simulink model "ScaraRobotApresentacao2023"  (R2024a)
(part 6 of 10)

et14 = -t2.*t4.*t8.*t9.*t63-t3.*t4.*t7.*t9.*t63-t2.*t4.*t8.*t9.*t68.*2.0-t3.*t4.*t7.*t9.*t68.*2.0-t2.*t4.*t8.*t9.*t69.*2.0-t3.*t4.*t7.*t9.*t69.*2.0+t2.*t4.*t8.*t9.*t70+t3.*t4.*t7.*t9.*t70+t2.*t4.*t8.*t9.*t71+t3.*t4.*t7.*t9.*t71-t2.*t4.*t8.*t9.*t72.*2.0-t3.*t4.*t7.*t9.*t72.*2.0-t2.*t4.*t8.*t9.*t73.*2.0-t3.*t4.*t7.*t9.*t73.*2.0+t2.*t4.*t8.*t9.*t74+t3.*t4.*t7.*t9.*t74+t2.*t4.*t8.*t9.*t75+t3.*t4.*t7.*t9.*t75+t2.*t4.*t8.*t9.*t95+t3.*t4.*t7.*t9.*t95+t2.*t4.*t8.*t9.*t97+t3.*t4.*t7.*t9.*t97+t2.*t4.*t8.*t9.*t101+t3.*t4.*t7.*t9.*t101+t2.*t4.*t8.*t9.*t103+t3.*t4.*t7.*t9.*t103-t3.*t4.*t7.*t9.*t126.*4.0+t3.*t4.*t7.*t9.*t130.*4.0+t3.*t4.*t7.*t9.*t134.*4.0;
et15 = t3.*t4.*t7.*t9.*t136.*4.0-t2.*t4.*t8.*t9.*t142.*2.0-t3.*t4.*t7.*t9.*t142.*2.0-t2.*t4.*t8.*t9.*t143.*2.0-t3.*t4.*t7.*t9.*t143.*2.0-t2.*t4.*t8.*t9.*t144.*2.0-t3.*t4.*t7.*t9.*t144.*2.0-t2.*t4.*t8.*t9.*t145.*2.0-t3.*t4.*t7.*t9.*t145.*2.0-t3.*t4.*t7.*t9.*t148.*4.0-t3.*t4.*t7.*t9.*t150.*4.0-t2.*t4.*t8.*t9.*t154.*2.0-t3.*t4.*t7.*t9.*t154.*2.0-t2.*t4.*t8.*t9.*t155.*2.0-t3.*t4.*t7.*t9.*t155.*2.0-t2.*t4.*t8.*t9.*t156.*2.0-t3.*t4.*t7.*t9.*t156.*2.0-t2.*t4.*t8.*t9.*t157.*2.0-t3.*t4.*t7.*t9.*t157.*2.0+t2.*t4.*t8.*t9.*t160+t3.*t4.*t7.*t9.*t160+t2.*t4.*t8.*t9.*t161+t3.*t4.*t7.*t9.*t161+t2.*t4.*t8.*t9.*t164+t3.*t4.*t7.*t9.*t164+t2.*t4.*t8.*t9.*t165+t3.*t4.*t7.*t9.*t165;
et16 = t2.*t4.*t8.*t9.*t183+t3.*t4.*t7.*t9.*t183+t2.*t4.*t8.*t9.*t184+t3.*t4.*t7.*t9.*t184+t2.*t4.*t8.*t9.*t187+t3.*t4.*t7.*t9.*t187+t2.*t4.*t8.*t9.*t188+t3.*t4.*t7.*t9.*t188+t3.*t4.*t7.*t9.*t239.*4.0-t3.*t4.*t7.*t9.*t243.*4.0+t3.*t4.*t7.*t9.*t246.*2.0-t2.*t4.*t8.*t9.*t250-t3.*t4.*t7.*t9.*t250-t2.*t4.*t8.*t9.*t251-t3.*t4.*t7.*t9.*t251+t3.*t4.*t7.*t9.*t254.*2.0-t2.*t4.*t8.*t9.*t258-t3.*t4.*t7.*t9.*t258-t2.*t4.*t8.*t9.*t259-t3.*t4.*t7.*t9.*t259-t3.*t4.*t7.*t9.*t265.*2.0+t3.*t4.*t7.*t9.*t267.*2.0-t2.*t4.*t8.*t9.*t276-t3.*t4.*t7.*t9.*t276-t2.*t4.*t8.*t9.*t277-t3.*t4.*t7.*t9.*t277-t3.*t4.*t7.*t9.*t278.*2.0;
et17 = t3.*t4.*t7.*t9.*t280.*2.0-t2.*t4.*t8.*t9.*t289-t3.*t4.*t7.*t9.*t289-t2.*t4.*t8.*t9.*t290-t3.*t4.*t7.*t9.*t290+t2.*t4.*t8.*t9.*t336+t3.*t4.*t7.*t9.*t336+t2.*t4.*t8.*t9.*t337+t3.*t4.*t7.*t9.*t337+t2.*t4.*t8.*t9.*t345+t3.*t4.*t7.*t9.*t345+t2.*t4.*t8.*t9.*t346+t3.*t4.*t7.*t9.*t346+t2.*t4.*t8.*t9.*t350+t3.*t4.*t7.*t9.*t350+t2.*t4.*t8.*t9.*t352+t3.*t4.*t7.*t9.*t352+t2.*t4.*t8.*t9.*t355+t3.*t4.*t7.*t9.*t355+t2.*t4.*t8.*t9.*t356+t3.*t4.*t7.*t9.*t356+t3.*t4.*t7.*t9.*t502.*2.0+t3.*t4.*t7.*t9.*t508.*2.0+t3.*t4.*t7.*t9.*t520.*2.0+t3.*t4.*t7.*t9.*t533.*2.0+t2.*t4.*t8.*t9.*t766+t3.*t4.*t7.*t9.*t766+t2.*t4.*t8.*t9.*t767+t3.*t4.*t7.*t9.*t767+t2.*t4.*t8.*t9.*t770+t3.*t4.*t7.*t9.*t770;
et18 = t2.*t4.*t8.*t9.*t771+t3.*t4.*t7.*t9.*t771+t2.*t4.*t8.*t9.*t784+t3.*t4.*t7.*t9.*t784+t2.*t4.*t8.*t9.*t786+t3.*t4.*t7.*t9.*t786+t2.*t4.*t8.*t9.*t787+t3.*t4.*t7.*t9.*t787+t2.*t4.*t8.*t9.*t790+t3.*t4.*t7.*t9.*t790+t2.*t4.*t8.*t9.*t1100+t3.*t4.*t7.*t9.*t1100+t2.*t4.*t8.*t9.*t1101+t3.*t4.*t7.*t9.*t1101+t2.*t4.*t8.*t9.*t1489+t3.*t4.*t7.*t9.*t1489+t2.*t4.*t8.*t9.*t1491+t3.*t4.*t7.*t9.*t1491+t2.*t4.*t8.*t9.*t1492+t3.*t4.*t7.*t9.*t1492+t2.*t4.*t8.*t9.*t1495+t3.*t4.*t7.*t9.*t1495-Lxcm2.^2.*dQ1.*dQ2.*m2.*t37+Lzcm2.^2.*dQ1.*dQ2.*m2.*t37+t2.*t3.*t5.*t9.*t10.*t44.*2.0+t2.*t3.*t5.*t9.*t10.*t45.*2.0+t2.*t3.*t5.*t9.*t10.*t48.*2.0+t2.*t3.*t5.*t9.*t10.*t49.*2.0-t5.*t7.*t8.*t9.*t10.*t44.*2.0+t2.*t3.*t5.*t9.*t10.*t55.*2.0;
et19 = t5.*t7.*t8.*t9.*t10.*t45.*-2.0+t2.*t3.*t5.*t9.*t10.*t56.*2.0-t2.*t5.*t6.*t8.*t11.*t54.*2.0-t3.*t5.*t6.*t7.*t11.*t54.*2.0-t5.*t7.*t8.*t9.*t10.*t48.*2.0-t5.*t7.*t8.*t9.*t10.*t49.*2.0+t2.*t3.*t5.*t9.*t10.*t62.*2.0+t2.*t3.*t5.*t9.*t10.*t63.*2.0-t2.*t5.*t6.*t8.*t11.*t61.*2.0-t3.*t5.*t6.*t7.*t11.*t61.*2.0-t5.*t7.*t8.*t9.*t10.*t55.*2.0-t5.*t7.*t8.*t9.*t10.*t56.*2.0-t2.*t3.*t5.*t9.*t10.*t70.*2.0-t2.*t3.*t5.*t9.*t10.*t71.*2.0-t5.*t7.*t8.*t9.*t10.*t62.*2.0-t5.*t7.*t8.*t9.*t10.*t63.*2.0-t2.*t3.*t5.*t9.*t10.*t74.*2.0-t2.*t3.*t5.*t9.*t10.*t75.*2.0+t5.*t7.*t8.*t9.*t10.*t70.*2.0+t5.*t7.*t8.*t9.*t10.*t71.*2.0-t2.*t4.*t8.*t9.*t36.*t52.*4.0-t3.*t4.*t7.*t9.*t36.*t52.*4.0;
et20 = t2.*t4.*t8.*t9.*t36.*t53.*-4.0-t3.*t4.*t7.*t9.*t36.*t53.*4.0+t5.*t7.*t8.*t9.*t10.*t74.*2.0+t5.*t7.*t8.*t9.*t10.*t75.*2.0-t2.*t4.*t8.*t9.*t36.*t59.*4.0-t3.*t4.*t7.*t9.*t36.*t59.*4.0-t2.*t4.*t8.*t9.*t36.*t60.*4.0-t3.*t4.*t7.*t9.*t36.*t60.*4.0-t2.*t5.*t6.*t8.*t11.*t94.*4.0-t3.*t5.*t6.*t7.*t11.*t94.*4.0-t2.*t4.*t8.*t9.*t35.*t70.*2.0-t2.*t5.*t6.*t8.*t11.*t96.*4.0-t3.*t4.*t7.*t9.*t35.*t70.*2.0-t3.*t5.*t6.*t7.*t11.*t96.*4.0-t2.*t4.*t8.*t9.*t35.*t71.*2.0-t3.*t4.*t7.*t9.*t35.*t71.*2.0-t2.*t4.*t8.*t9.*t35.*t74.*2.0-t2.*t5.*t6.*t8.*t11.*t100.*4.0-t3.*t4.*t7.*t9.*t35.*t74.*2.0-t3.*t5.*t6.*t7.*t11.*t100.*4.0-t2.*t4.*t8.*t9.*t35.*t75.*2.0-t3.*t4.*t7.*t9.*t35.*t75.*2.0;
et21 = t2.*t5.*t6.*t8.*t11.*t102.*-4.0-t3.*t5.*t6.*t7.*t11.*t102.*4.0-t2.*t4.*t8.*t9.*t36.*t95.*2.0-t3.*t4.*t7.*t9.*t36.*t95.*2.0-t2.*t4.*t8.*t9.*t36.*t97.*2.0-t3.*t4.*t7.*t9.*t36.*t97.*2.0-t2.*t4.*t8.*t9.*t36.*t101.*2.0-t3.*t4.*t7.*t9.*t36.*t101.*2.0-t2.*t4.*t8.*t9.*t36.*t103.*2.0-t3.*t4.*t7.*t9.*t36.*t103.*2.0+t3.*t5.*t6.*t7.*t11.*t130.*4.0-t2.*t5.*t6.*t8.*t11.*t132.*2.0-t3.*t5.*t6.*t7.*t11.*t132.*2.0-t3.*t5.*t6.*t7.*t11.*t138.*4.0+t2.*t5.*t6.*t8.*t11.*t140.*2.0+t3.*t5.*t6.*t7.*t11.*t140.*2.0-t3.*t4.*t7.*t9.*t35.*t128.*4.0-t3.*t4.*t7.*t9.*t36.*t130.*4.0-t3.*t4.*t7.*t9.*t35.*t138.*4.0+t3.*t4.*t7.*t9.*t36.*t138.*4.0+t3.*t4.*t7.*t9.*t35.*t148.*4.0+t3.*t4.*t7.*t9.*t35.*t150.*4.0+t5.*t7.*t8.*t9.*t10.*t222.*4.0;
et22 = t5.*t7.*t8.*t9.*t10.*t225.*4.0-t3.*t4.*t7.*t9.*t36.*t239.*8.0-t3.*t5.*t6.*t7.*t11.*t267.*4.0+t3.*t4.*t7.*t9.*t36.*t243.*8.0+t2.*t5.*t6.*t8.*t11.*t271.*2.0+t3.*t5.*t6.*t7.*t11.*t271.*2.0+t2.*t5.*t6.*t8.*t11.*t272.*2.0+t3.*t5.*t6.*t7.*t11.*t272.*2.0-t3.*t5.*t6.*t7.*t11.*t280.*4.0+t2.*t5.*t6.*t8.*t11.*t284.*2.0+t3.*t5.*t6.*t7.*t11.*t284.*2.0+t2.*t5.*t6.*t8.*t11.*t285.*2.0+t3.*t5.*t6.*t7.*t11.*t285.*2.0-t3.*t4.*t7.*t9.*t36.*t267.*4.0-t3.*t4.*t7.*t9.*t36.*t280.*4.0+t5.*t7.*t8.*t9.*t10.*t485.*4.0+t5.*t7.*t8.*t9.*t10.*t486.*4.0-t5.*t7.*t8.*t9.*t10.*t501.*4.0-t5.*t7.*t8.*t9.*t10.*t507.*4.0-t3.*t5.*t6.*t7.*t11.*t515.*8.0-t3.*t5.*t6.*t7.*t11.*t528.*8.0-t3.*t5.*t6.*t7.*t11.*t978.*4.0-t3.*t5.*t6.*t7.*t11.*t984.*4.0;
et23 = Lx2.*Lx3.*dQ1.*dQ2.*m4.*t8.*2.0+Lx2.*Lx3.*dQ1.*dQ2.*m5.*t8.*2.0+Lx2.*Lx3.*dQ1.*dQ2.*m6.*t8.*2.0+Lx2.*Lxcm3.*dQ1.*dQ2.*m3.*t8.*2.0-Lx3.*Lxcm4.*dQ1.*dQ4.*m4.*t9.*2.0-Lx3.*Lxcm5.*dQ1.*dQ2.*m5.*t10.*2.0-Lx3.*Lxcm5.*dQ1.*dQ3.*m5.*t10.*2.0-Lx3.*Lycm4.*dQ1.*dQ4.*m4.*t4.*2.0-Lx3.*Lycm5.*dQ1.*dQ4.*m5.*t4.*2.0-Lxcm4.*Lycm4.*dQ1.*dQ4.*m4.*t32.*2.0-Lxcm4.*Lycm4.*dQ1.*dQ4.*m4.*t33.*2.0+Lxcm6.*Lycm6.*dQ1.*dQ6.*m6.*t32.*4.0+Lxcm6.*Lycm6.*dQ1.*dQ6.*m6.*t33.*4.0+Lxcm6.*Lycm6.*dQ1.*dQ6.*m6.*t35.*2.0+Lxcm6.*Lycm6.*dQ1.*dQ6.*m6.*t36.*4.0-Lx2.*Lz4.*dQ1.*dQ2.*m5.*t3.*2.0-Lx2.*Lz4.*dQ1.*dQ2.*m6.*t3.*2.0+Lx3.*Lz5.*dQ1.*dQ2.*m6.*t5.*2.0+Lx3.*Lz5.*dQ1.*dQ3.*m6.*t5.*2.0-Lx3.*Lz4.*dQ1.*dQ2.*m5.*t32.*4.0-Lx3.*Lz4.*dQ1.*dQ2.*m5.*t33.*4.0-Lx3.*Lz4.*dQ1.*dQ2.*m6.*t32.*4.0-Lx3.*Lz4.*dQ1.*dQ3.*m5.*t32.*4.0;
et24 = Lx3.*Lz4.*dQ1.*dQ2.*m6.*t33.*-4.0-Lx3.*Lz4.*dQ1.*dQ3.*m5.*t33.*4.0-Lx3.*Lz4.*dQ1.*dQ3.*m6.*t32.*4.0-Lx3.*Lz4.*dQ1.*dQ3.*m6.*t33.*4.0-Lx2.*Lzcm3.*dQ1.*dQ2.*m3.*t3.*2.0-Lx2.*Lzcm4.*dQ1.*dQ2.*m4.*t3.*2.0+Lx3.*Lzcm5.*dQ1.*dQ2.*m5.*t5.*2.0+Lx3.*Lzcm5.*dQ1.*dQ3.*m5.*t5.*2.0+Lx3.*Lzcm6.*dQ1.*dQ2.*m6.*t5.*2.0+Lx3.*Lzcm6.*dQ1.*dQ3.*m6.*t5.*2.0-Lxcm6.*Lz5.*dQ1.*dQ5.*m6.*t6.*2.0-Lx3.*Lzcm4.*dQ1.*dQ2.*m4.*t32.*4.0-Lx3.*Lzcm4.*dQ1.*dQ2.*m4.*t33.*4.0-Lx3.*Lzcm4.*dQ1.*dQ3.*m4.*t32.*4.0-Lx3.*Lzcm4.*dQ1.*dQ3.*m4.*t33.*4.0+Lxcm4.*Lzcm4.*dQ1.*dQ2.*m4.*t4.*2.0+Lxcm4.*Lzcm4.*dQ1.*dQ3.*m4.*t4.*2.0-Lxcm5.*Lzcm5.*dQ1.*dQ2.*m5.*t4.*2.0-Lxcm5.*Lzcm5.*dQ1.*dQ3.*m5.*t4.*2.0-Lxcm6.*Lzcm6.*dQ1.*dQ5.*m6.*t6.*2.0+Lxcm2.*Lzcm2.*dQ1.*dQ2.*m2.*t32.*4.0-Lxcm3.*Lzcm3.*dQ1.*dQ2.*m3.*t32.*4.0-Lxcm3.*Lzcm3.*dQ1.*dQ2.*m3.*t33.*4.0;
et25 = Lxcm3.*Lzcm3.*dQ1.*dQ3.*m3.*t32.*-4.0-Lxcm3.*Lzcm3.*dQ1.*dQ3.*m3.*t33.*4.0+Lxcm5.*Lzcm5.*dQ1.*dQ5.*m5.*t32.*2.0+Lxcm5.*Lzcm5.*dQ1.*dQ5.*m5.*t33.*2.0+Lxcm5.*Lzcm5.*dQ1.*dQ5.*m5.*t35.*4.0-Lycm5.*Lz4.*dQ1.*dQ2.*m5.*t9.*2.0-Lycm5.*Lz4.*dQ1.*dQ3.*m5.*t9.*2.0+Lycm6.*Lz5.*dQ1.*dQ5.*m6.*t11.*2.0-Lycm4.*Lzcm4.*dQ1.*dQ2.*m4.*t9.*2.0-Lycm4.*Lzcm4.*dQ1.*dQ3.*m4.*t9.*2.0+Lycm6.*Lzcm6.*dQ1.*dQ5.*m6.*t11.*2.0+Lz5.*Lzcm6.*dQ1.*dQ5.*m6.*t40.*2.0+Ixx5.*dQ1.*dQ5.*t2.*t4.*t7.*2.0+Ixx5.*dQ1.*dQ5.*t3.*t4.*t8.*2.0+Ixx5.*dQ2.*dQ5.*t2.*t3.*t9+Ixx5.*dQ1.*dQ2.*t4.*t5.*t10.*2.0+Ixx5.*dQ3.*dQ5.*t2.*t3.*t9+Ixx6.*dQ2.*dQ5.*t2.*t3.*t9+Ixx5.*dQ1.*dQ3.*t4.*t5.*t10.*2.0-Ixx5.*dQ4.*dQ5.*t2.*t4.*t8-Ixx5.*dQ4.*dQ5.*t3.*t4.*t7+Ixx6.*dQ3.*dQ5.*t2.*t3.*t9-Ixx6.*dQ2.*dQ6.*t2.*t5.*t8-Ixx6.*dQ2.*dQ6.*t3.*t5.*t7;
et26 = Ixx6.*dQ4.*dQ5.*t2.*t4.*t8+Ixx6.*dQ4.*dQ5.*t3.*t4.*t7-Ixx6.*dQ3.*dQ6.*t2.*t5.*t8-Ixx6.*dQ3.*dQ6.*t3.*t5.*t7+Ixx6.*dQ5.*dQ6.*t2.*t3.*t10-Ixx5.*dQ2.*dQ5.*t7.*t8.*t9-Ixx5.*dQ3.*dQ5.*t7.*t8.*t9-Ixx6.*dQ2.*dQ5.*t7.*t8.*t9-Ixx6.*dQ3.*dQ5.*t7.*t8.*t9-Ixx6.*dQ5.*dQ6.*t7.*t8.*t10+Ixx3.*dQ1.*dQ2.*t2.*t7.*t33.*4.0+Ixx3.*dQ1.*dQ2.*t3.*t8.*t32.*4.0+Ixx3.*dQ1.*dQ3.*t2.*t7.*t33.*4.0+Ixx3.*dQ1.*dQ3.*t3.*t8.*t32.*4.0-Ixx4.*dQ1.*dQ2.*t2.*t7.*t34.*2.0-Ixx5.*dQ1.*dQ2.*t2.*t7.*t33.*4.0-Ixx4.*dQ1.*dQ3.*t2.*t7.*t34.*2.0-Ixx5.*dQ1.*dQ2.*t3.*t8.*t32.*4.0-Ixx5.*dQ1.*dQ3.*t2.*t7.*t33.*4.0+Ixx6.*dQ1.*dQ2.*t2.*t7.*t33.*4.0-Ixx4.*dQ1.*dQ2.*t3.*t8.*t34.*2.0-Ixx5.*dQ1.*dQ2.*t2.*t7.*t35.*2.0-Ixx5.*dQ1.*dQ3.*t3.*t8.*t32.*4.0;
et27 = Ixx6.*dQ1.*dQ2.*t2.*t7.*t34.*2.0+Ixx6.*dQ1.*dQ2.*t3.*t8.*t32.*4.0+Ixx6.*dQ1.*dQ3.*t2.*t7.*t33.*4.0-Ixx4.*dQ1.*dQ3.*t3.*t8.*t34.*2.0-Ixx5.*dQ1.*dQ3.*t2.*t7.*t35.*2.0+Ixx6.*dQ1.*dQ3.*t2.*t7.*t34.*2.0+Ixx6.*dQ1.*dQ3.*t3.*t8.*t32.*4.0-Ixx4.*dQ1.*dQ4.*t4.*t9.*t32.*2.0-Ixx4.*dQ2.*dQ4.*t2.*t8.*t34.*2.0-Ixx4.*dQ2.*dQ4.*t3.*t7.*t34.*2.0-Ixx5.*dQ1.*dQ2.*t3.*t8.*t35.*2.0+Ixx6.*dQ1.*dQ2.*t2.*t7.*t36.*4.0+Ixx6.*dQ1.*dQ2.*t3.*t8.*t34.*2.0-Ixx4.*dQ1.*dQ4.*t4.*t9.*t33.*2.0-Ixx4.*dQ3.*dQ4.*t2.*t8.*t34.*2.0-Ixx4.*dQ3.*dQ4.*t3.*t7.*t34.*2.0-Ixx5.*dQ1.*dQ3.*t3.*t8.*t35.*2.0+Ixx6.*dQ1.*dQ3.*t2.*t7.*t36.*4.0+Ixx6.*dQ1.*dQ3.*t3.*t8.*t34.*2.0+Ixx5.*dQ2.*dQ4.*t2.*t8.*t35.*2.0+Ixx5.*dQ2.*dQ4.*t3.*t7.*t35.*2.0+Ixx6.*dQ1.*dQ2.*t3.*t8.*t36.*4.0+Ixx6.*dQ1.*dQ4.*t4.*t9.*t32.*2.0;
et28 = Ixx6.*dQ2.*dQ4.*t2.*t8.*t34.*2.0+Ixx6.*dQ2.*dQ4.*t3.*t7.*t34.*2.0+Ixx5.*dQ3.*dQ4.*t2.*t8.*t35.*2.0+Ixx5.*dQ3.*dQ4.*t3.*t7.*t35.*2.0+Ixx6.*dQ1.*dQ3.*t3.*t8.*t36.*4.0+Ixx6.*dQ1.*dQ4.*t4.*t9.*t33.*2.0+Ixx6.*dQ3.*dQ4.*t2.*t8.*t34.*2.0+Ixx6.*dQ3.*dQ4.*t3.*t7.*t34.*2.0-Ixx5.*dQ1.*dQ5.*t5.*t10.*t32.*2.0-Ixx5.*dQ1.*dQ5.*t5.*t10.*t33.*2.0+Ixx6.*dQ1.*dQ6.*t6.*t11.*t32.*4.0+Ixx6.*dQ1.*dQ5.*t5.*t10.*t36.*2.0+Ixx6.*dQ1.*dQ6.*t6.*t11.*t33.*4.0+Ixx6.*dQ1.*dQ6.*t6.*t11.*t35.*2.0-Ixy5.*dQ2.*dQ3.*t2.*t3.*t5+Ixy6.*dQ2.*dQ3.*t2.*t3.*t5+Ixy5.*dQ2.*dQ3.*t5.*t7.*t8-Ixy6.*dQ2.*dQ3.*t5.*t7.*t8+Ixy6.*dQ5.*dQ6.*t2.*t8.*t9+Ixy6.*dQ5.*dQ6.*t3.*t7.*t9+Ixy4.*dQ2.*dQ3.*t2.*t3.*t34.*2.0+Ixy6.*dQ4.*dQ6.*t2.*t3.*t35+Ixy6.*dQ4.*dQ6.*t2.*t3.*t36.*2.0-Ixy4.*dQ2.*dQ3.*t7.*t8.*t34.*2.0;
et29 = Ixy5.*dQ1.*dQ2.*t9.*t10.*t32.*-2.0-Ixy5.*dQ1.*dQ2.*t9.*t10.*t33.*2.0-Ixy5.*dQ1.*dQ3.*t9.*t10.*t32.*2.0+Ixy6.*dQ1.*dQ2.*t9.*t10.*t32.*2.0-Ixy5.*dQ1.*dQ3.*t9.*t10.*t33.*2.0+Ixy6.*dQ1.*dQ2.*t9.*t10.*t33.*2.0+Ixy6.*dQ1.*dQ3.*t9.*t10.*t32.*2.0+Ixy6.*dQ1.*dQ3.*t9.*t10.*t33.*2.0+Ixy6.*dQ1.*dQ2.*t9.*t10.*t36.*2.0+Ixy6.*dQ1.*dQ3.*t9.*t10.*t36.*2.0-Ixy6.*dQ4.*dQ6.*t7.*t8.*t35-Ixy6.*dQ4.*dQ6.*t7.*t8.*t36.*2.0+Ixy5.*dQ1.*dQ4.*t5.*t32.*t33.*2.0+Ixy5.*dQ1.*dQ4.*t5.*t32.*t34.*2.0-Ixy6.*dQ1.*dQ4.*t5.*t32.*t33.*2.0+Ixy5.*dQ1.*dQ4.*t5.*t33.*t34.*2.0-Ixy6.*dQ1.*dQ4.*t5.*t32.*t34.*2.0-Ixy6.*dQ1.*dQ4.*t5.*t33.*t34.*2.0-Ixy6.*dQ1.*dQ4.*t5.*t32.*t36.*2.0-Ixy6.*dQ1.*dQ4.*t5.*t33.*t36.*2.0-Ixy4.*dQ1.*dQ4.*t32.*t33.*t34.*4.0+Ixy6.*dQ1.*dQ6.*t32.*t33.*t34.*2.0+Ixy6.*dQ1.*dQ6.*t32.*t33.*t35.*2.0;
et30 = Ixy6.*dQ1.*dQ6.*t32.*t33.*t36.*8.0-Ixy6.*dQ1.*dQ6.*t32.*t34.*t35+Ixy6.*dQ1.*dQ6.*t32.*t34.*t36.*2.0-Ixy6.*dQ1.*dQ6.*t33.*t34.*t35+Ixy6.*dQ1.*dQ6.*t32.*t35.*t36.*2.0+Ixy6.*dQ1.*dQ6.*t33.*t34.*t36.*2.0+Ixy6.*dQ1.*dQ6.*t33.*t35.*t36.*2.0-Ixz6.*dQ4.*dQ5.*t2.*t3.*t6+Ixz4.*dQ1.*dQ4.*t2.*t7.*t9+Ixz4.*dQ2.*dQ3.*t2.*t8.*t9+Ixz4.*dQ2.*dQ3.*t3.*t7.*t9-Ixz5.*dQ1.*dQ4.*t2.*t7.*t9+Ixz4.*dQ1.*dQ4.*t3.*t8.*t9-Ixz5.*dQ2.*dQ3.*t2.*t8.*t9-Ixz5.*dQ2.*dQ3.*t3.*t7.*t9-Ixz5.*dQ1.*dQ4.*t3.*t8.*t9-Ixz6.*dQ1.*dQ2.*t5.*t9.*t11-Ixz6.*dQ1.*dQ3.*t5.*t9.*t11+Ixz6.*dQ4.*dQ5.*t6.*t7.*t8-Ixz6.*dQ1.*dQ6.*t5.*t10.*t11+Ixz6.*dQ1.*dQ2.*t4.*t6.*t32.*2.0+Ixz6.*dQ1.*dQ2.*t4.*t6.*t33.*2.0+Ixz6.*dQ1.*dQ3.*t4.*t6.*t32.*2.0+Ixz6.*dQ1.*dQ3.*t4.*t6.*t33.*2.0;
et31 = Ixz5.*dQ4.*dQ5.*t2.*t3.*t35.*2.0+Ixz6.*dQ1.*dQ2.*t4.*t6.*t35.*2.0+Ixz6.*dQ1.*dQ3.*t4.*t6.*t35.*2.0-Ixz5.*dQ4.*dQ5.*t7.*t8.*t35.*2.0-Ixz6.*dQ1.*dQ4.*t10.*t11.*t32-Ixz6.*dQ1.*dQ4.*t10.*t11.*t33+Ixz4.*dQ1.*dQ2.*t4.*t32.*t33.*4.0+Ixz4.*dQ1.*dQ3.*t4.*t32.*t33.*4.0-Ixz5.*dQ1.*dQ2.*t4.*t32.*t33.*4.0-Ixz5.*dQ1.*dQ3.*t4.*t32.*t33.*4.0-Ixz5.*dQ1.*dQ2.*t4.*t32.*t35.*4.0-Ixz5.*dQ1.*dQ2.*t4.*t33.*t35.*4.0-Ixz5.*dQ1.*dQ3.*t4.*t32.*t35.*4.0-Ixz5.*dQ1.*dQ3.*t4.*t33.*t35.*4.0-Ixz6.*dQ1.*dQ5.*t6.*t32.*t33.*2.0+Ixz6.*dQ1.*dQ5.*t6.*t32.*t34-Ixz6.*dQ1.*dQ5.*t6.*t32.*t35.*2.0+Ixz6.*dQ1.*dQ5.*t6.*t33.*t34-Ixz6.*dQ1.*dQ5.*t6.*t33.*t35.*2.0-Ixz5.*dQ1.*dQ5.*t32.*t33.*t34.*2.0+Ixz5.*dQ1.*dQ5.*t32.*t33.*t35.*4.0-Ixz5.*dQ1.*dQ5.*t32.*t34.*t35.*2.0-Ixz5.*dQ1.*dQ5.*t33.*t34.*t35.*2.0;
et32 = -Iyx5.*dQ2.*dQ3.*t2.*t3.*t5+Iyx6.*dQ2.*dQ3.*t2.*t3.*t5+Iyx5.*dQ2.*dQ3.*t5.*t7.*t8-Iyx6.*dQ2.*dQ3.*t5.*t7.*t8+Iyx6.*dQ5.*dQ6.*t2.*t8.*t9+Iyx6.*dQ5.*dQ6.*t3.*t7.*t9+Iyx4.*dQ2.*dQ3.*t2.*t3.*t34.*2.0+Iyx6.*dQ4.*dQ6.*t2.*t3.*t35+Iyx6.*dQ4.*dQ6.*t2.*t3.*t36.*2.0-Iyx4.*dQ2.*dQ3.*t7.*t8.*t34.*2.0-Iyx5.*dQ1.*dQ2.*t9.*t10.*t32.*2.0-Iyx5.*dQ1.*dQ2.*t9.*t10.*t33.*2.0-Iyx5.*dQ1.*dQ3.*t9.*t10.*t32.*2.0+Iyx6.*dQ1.*dQ2.*t9.*t10.*t32.*2.0-Iyx5.*dQ1.*dQ3.*t9.*t10.*t33.*2.0+Iyx6.*dQ1.*dQ2.*t9.*t10.*t33.*2.0+Iyx6.*dQ1.*dQ3.*t9.*t10.*t32.*2.0+Iyx6.*dQ1.*dQ3.*t9.*t10.*t33.*2.0+Iyx6.*dQ1.*dQ2.*t9.*t10.*t36.*2.0+Iyx6.*dQ1.*dQ3.*t9.*t10.*t36.*2.0-Iyx6.*dQ4.*dQ6.*t7.*t8.*t35-Iyx6.*dQ4.*dQ6.*t7.*t8.*t36.*2.0+Iyx5.*dQ1.*dQ4.*t5.*t32.*t33.*2.0+Iyx5.*dQ1.*dQ4.*t5.*t32.*t34.*2.0;
et33 = Iyx6.*dQ1.*dQ4.*t5.*t32.*t33.*-2.0+Iyx5.*dQ1.*dQ4.*t5.*t33.*t34.*2.0-Iyx6.*dQ1.*dQ4.*t5.*t32.*t34.*2.0-Iyx6.*dQ1.*dQ4.*t5.*t33.*t34.*2.0-Iyx6.*dQ1.*dQ4.*t5.*t32.*t36.*2.0-Iyx6.*dQ1.*dQ4.*t5.*t33.*t36.*2.0-Iyx4.*dQ1.*dQ4.*t32.*t33.*t34.*4.0+Iyx6.*dQ1.*dQ6.*t32.*t33.*t34.*2.0+Iyx6.*dQ1.*dQ6.*t32.*t33.*t35.*2.0+Iyx6.*dQ1.*dQ6.*t32.*t33.*t36.*8.0-Iyx6.*dQ1.*dQ6.*t32.*t34.*t35+Iyx6.*dQ1.*dQ6.*t32.*t34.*t36.*2.0-Iyx6.*dQ1.*dQ6.*t33.*t34.*t35+Iyx6.*dQ1.*dQ6.*t32.*t35.*t36.*2.0+Iyx6.*dQ1.*dQ6.*t33.*t34.*t36.*2.0+Iyx6.*dQ1.*dQ6.*t33.*t35.*t36.*2.0+Iyy6.*dQ1.*dQ5.*t2.*t4.*t7.*2.0+Iyy5.*dQ2.*dQ5.*t2.*t3.*t9+Iyy5.*dQ3.*dQ5.*t2.*t3.*t9+Iyy6.*dQ1.*dQ5.*t3.*t4.*t8.*2.0+Iyy6.*dQ2.*dQ5.*t2.*t3.*t9+Iyy5.*dQ4.*dQ5.*t2.*t4.*t8+Iyy5.*dQ4.*dQ5.*t3.*t4.*t7+Iyy6.*dQ1.*dQ2.*t4.*t5.*t10.*2.0;
et34 = Iyy6.*dQ3.*dQ5.*t2.*t3.*t9+Iyy6.*dQ1.*dQ3.*t4.*t5.*t10.*2.0+Iyy6.*dQ2.*dQ6.*t2.*t5.*t8+Iyy6.*dQ2.*dQ6.*t3.*t5.*t7-Iyy6.*dQ4.*dQ5.*t2.*t4.*t8-Iyy6.*dQ4.*dQ5.*t3.*t4.*t7+Iyy6.*dQ3.*dQ6.*t2.*t5.*t8+Iyy6.*dQ3.*dQ6.*t3.*t5.*t7-Iyy6.*dQ5.*dQ6.*t2.*t3.*t10-Iyy5.*dQ2.*dQ5.*t7.*t8.*t9-Iyy5.*dQ3.*dQ5.*t7.*t8.*t9-Iyy6.*dQ2.*dQ5.*t7.*t8.*t9-Iyy6.*dQ3.*dQ5.*t7.*t8.*t9+Iyy6.*dQ5.*dQ6.*t7.*t8.*t10+Iyy4.*dQ1.*dQ2.*t2.*t7.*t33.*4.0+Iyy4.*dQ1.*dQ2.*t2.*t7.*t34.*2.0+Iyy4.*dQ1.*dQ2.*t3.*t8.*t32.*4.0+Iyy4.*dQ1.*dQ3.*t2.*t7.*t33.*4.0+Iyy5.*dQ1.*dQ2.*t2.*t7.*t33.*4.0+Iyy4.*dQ1.*dQ3.*t2.*t7.*t34.*2.0+Iyy4.*dQ1.*dQ3.*t3.*t8.*t32.*4.0+Iyy5.*dQ1.*dQ2.*t2.*t7.*t34.*2.0+Iyy5.*dQ1.*dQ2.*t3.*t8.*t32.*4.0+Iyy5.*dQ1.*dQ3.*t2.*t7.*t33.*4.0;
et35 = Iyy6.*dQ1.*dQ2.*t2.*t7.*t33.*-4.0+Iyy4.*dQ1.*dQ2.*t3.*t8.*t34.*2.0+Iyy5.*dQ1.*dQ3.*t2.*t7.*t34.*2.0+Iyy5.*dQ1.*dQ3.*t3.*t8.*t32.*4.0-Iyy6.*dQ1.*dQ2.*t3.*t8.*t32.*4.0-Iyy6.*dQ1.*dQ3.*t2.*t7.*t33.*4.0+Iyy4.*dQ1.*dQ3.*t3.*t8.*t34.*2.0+Iyy5.*dQ1.*dQ2.*t3.*t8.*t34.*2.0-Iyy6.*dQ1.*dQ2.*t2.*t7.*t35.*2.0-Iyy6.*dQ1.*dQ3.*t3.*t8.*t32.*4.0+Iyy4.*dQ1.*dQ4.*t4.*t9.*t32.*2.0+Iyy4.*dQ2.*dQ4.*t2.*t8.*t34.*2.0+Iyy4.*dQ2.*dQ4.*t3.*t7.*t34.*2.0+Iyy5.*dQ1.*dQ3.*t3.*t8.*t34.*2.0-Iyy6.*dQ1.*dQ2.*t2.*t7.*t36.*4.0-Iyy6.*dQ1.*dQ3.*t2.*t7.*t35.*2.0+Iyy4.*dQ1.*dQ4.*t4.*t9.*t33.*2.0+Iyy4.*dQ3.*dQ4.*t2.*t8.*t34.*2.0+Iyy4.*dQ3.*dQ4.*t3.*t7.*t34.*2.0+Iyy5.*dQ1.*dQ4.*t4.*t9.*t32.*2.0+Iyy5.*dQ2.*dQ4.*t2.*t8.*t34.*2.0+Iyy5.*dQ2.*dQ4.*t3.*t7.*t34.*2.0-Iyy6.*dQ1.*dQ2.*t3.*t8.*t35.*2.0;
et36 = Iyy6.*dQ1.*dQ3.*t2.*t7.*t36.*-4.0+Iyy5.*dQ1.*dQ4.*t4.*t9.*t33.*2.0+Iyy5.*dQ3.*dQ4.*t2.*t8.*t34.*2.0+Iyy5.*dQ3.*dQ4.*t3.*t7.*t34.*2.0-Iyy6.*dQ1.*dQ2.*t3.*t8.*t36.*4.0-Iyy6.*dQ1.*dQ3.*t3.*t8.*t35.*2.0-Iyy6.*dQ1.*dQ3.*t3.*t8.*t36.*4.0+Iyy6.*dQ2.*dQ4.*t2.*t8.*t35.*2.0+Iyy6.*dQ2.*dQ4.*t3.*t7.*t35.*2.0+Iyy6.*dQ3.*dQ4.*t2.*t8.*t35.*2.0+Iyy6.*dQ3.*dQ4.*t3.*t7.*t35.*2.0-Iyy6.*dQ1.*dQ5.*t5.*t10.*t32.*2.0-Iyy6.*dQ1.*dQ5.*t5.*t10.*t33.*2.0-Iyy6.*dQ1.*dQ6.*t6.*t11.*t32.*4.0-Iyy6.*dQ1.*dQ5.*t5.*t10.*t36.*2.0-Iyy6.*dQ1.*dQ6.*t6.*t11.*t33.*4.0-Iyy6.*dQ1.*dQ6.*t6.*t11.*t35.*2.0+Iyz4.*dQ1.*dQ4.*t2.*t4.*t7+Iyz4.*dQ2.*dQ3.*t2.*t4.*t8+Iyz4.*dQ2.*dQ3.*t3.*t4.*t7+Iyz4.*dQ1.*dQ4.*t3.*t4.*t8-Iyz5.*dQ2.*dQ3.*t2.*t3.*t10-Iyz6.*dQ1.*dQ2.*t5.*t6.*t9;
et37 = -Iyz6.*dQ1.*dQ3.*t5.*t6.*t9+Iyz6.*dQ4.*dQ5.*t2.*t3.*t11-Iyz6.*dQ1.*dQ6.*t5.*t6.*t10+Iyz5.*dQ2.*dQ3.*t7.*t8.*t10-Iyz6.*dQ4.*dQ5.*t7.*t8.*t11+Iyz5.*dQ1.*dQ2.*t5.*t9.*t32.*2.0+Iyz5.*dQ1.*dQ2.*t5.*t9.*t33.*2.0+Iyz5.*dQ1.*dQ3.*t5.*t9.*t32.*2.0+Iyz5.*dQ1.*dQ3.*t5.*t9.*t33.*2.0-Iyz6.*dQ1.*dQ2.*t4.*t11.*t32.*2.0-Iyz6.*dQ1.*dQ2.*t4.*t11.*t33.*2.0-Iyz6.*dQ1.*dQ3.*t4.*t11.*t32.*2.0-Iyz6.*dQ1.*dQ3.*t4.*t11.*t33.*2.0-Iyz6.*dQ1.*dQ2.*t4.*t11.*t35.*2.0-Iyz6.*dQ1.*dQ4.*t6.*t10.*t32-Iyz6.*dQ1.*dQ3.*t4.*t11.*t35.*2.0-Iyz6.*dQ1.*dQ4.*t6.*t10.*t33-Iyz4.*dQ1.*dQ2.*t9.*t32.*t33.*4.0-Iyz4.*dQ1.*dQ3.*t9.*t32.*t33.*4.0+Iyz5.*dQ1.*dQ4.*t10.*t32.*t33.*2.0+Iyz5.*dQ1.*dQ4.*t10.*t32.*t34.*2.0+Iyz5.*dQ1.*dQ4.*t10.*t33.*t34.*2.0+Iyz6.*dQ1.*dQ5.*t11.*t32.*t33.*2.0;
et38 = -Iyz6.*dQ1.*dQ5.*t11.*t32.*t34+Iyz6.*dQ1.*dQ5.*t11.*t32.*t35.*2.0-Iyz6.*dQ1.*dQ5.*t11.*t33.*t34+Iyz6.*dQ1.*dQ5.*t11.*t33.*t35.*2.0-Izx6.*dQ4.*dQ5.*t2.*t3.*t6+Izx4.*dQ1.*dQ4.*t2.*t7.*t9+Izx4.*dQ2.*dQ3.*t2.*t8.*t9+Izx4.*dQ2.*dQ3.*t3.*t7.*t9-Izx5.*dQ1.*dQ4.*t2.*t7.*t9+Izx4.*dQ1.*dQ4.*t3.*t8.*t9-Izx5.*dQ2.*dQ3.*t2.*t8.*t9-Izx5.*dQ2.*dQ3.*t3.*t7.*t9-Izx5.*dQ1.*dQ4.*t3.*t8.*t9-Izx6.*dQ1.*dQ2.*t5.*t9.*t11-Izx6.*dQ1.*dQ3.*t5.*t9.*t11+Izx6.*dQ4.*dQ5.*t6.*t7.*t8-Izx6.*dQ1.*dQ6.*t5.*t10.*t11+Izx6.*dQ1.*dQ2.*t4.*t6.*t32.*2.0+Izx6.*dQ1.*dQ2.*t4.*t6.*t33.*2.0+Izx6.*dQ1.*dQ3.*t4.*t6.*t32.*2.0+Izx6.*dQ1.*dQ3.*t4.*t6.*t33.*2.0+Izx5.*dQ4.*dQ5.*t2.*t3.*t35.*2.0+Izx6.*dQ1.*dQ2.*t4.*t6.*t35.*2.0+Izx6.*dQ1.*dQ3.*t4.*t6.*t35.*2.0;
et39 = Izx5.*dQ4.*dQ5.*t7.*t8.*t35.*-2.0-Izx6.*dQ1.*dQ4.*t10.*t11.*t32-Izx6.*dQ1.*dQ4.*t10.*t11.*t33+Izx4.*dQ1.*dQ2.*t4.*t32.*t33.*4.0+Izx4.*dQ1.*dQ3.*t4.*t32.*t33.*4.0-Izx5.*dQ1.*dQ2.*t4.*t32.*t33.*4.0-Izx5.*dQ1.*dQ3.*t4.*t32.*t33.*4.0-Izx5.*dQ1.*dQ2.*t4.*t32.*t35.*4.0-Izx5.*dQ1.*dQ2.*t4.*t33.*t35.*4.0-Izx5.*dQ1.*dQ3.*t4.*t32.*t35.*4.0-Izx5.*dQ1.*dQ3.*t4.*t33.*t35.*4.0-Izx6.*dQ1.*dQ5.*t6.*t32.*t33.*2.0+Izx6.*dQ1.*dQ5.*t6.*t32.*t34-Izx6.*dQ1.*dQ5.*t6.*t32.*t35.*2.0+Izx6.*dQ1.*dQ5.*t6.*t33.*t34-Izx6.*dQ1.*dQ5.*t6.*t33.*t35.*2.0-Izx5.*dQ1.*dQ5.*t32.*t33.*t34.*2.0+Izx5.*dQ1.*dQ5.*t32.*t33.*t35.*4.0-Izx5.*dQ1.*dQ5.*t32.*t34.*t35.*2.0-Izx5.*dQ1.*dQ5.*t33.*t34.*t35.*2.0+Izy4.*dQ1.*dQ4.*t2.*t4.*t7+Izy4.*dQ2.*dQ3.*t2.*t4.*t8+Izy4.*dQ2.*dQ3.*t3.*t4.*t7;
et40 = Izy4.*dQ1.*dQ4.*t3.*t4.*t8-Izy5.*dQ2.*dQ3.*t2.*t3.*t10-Izy6.*dQ1.*dQ2.*t5.*t6.*t9-Izy6.*dQ1.*dQ3.*t5.*t6.*t9+Izy6.*dQ4.*dQ5.*t2.*t3.*t11-Izy6.*dQ1.*dQ6.*t5.*t6.*t10+Izy5.*dQ2.*dQ3.*t7.*t8.*t10-Izy6.*dQ4.*dQ5.*t7.*t8.*t11+Izy5.*dQ1.*dQ2.*t5.*t9.*t32.*2.0+Izy5.*dQ1.*dQ2.*t5.*t9.*t33.*2.0+Izy5.*dQ1.*dQ3.*t5.*t9.*t32.*2.0+Izy5.*dQ1.*dQ3.*t5.*t9.*t33.*2.0-Izy6.*dQ1.*dQ2.*t4.*t11.*t32.*2.0-Izy6.*dQ1.*dQ2.*t4.*t11.*t33.*2.0-Izy6.*dQ1.*dQ3.*t4.*t11.*t32.*2.0-Izy6.*dQ1.*dQ3.*t4.*t11.*t33.*2.0-Izy6.*dQ1.*dQ2.*t4.*t11.*t35.*2.0-Izy6.*dQ1.*dQ4.*t6.*t10.*t32-Izy6.*dQ1.*dQ3.*t4.*t11.*t35.*2.0-Izy6.*dQ1.*dQ4.*t6.*t10.*t33-Izy4.*dQ1.*dQ2.*t9.*t32.*t33.*4.0-Izy4.*dQ1.*dQ3.*t9.*t32.*t33.*4.0+Izy5.*dQ1.*dQ4.*t10.*t32.*t33.*2.0;
et41 = Izy5.*dQ1.*dQ4.*t10.*t32.*t34.*2.0+Izy5.*dQ1.*dQ4.*t10.*t33.*t34.*2.0+Izy6.*dQ1.*dQ5.*t11.*t32.*t33.*2.0-Izy6.*dQ1.*dQ5.*t11.*t32.*t34+Izy6.*dQ1.*dQ5.*t11.*t32.*t35.*2.0-Izy6.*dQ1.*dQ5.*t11.*t33.*t34+Izy6.*dQ1.*dQ5.*t11.*t33.*t35.*2.0-Izz5.*dQ1.*dQ5.*t2.*t4.*t7.*2.0-Izz6.*dQ1.*dQ5.*t2.*t4.*t7.*2.0-Izz5.*dQ1.*dQ5.*t3.*t4.*t8.*2.0-Izz5.*dQ2.*dQ5.*t2.*t3.*t9-Izz5.*dQ1.*dQ2.*t4.*t5.*t10.*2.0-Izz5.*dQ3.*dQ5.*t2.*t3.*t9-Izz6.*dQ1.*dQ5.*t3.*t4.*t8.*2.0-Izz6.*dQ2.*dQ5.*t2.*t3.*t9-Izz5.*dQ1.*dQ3.*t4.*t5.*t10.*2.0+Izz5.*dQ4.*dQ5.*t2.*t4.*t8+Izz5.*dQ4.*dQ5.*t3.*t4.*t7-Izz6.*dQ1.*dQ2.*t4.*t5.*t10.*2.0-Izz6.*dQ3.*dQ5.*t2.*t3.*t9-Izz6.*dQ1.*dQ3.*t4.*t5.*t10.*2.0-Izz6.*dQ2.*dQ6.*t2.*t5.*t8-Izz6.*dQ2.*dQ6.*t3.*t5.*t7;
et42 = Izz6.*dQ4.*dQ5.*t2.*t4.*t8+Izz6.*dQ4.*dQ5.*t3.*t4.*t7-Izz6.*dQ3.*dQ6.*t2.*t5.*t8-Izz6.*dQ3.*dQ6.*t3.*t5.*t7-Izz6.*dQ5.*dQ6.*t2.*t3.*t10+Izz5.*dQ2.*dQ5.*t7.*t8.*t9+Izz5.*dQ3.*dQ5.*t7.*t8.*t9+Izz6.*dQ2.*dQ5.*t7.*t8.*t9+Izz6.*dQ3.*dQ5.*t7.*t8.*t9+Izz6.*dQ5.*dQ6.*t7.*t8.*t10-Izz3.*dQ1.*dQ2.*t2.*t7.*t33.*4.0-Izz3.*dQ1.*dQ2.*t3.*t8.*t32.*4.0-Izz3.*dQ1.*dQ3.*t2.*t7.*t33.*4.0-Izz4.*dQ1.*dQ2.*t2.*t7.*t33.*4.0-Izz3.*dQ1.*dQ3.*t3.*t8.*t32.*4.0-Izz4.*dQ1.*dQ2.*t3.*t8.*t32.*4.0-Izz4.*dQ1.*dQ3.*t2.*t7.*t33.*4.0-Izz4.*dQ1.*dQ3.*t3.*t8.*t32.*4.0-Izz5.*dQ1.*dQ2.*t2.*t7.*t34.*2.0+Izz5.*dQ1.*dQ2.*t2.*t7.*t35.*2.0-Izz5.*dQ1.*dQ3.*t2.*t7.*t34.*2.0-Izz6.*dQ1.*dQ2.*t2.*t7.*t34.*2.0-Izz5.*dQ1.*dQ2.*t3.*t8.*t34.*2.0+Izz5.*dQ1.*dQ3.*t2.*t7.*t35.*2.0;
et43 = Izz6.*dQ1.*dQ2.*t2.*t7.*t35.*2.0-Izz6.*dQ1.*dQ3.*t2.*t7.*t34.*2.0+Izz5.*dQ1.*dQ2.*t3.*t8.*t35.*2.0-Izz5.*dQ1.*dQ3.*t3.*t8.*t34.*2.0-Izz6.*dQ1.*dQ2.*t3.*t8.*t34.*2.0+Izz6.*dQ1.*dQ3.*t2.*t7.*t35.*2.0+Izz5.*dQ1.*dQ3.*t3.*t8.*t35.*2.0-Izz5.*dQ1.*dQ4.*t4.*t9.*t32.*2.0-Izz5.*dQ2.*dQ4.*t2.*t8.*t34.*2.0-Izz5.*dQ2.*dQ4.*t3.*t7.*t34.*2.0+Izz6.*dQ1.*dQ2.*t3.*t8.*t35.*2.0-Izz6.*dQ1.*dQ3.*t3.*t8.*t34.*2.0-Izz5.*dQ1.*dQ4.*t4.*t9.*t33.*2.0-Izz5.*dQ2.*dQ4.*t2.*t8.*t35.*2.0-Izz5.*dQ2.*dQ4.*t3.*t7.*t35.*2.0-Izz5.*dQ3.*dQ4.*t2.*t8.*t34.*2.0-Izz5.*dQ3.*dQ4.*t3.*t7.*t34.*2.0+Izz6.*dQ1.*dQ3.*t3.*t8.*t35.*2.0-Izz6.*dQ1.*dQ4.*t4.*t9.*t32.*2.0-Izz6.*dQ2.*dQ4.*t2.*t8.*t34.*2.0-Izz6.*dQ2.*dQ4.*t3.*t7.*t34.*2.0-Izz5.*dQ3.*dQ4.*t2.*t8.*t35.*2.0;
et44 = Izz5.*dQ3.*dQ4.*t3.*t7.*t35.*-2.0-Izz6.*dQ1.*dQ4.*t4.*t9.*t33.*2.0-Izz6.*dQ2.*dQ4.*t2.*t8.*t35.*2.0-Izz6.*dQ2.*dQ4.*t3.*t7.*t35.*2.0-Izz6.*dQ3.*dQ4.*t2.*t8.*t34.*2.0-Izz6.*dQ3.*dQ4.*t3.*t7.*t34.*2.0+Izz5.*dQ1.*dQ5.*t5.*t10.*t32.*2.0-Izz6.*dQ3.*dQ4.*t2.*t8.*t35.*2.0-Izz6.*dQ3.*dQ4.*t3.*t7.*t35.*2.0+Izz5.*dQ1.*dQ5.*t5.*t10.*t33.*2.0+Izz6.*dQ1.*dQ5.*t5.*t10.*t32.*2.0+Izz6.*dQ1.*dQ5.*t5.*t10.*t33.*2.0-dQ2.*dQ4.*m4.*t2.*t8.*t15.*2.0-dQ2.*dQ4.*m4.*t3.*t7.*t15.*2.0-dQ3.*dQ4.*m4.*t2.*t8.*t15.*2.0-dQ3.*dQ4.*m4.*t3.*t7.*t15.*2.0-dQ2.*dQ4.*m6.*t2.*t8.*t22.*2.0-dQ2.*dQ4.*m6.*t3.*t7.*t22.*2.0-dQ3.*dQ4.*m6.*t2.*t8.*t22.*2.0-dQ3.*dQ4.*m6.*t3.*t7.*t22.*2.0-dQ2.*dQ4.*m5.*t2.*t8.*t25.*2.0-dQ2.*dQ4.*m5.*t3.*t7.*t25.*2.0;
et45 = dQ3.*dQ4.*m5.*t2.*t8.*t25.*-2.0-dQ3.*dQ4.*m5.*t3.*t7.*t25.*2.0-dQ2.*dQ4.*m6.*t2.*t8.*t26.*2.0-dQ2.*dQ4.*m6.*t3.*t7.*t26.*2.0-dQ3.*dQ4.*m6.*t2.*t8.*t26.*2.0-dQ3.*dQ4.*m6.*t3.*t7.*t26.*2.0-Lx2.*Lx3.*dQ1.*dQ2.*m4.*t8.*t32.*4.0-Lx2.*Lx3.*dQ1.*dQ2.*m5.*t8.*t32.*4.0-Lx2.*Lx3.*dQ1.*dQ3.*m4.*t8.*t32.*2.0-Lx2.*Lx3.*dQ1.*dQ2.*m6.*t8.*t32.*4.0-Lx2.*Lx3.*dQ1.*dQ3.*m5.*t8.*t32.*2.0-Lx2.*Lx3.*dQ1.*dQ3.*m6.*t8.*t32.*2.0+Lx2.*Lxcm4.*dQ1.*dQ2.*m4.*t4.*t8.*2.0+Lx2.*Lxcm5.*dQ1.*dQ2.*m5.*t3.*t10.*2.0-Lx3.*Lxcm5.*dQ1.*dQ4.*m5.*t5.*t9.*2.0-Lx3.*Lxcm5.*dQ1.*dQ5.*m5.*t4.*t10.*2.0-Lx3.*Lxcm6.*dQ1.*dQ2.*m6.*t6.*t10.*2.0-Lx3.*Lxcm6.*dQ1.*dQ3.*m6.*t6.*t10.*2.0-Lx3.*Lxcm6.*dQ1.*dQ4.*m6.*t4.*t11.*2.0-Lx3.*Lxcm6.*dQ1.*dQ6.*m6.*t6.*t9.*2.0;
et46 = Lx2.*Lxcm3.*dQ1.*dQ2.*m3.*t8.*t32.*-4.0-Lx2.*Lxcm3.*dQ1.*dQ3.*m3.*t8.*t32.*2.0+Lx3.*Lxcm4.*dQ1.*dQ4.*m4.*t9.*t32.*2.0+Lx3.*Lxcm4.*dQ1.*dQ4.*m4.*t9.*t33.*2.0+Lx3.*Lxcm5.*dQ1.*dQ2.*m5.*t10.*t32.*4.0+Lx3.*Lxcm5.*dQ1.*dQ2.*m5.*t10.*t33.*4.0+Lx3.*Lxcm5.*dQ1.*dQ3.*m5.*t10.*t32.*4.0+Lx3.*Lxcm5.*dQ1.*dQ3.*m5.*t10.*t33.*4.0-Lx2.*Lycm4.*dQ1.*dQ2.*m4.*t8.*t9.*2.0-Lx3.*Lycm6.*dQ1.*dQ4.*m6.*t4.*t6.*2.0-Lx2.*Lycm5.*dQ1.*dQ2.*m5.*t8.*t9.*2.0+Lx3.*Lycm6.*dQ1.*dQ2.*m6.*t10.*t11.*2.0+Lx3.*Lycm6.*dQ1.*dQ3.*m6.*t10.*t11.*2.0+Lx3.*Lycm6.*dQ1.*dQ6.*m6.*t9.*t11.*2.0+Lx3.*Lycm4.*dQ1.*dQ4.*m4.*t4.*t32.*2.0+Lx3.*Lycm4.*dQ1.*dQ4.*m4.*t4.*t33.*2.0+Lx3.*Lycm5.*dQ1.*dQ4.*m5.*t4.*t32.*2.0+Lx3.*Lycm5.*dQ1.*dQ4.*m5.*t4.*t33.*2.0+Lxcm3.*Lycm3.*dQ2.*dQ3.*m3.*t2.*t3.*2.0-Lxcm4.*Lycm4.*dQ2.*dQ3.*m4.*t2.*t3.*2.0-Lxcm3.*Lycm3.*dQ2.*dQ3.*m3.*t7.*t8.*2.0;
et47 = Lxcm4.*Lycm4.*dQ2.*dQ3.*m4.*t7.*t8.*2.0-Lxcm6.*Lycm6.*dQ4.*dQ6.*m6.*t2.*t3.*2.0+Lxcm5.*Lycm5.*dQ1.*dQ2.*m5.*t9.*t10.*2.0+Lxcm5.*Lycm5.*dQ1.*dQ3.*m5.*t9.*t10.*2.0-Lxcm6.*Lycm6.*dQ1.*dQ2.*m6.*t9.*t10.*2.0-Lxcm6.*Lycm6.*dQ1.*dQ3.*m6.*t9.*t10.*2.0+Lxcm6.*Lycm6.*dQ4.*dQ6.*m6.*t7.*t8.*2.0-Lxcm5.*Lycm5.*dQ1.*dQ4.*m5.*t5.*t32.*2.0-Lxcm5.*Lycm5.*dQ1.*dQ4.*m5.*t5.*t33.*2.0+Lxcm6.*Lycm6.*dQ1.*dQ4.*m6.*t5.*t32.*2.0+Lxcm6.*Lycm6.*dQ1.*dQ4.*m6.*t5.*t33.*2.0+Lxcm4.*Lycm4.*dQ1.*dQ4.*m4.*t32.*t33.*4.0+Lxcm4.*Lycm4.*dQ1.*dQ4.*m4.*t32.*t34.*4.0+Lxcm4.*Lycm4.*dQ1.*dQ4.*m4.*t33.*t34.*4.0-Lxcm6.*Lycm6.*dQ1.*dQ6.*m6.*t32.*t33.*8.0-Lxcm6.*Lycm6.*dQ1.*dQ6.*m6.*t32.*t34.*2.0-Lxcm6.*Lycm6.*dQ1.*dQ6.*m6.*t32.*t35.*2.0-Lxcm6.*Lycm6.*dQ1.*dQ6.*m6.*t33.*t34.*2.0-Lxcm6.*Lycm6.*dQ1.*dQ6.*m6.*t32.*t36.*8.0-Lxcm6.*Lycm6.*dQ1.*dQ6.*m6.*t33.*t35.*2.0;
et48 = Lxcm6.*Lycm6.*dQ1.*dQ6.*m6.*t33.*t36.*-8.0-Lxcm6.*Lycm6.*dQ1.*dQ6.*m6.*t35.*t36.*4.0-Lx2.*Lz5.*dQ1.*dQ2.*m6.*t3.*t5.*2.0+Lx3.*Lz5.*dQ1.*dQ5.*m6.*t4.*t5.*2.0-Lx3.*Lz5.*dQ1.*dQ4.*m6.*t9.*t10.*2.0+Lx2.*Lz4.*dQ1.*dQ2.*m5.*t3.*t32.*4.0+Lx2.*Lz4.*dQ1.*dQ2.*m6.*t3.*t32.*4.0+Lx2.*Lz4.*dQ1.*dQ3.*m5.*t3.*t32.*2.0+Lx2.*Lz4.*dQ1.*dQ3.*m6.*t3.*t32.*2.0-Lx3.*Lz5.*dQ1.*dQ2.*m6.*t5.*t32.*4.0-Lx3.*Lz5.*dQ1.*dQ2.*m6.*t5.*t33.*4.0-Lx3.*Lz5.*dQ1.*dQ3.*m6.*t5.*t32.*4.0-Lx3.*Lz5.*dQ1.*dQ3.*m6.*t5.*t33.*4.0+Lx3.*Lz4.*dQ1.*dQ2.*m5.*t32.*t33.*8.0+Lx3.*Lz4.*dQ1.*dQ2.*m6.*t32.*t33.*8.0+Lx3.*Lz4.*dQ1.*dQ3.*m5.*t32.*t33.*8.0+Lx3.*Lz4.*dQ1.*dQ3.*m6.*t32.*t33.*8.0-Lx2.*Lzcm5.*dQ1.*dQ2.*m5.*t3.*t5.*2.0-Lx2.*Lzcm6.*dQ1.*dQ2.*m6.*t3.*t5.*2.0+Lxcm5.*Lz4.*dQ1.*dQ2.*m5.*t4.*t5.*2.0;
et49 = Lxcm5.*Lz4.*dQ1.*dQ3.*m5.*t4.*t5.*2.0+Lx3.*Lzcm5.*dQ1.*dQ5.*m5.*t4.*t5.*2.0+Lx3.*Lzcm6.*dQ1.*dQ5.*m6.*t4.*t5.*2.0-Lxcm6.*Lz5.*dQ1.*dQ2.*m6.*t4.*t6.*2.0-Lxcm6.*Lz5.*dQ1.*dQ3.*m6.*t4.*t6.*2.0-Lx3.*Lzcm5.*dQ1.*dQ4.*m5.*t9.*t10.*2.0-Lx3.*Lzcm6.*dQ1.*dQ4.*m6.*t9.*t10.*2.0-Lxcm6.*Lz4.*dQ1.*dQ2.*m6.*t9.*t11.*2.0-Lxcm6.*Lz4.*dQ1.*dQ3.*m6.*t9.*t11.*2.0+Lx2.*Lzcm3.*dQ1.*dQ2.*m3.*t3.*t32.*4.0+Lx2.*Lzcm3.*dQ1.*dQ3.*m3.*t3.*t32.*2.0+Lx2.*Lzcm4.*dQ1.*dQ2.*m4.*t3.*t32.*4.0+Lx2.*Lzcm4.*dQ1.*dQ3.*m4.*t3.*t32.*2.0-Lx3.*Lzcm5.*dQ1.*dQ2.*m5.*t5.*t32.*4.0-Lx3.*Lzcm5.*dQ1.*dQ2.*m5.*t5.*t33.*4.0-Lx3.*Lzcm5.*dQ1.*dQ3.*m5.*t5.*t32.*4.0-Lx3.*Lzcm5.*dQ1.*dQ3.*m5.*t5.*t33.*4.0-Lx3.*Lzcm6.*dQ1.*dQ2.*m6.*t5.*t32.*4.0-Lx3.*Lzcm6.*dQ1.*dQ2.*m6.*t5.*t33.*4.0-Lx3.*Lzcm6.*dQ1.*dQ3.*m6.*t5.*t32.*4.0;
et50 = Lx3.*Lzcm6.*dQ1.*dQ3.*m6.*t5.*t33.*-4.0-Lxcm5.*Lz4.*dQ1.*dQ5.*m5.*t5.*t32.*2.0-Lxcm5.*Lz4.*dQ1.*dQ5.*m5.*t5.*t33.*2.0+Lxcm6.*Lz5.*dQ1.*dQ5.*m6.*t6.*t32.*2.0+Lxcm6.*Lz5.*dQ1.*dQ5.*m6.*t6.*t33.*2.0+Lxcm6.*Lz5.*dQ1.*dQ5.*m6.*t6.*t35.*4.0+Lx3.*Lzcm4.*dQ1.*dQ2.*m4.*t32.*t33.*8.0+Lx3.*Lzcm4.*dQ1.*dQ3.*m4.*t32.*t33.*8.0-Lxcm5.*Lzcm5.*dQ4.*dQ5.*m5.*t2.*t3.*2.0-Lxcm6.*Lzcm6.*dQ1.*dQ2.*m6.*t4.*t6.*2.0-Lxcm6.*Lzcm6.*dQ1.*dQ3.*m6.*t4.*t6.*2.0+Lxcm5.*Lzcm5.*dQ4.*dQ5.*m5.*t7.*t8.*2.0-Lxcm4.*Lzcm4.*dQ1.*dQ2.*m4.*t4.*t32.*4.0-Lxcm4.*Lzcm4.*dQ1.*dQ2.*m4.*t4.*t33.*4.0-Lxcm4.*Lzcm4.*dQ1.*dQ3.*m4.*t4.*t32.*4.0-Lxcm4.*Lzcm4.*dQ1.*dQ3.*m4.*t4.*t33.*4.0+Lxcm5.*Lzcm5.*dQ1.*dQ2.*m5.*t4.*t32.*4.0+Lxcm5.*Lzcm5.*dQ1.*dQ2.*m5.*t4.*t33.*4.0+Lxcm5.*Lzcm5.*dQ1.*dQ3.*m5.*t4.*t32.*4.0+Lxcm5.*Lzcm5.*dQ1.*dQ3.*m5.*t4.*t33.*4.0;
et51 = Lxcm5.*Lzcm5.*dQ1.*dQ2.*m5.*t4.*t35.*4.0+Lxcm5.*Lzcm5.*dQ1.*dQ3.*m5.*t4.*t35.*4.0+Lxcm6.*Lzcm6.*dQ1.*dQ5.*m6.*t6.*t32.*2.0+Lxcm6.*Lzcm6.*dQ1.*dQ5.*m6.*t6.*t33.*2.0+Lxcm6.*Lzcm6.*dQ1.*dQ5.*m6.*t6.*t35.*4.0+Lxcm3.*Lzcm3.*dQ1.*dQ2.*m3.*t32.*t33.*8.0+Lxcm3.*Lzcm3.*dQ1.*dQ3.*m3.*t32.*t33.*8.0-Lxcm5.*Lzcm5.*dQ1.*dQ5.*m5.*t32.*t33.*4.0+Lxcm5.*Lzcm5.*dQ1.*dQ5.*m5.*t32.*t34.*2.0-Lxcm5.*Lzcm5.*dQ1.*dQ5.*m5.*t32.*t35.*4.0+Lxcm5.*Lzcm5.*dQ1.*dQ5.*m5.*t33.*t34.*2.0-Lxcm5.*Lzcm5.*dQ1.*dQ5.*m5.*t33.*t35.*4.0-Lycm6.*Lz4.*dQ1.*dQ2.*m6.*t6.*t9.*2.0-Lycm6.*Lz4.*dQ1.*dQ3.*m6.*t6.*t9.*2.0+Lycm6.*Lz5.*dQ1.*dQ2.*m6.*t4.*t11.*2.0+Lycm6.*Lz5.*dQ1.*dQ3.*m6.*t4.*t11.*2.0+Lycm5.*Lz4.*dQ1.*dQ2.*m5.*t9.*t32.*4.0+Lycm5.*Lz4.*dQ1.*dQ2.*m5.*t9.*t33.*4.0+Lycm5.*Lz4.*dQ1.*dQ3.*m5.*t9.*t32.*4.0+Lycm5.*Lz4.*dQ1.*dQ3.*m5.*t9.*t33.*4.0-Lycm6.*Lz5.*dQ1.*dQ5.*m6.*t11.*t32.*2.0;
et52 = Lycm6.*Lz5.*dQ1.*dQ5.*m6.*t11.*t33.*-2.0-Lycm6.*Lz5.*dQ1.*dQ5.*m6.*t11.*t35.*4.0+Lycm3.*Lzcm3.*dQ2.*dQ3.*m3.*t2.*t8.*2.0+Lycm3.*Lzcm3.*dQ2.*dQ3.*m3.*t3.*t7.*2.0-Lycm5.*Lzcm5.*dQ1.*dQ2.*m5.*t5.*t9.*2.0-Lycm5.*Lzcm5.*dQ1.*dQ3.*m5.*t5.*t9.*2.0+Lycm6.*Lzcm6.*dQ1.*dQ2.*m6.*t4.*t11.*2.0+Lycm6.*Lzcm6.*dQ1.*dQ3.*m6.*t4.*t11.*2.0+Lycm4.*Lzcm4.*dQ1.*dQ2.*m4.*t9.*t32.*4.0+Lycm4.*Lzcm4.*dQ1.*dQ2.*m4.*t9.*t33.*4.0+Lycm4.*Lzcm4.*dQ1.*dQ3.*m4.*t9.*t32.*4.0+Lycm4.*Lzcm4.*dQ1.*dQ3.*m4.*t9.*t33.*4.0-Lycm5.*Lzcm5.*dQ1.*dQ4.*m5.*t10.*t32.*2.0-Lycm5.*Lzcm5.*dQ1.*dQ4.*m5.*t10.*t33.*2.0-Lycm6.*Lzcm6.*dQ1.*dQ5.*m6.*t11.*t32.*2.0-Lycm6.*Lzcm6.*dQ1.*dQ5.*m6.*t11.*t33.*2.0-Lycm6.*Lzcm6.*dQ1.*dQ5.*m6.*t11.*t35.*4.0+Lz4.*Lz5.*dQ1.*dQ2.*m6.*t4.*t10.*2.0+Lz4.*Lz5.*dQ1.*dQ3.*m6.*t4.*t10.*2.0-Lz4.*Lz5.*dQ1.*dQ5.*m6.*t10.*t32.*2.0-Lz4.*Lz5.*dQ1.*dQ5.*m6.*t10.*t33.*2.0;
et53 = Lz4.*Lzcm5.*dQ1.*dQ2.*m5.*t4.*t10.*2.0+Lz4.*Lzcm5.*dQ1.*dQ3.*m5.*t4.*t10.*2.0+Lz4.*Lzcm6.*dQ1.*dQ2.*m6.*t4.*t10.*2.0-Lz5.*Lzcm6.*dQ2.*dQ4.*m6.*t2.*t8.*4.0-Lz5.*Lzcm6.*dQ2.*dQ4.*m6.*t3.*t7.*4.0+Lz4.*Lzcm6.*dQ1.*dQ3.*m6.*t4.*t10.*2.0-Lz5.*Lzcm6.*dQ3.*dQ4.*m6.*t2.*t8.*4.0-Lz5.*Lzcm6.*dQ3.*dQ4.*m6.*t3.*t7.*4.0-Lz4.*Lzcm5.*dQ1.*dQ5.*m5.*t10.*t32.*2.0-Lz4.*Lzcm5.*dQ1.*dQ5.*m5.*t10.*t33.*2.0-Lz4.*Lzcm6.*dQ1.*dQ5.*m6.*t10.*t32.*2.0-Lz4.*Lzcm6.*dQ1.*dQ5.*m6.*t10.*t33.*2.0-Ixx4.*dQ2.*dQ3.*t2.*t3.*t4.*t9.*2.0+Ixx6.*dQ2.*dQ3.*t2.*t3.*t4.*t9.*2.0+Ixx6.*dQ2.*dQ6.*t2.*t3.*t4.*t10+Ixx5.*dQ4.*dQ5.*t2.*t3.*t5.*t10.*2.0+Ixx6.*dQ3.*dQ6.*t2.*t3.*t4.*t10+Ixx6.*dQ5.*dQ6.*t2.*t4.*t5.*t8+Ixx6.*dQ5.*dQ6.*t3.*t4.*t5.*t7+Ixx4.*dQ2.*dQ3.*t4.*t7.*t8.*t9.*2.0-Ixx6.*dQ4.*dQ6.*t2.*t3.*t6.*t11.*2.0;
et54 = Ixx6.*dQ2.*dQ3.*t4.*t7.*t8.*t9.*-2.0-Ixx6.*dQ1.*dQ6.*t2.*t7.*t9.*t10.*2.0-Ixx6.*dQ1.*dQ6.*t3.*t8.*t9.*t10.*2.0-Ixx6.*dQ2.*dQ6.*t4.*t7.*t8.*t10-Ixx5.*dQ4.*dQ5.*t5.*t7.*t8.*t10.*2.0-Ixx6.*dQ3.*dQ6.*t4.*t7.*t8.*t10-Ixx6.*dQ1.*dQ2.*t6.*t9.*t10.*t11.*2.0+Ixx6.*dQ4.*dQ6.*t2.*t8.*t9.*t10+Ixx6.*dQ4.*dQ6.*t3.*t7.*t9.*t10-Ixx6.*dQ1.*dQ3.*t6.*t9.*t10.*t11.*2.0+Ixx6.*dQ4.*dQ6.*t6.*t7.*t8.*t11.*2.0-Ixx5.*dQ1.*dQ5.*t2.*t4.*t7.*t33.*4.0-Ixx5.*dQ1.*dQ5.*t3.*t4.*t8.*t32.*4.0-Ixx5.*dQ1.*dQ2.*t4.*t5.*t10.*t32.*4.0-Ixx5.*dQ1.*dQ5.*t2.*t4.*t7.*t35.*4.0-Ixx5.*dQ1.*dQ2.*t4.*t5.*t10.*t33.*4.0-Ixx5.*dQ1.*dQ3.*t4.*t5.*t10.*t32.*4.0-Ixx5.*dQ1.*dQ3.*t4.*t5.*t10.*t33.*4.0-Ixx5.*dQ1.*dQ5.*t3.*t4.*t8.*t35.*4.0-Ixx5.*dQ2.*dQ5.*t2.*t3.*t9.*t35.*2.0;
et55 = Ixx6.*dQ1.*dQ5.*t2.*t4.*t7.*t36.*2.0-Ixx5.*dQ3.*dQ5.*t2.*t3.*t9.*t35.*2.0+Ixx5.*dQ4.*dQ5.*t2.*t4.*t8.*t35.*2.0+Ixx5.*dQ4.*dQ5.*t3.*t4.*t7.*t35.*2.0+Ixx6.*dQ1.*dQ5.*t3.*t4.*t8.*t36.*2.0+Ixx6.*dQ1.*dQ6.*t4.*t5.*t9.*t32.*2.0+Ixx6.*dQ2.*dQ6.*t2.*t5.*t8.*t34.*2.0+Ixx6.*dQ2.*dQ6.*t3.*t5.*t7.*t34.*2.0+Ixx6.*dQ1.*dQ2.*t4.*t5.*t10.*t36.*2.0+Ixx6.*dQ1.*dQ6.*t4.*t5.*t9.*t33.*2.0+Ixx6.*dQ3.*dQ6.*t2.*t5.*t8.*t34.*2.0+Ixx6.*dQ3.*dQ6.*t3.*t5.*t7.*t34.*2.0+Ixx6.*dQ1.*dQ3.*t4.*t5.*t10.*t36.*2.0+Ixx6.*dQ1.*dQ4.*t5.*t6.*t11.*t32.*2.0+Ixx6.*dQ2.*dQ6.*t2.*t5.*t8.*t36.*2.0+Ixx6.*dQ2.*dQ6.*t3.*t5.*t7.*t36.*2.0-Ixx6.*dQ4.*dQ5.*t2.*t4.*t8.*t36.*2.0-Ixx6.*dQ4.*dQ5.*t3.*t4.*t7.*t36.*2.0+Ixx6.*dQ1.*dQ4.*t5.*t6.*t11.*t33.*2.0+Ixx6.*dQ3.*dQ6.*t2.*t5.*t8.*t36.*2.0+Ixx6.*dQ3.*dQ6.*t3.*t5.*t7.*t36.*2.0;
et56 = Ixx6.*dQ5.*dQ6.*t2.*t3.*t10.*t36.*-2.0+Ixx5.*dQ2.*dQ5.*t7.*t8.*t9.*t35.*2.0+Ixx5.*dQ3.*dQ5.*t7.*t8.*t9.*t35.*2.0+Ixx6.*dQ5.*dQ6.*t7.*t8.*t10.*t36.*2.0+Ixx4.*dQ1.*dQ2.*t2.*t7.*t33.*t34.*4.0+Ixx4.*dQ1.*dQ2.*t3.*t8.*t32.*t34.*4.0+Ixx4.*dQ1.*dQ3.*t2.*t7.*t33.*t34.*4.0+Ixx4.*dQ1.*dQ3.*t3.*t8.*t32.*t34.*4.0+Ixx5.*dQ1.*dQ2.*t2.*t7.*t33.*t35.*4.0-Ixx6.*dQ1.*dQ2.*t2.*t7.*t33.*t34.*4.0-Ixx5.*dQ1.*dQ2.*t2.*t7.*t34.*t35.*2.0+Ixx5.*dQ1.*dQ2.*t3.*t8.*t32.*t35.*4.0+Ixx5.*dQ1.*dQ3.*t2.*t7.*t33.*t35.*4.0-Ixx6.*dQ1.*dQ2.*t3.*t8.*t32.*t34.*4.0-Ixx6.*dQ1.*dQ3.*t2.*t7.*t33.*t34.*4.0+Ixx4.*dQ1.*dQ4.*t4.*t9.*t32.*t33.*4.0-Ixx5.*dQ1.*dQ3.*t2.*t7.*t34.*t35.*2.0+Ixx5.*dQ1.*dQ3.*t3.*t8.*t32.*t35.*4.0-Ixx6.*dQ1.*dQ2.*t2.*t7.*t33.*t36.*8.0-Ixx6.*dQ1.*dQ3.*t3.*t8.*t32.*t34.*4.0-Ixx5.*dQ1.*dQ2.*t3.*t8.*t34.*t35.*2.0;
et57 = Ixx6.*dQ1.*dQ2.*t2.*t7.*t34.*t36.*-2.0-Ixx6.*dQ1.*dQ2.*t3.*t8.*t32.*t36.*8.0-Ixx6.*dQ1.*dQ3.*t2.*t7.*t33.*t36.*8.0-Ixx5.*dQ1.*dQ3.*t3.*t8.*t34.*t35.*2.0-Ixx6.*dQ1.*dQ2.*t2.*t7.*t35.*t36.*2.0-Ixx6.*dQ1.*dQ3.*t2.*t7.*t34.*t36.*2.0-Ixx6.*dQ1.*dQ3.*t3.*t8.*t32.*t36.*8.0-Ixx6.*dQ1.*dQ4.*t4.*t9.*t32.*t33.*4.0-Ixx5.*dQ1.*dQ4.*t4.*t9.*t32.*t35.*2.0-Ixx5.*dQ2.*dQ4.*t2.*t8.*t34.*t35.*2.0-Ixx5.*dQ2.*dQ4.*t3.*t7.*t34.*t35.*2.0-Ixx6.*dQ1.*dQ2.*t3.*t8.*t34.*t36.*2.0-Ixx6.*dQ1.*dQ3.*t2.*t7.*t35.*t36.*2.0-Ixx5.*dQ1.*dQ4.*t4.*t9.*t33.*t35.*2.0+Ixx5.*dQ1.*dQ5.*t5.*t10.*t32.*t33.*4.0-Ixx5.*dQ3.*dQ4.*t2.*t8.*t34.*t35.*2.0-Ixx5.*dQ3.*dQ4.*t3.*t7.*t34.*t35.*2.0-Ixx6.*dQ1.*dQ2.*t3.*t8.*t35.*t36.*2.0-Ixx6.*dQ1.*dQ3.*t3.*t8.*t34.*t36.*2.0;
et58 = Ixx5.*dQ1.*dQ5.*t5.*t10.*t32.*t34.*-2.0-Ixx6.*dQ1.*dQ3.*t3.*t8.*t35.*t36.*2.0-Ixx6.*dQ1.*dQ4.*t4.*t9.*t32.*t36.*2.0-Ixx6.*dQ2.*dQ4.*t2.*t8.*t34.*t36.*2.0-Ixx6.*dQ2.*dQ4.*t3.*t7.*t34.*t36.*2.0-Ixx5.*dQ1.*dQ5.*t5.*t10.*t33.*t34.*2.0-Ixx6.*dQ1.*dQ4.*t4.*t9.*t33.*t36.*2.0+Ixx6.*dQ2.*dQ4.*t2.*t8.*t35.*t36.*2.0+Ixx6.*dQ2.*dQ4.*t3.*t7.*t35.*t36.*2.0-Ixx6.*dQ3.*dQ4.*t2.*t8.*t34.*t36.*2.0-Ixx6.*dQ3.*dQ4.*t3.*t7.*t34.*t36.*2.0+Ixx6.*dQ3.*dQ4.*t2.*t8.*t35.*t36.*2.0+Ixx6.*dQ3.*dQ4.*t3.*t7.*t35.*t36.*2.0-Ixx6.*dQ1.*dQ5.*t5.*t10.*t32.*t36.*2.0-Ixx6.*dQ1.*dQ6.*t6.*t11.*t32.*t33.*8.0-Ixx6.*dQ1.*dQ5.*t5.*t10.*t33.*t36.*2.0-Ixx6.*dQ1.*dQ6.*t6.*t11.*t32.*t34.*2.0-Ixx6.*dQ1.*dQ6.*t6.*t11.*t32.*t35.*2.0-Ixx6.*dQ1.*dQ6.*t6.*t11.*t33.*t34.*2.0-Ixx6.*dQ1.*dQ6.*t6.*t11.*t33.*t35.*2.0;
et59 = Ixy5.*dQ2.*dQ5.*t2.*t3.*t4.*t5+Ixy5.*dQ3.*dQ5.*t2.*t3.*t4.*t5-Ixy6.*dQ2.*dQ5.*t2.*t3.*t4.*t5-Ixy6.*dQ3.*dQ5.*t2.*t3.*t4.*t5-Ixy4.*dQ1.*dQ2.*t2.*t4.*t7.*t9.*2.0-Ixy4.*dQ1.*dQ4.*t2.*t3.*t7.*t8.*2.0-Ixy4.*dQ1.*dQ3.*t2.*t4.*t7.*t9.*2.0-Ixy4.*dQ1.*dQ2.*t3.*t4.*t8.*t9.*2.0-Ixy4.*dQ1.*dQ3.*t3.*t4.*t8.*t9.*2.0-Ixy5.*dQ1.*dQ4.*t2.*t4.*t7.*t10+Ixy6.*dQ1.*dQ6.*t2.*t3.*t7.*t8.*4.0-Ixy5.*dQ1.*dQ5.*t2.*t5.*t7.*t9-Ixy5.*dQ2.*dQ3.*t2.*t4.*t8.*t10-Ixy5.*dQ2.*dQ3.*t3.*t4.*t7.*t10+Ixy6.*dQ1.*dQ4.*t2.*t4.*t7.*t10-Ixy5.*dQ1.*dQ4.*t3.*t4.*t8.*t10+Ixy6.*dQ1.*dQ2.*t2.*t6.*t7.*t11.*4.0+Ixy6.*dQ1.*dQ5.*t2.*t5.*t7.*t9+Ixy6.*dQ2.*dQ3.*t2.*t4.*t8.*t10+Ixy6.*dQ2.*dQ3.*t3.*t4.*t7.*t10-Ixy5.*dQ1.*dQ5.*t3.*t5.*t8.*t9;
et60 = -Ixy5.*dQ2.*dQ5.*t4.*t5.*t7.*t8+Ixy6.*dQ1.*dQ3.*t2.*t6.*t7.*t11.*4.0+Ixy6.*dQ1.*dQ4.*t3.*t4.*t8.*t10-Ixy5.*dQ3.*dQ5.*t4.*t5.*t7.*t8+Ixy6.*dQ1.*dQ2.*t3.*t6.*t8.*t11.*4.0+Ixy6.*dQ1.*dQ5.*t3.*t5.*t8.*t9+Ixy6.*dQ2.*dQ5.*t4.*t5.*t7.*t8+Ixy6.*dQ2.*dQ6.*t2.*t4.*t8.*t9+Ixy6.*dQ2.*dQ6.*t3.*t4.*t7.*t9+Ixy6.*dQ1.*dQ3.*t3.*t6.*t8.*t11.*4.0+Ixy6.*dQ3.*dQ5.*t4.*t5.*t7.*t8+Ixy6.*dQ3.*dQ6.*t2.*t4.*t8.*t9+Ixy6.*dQ3.*dQ6.*t3.*t4.*t7.*t9+Ixy6.*dQ1.*dQ5.*t5.*t6.*t10.*t11.*2.0+Ixy5.*dQ2.*dQ3.*t2.*t3.*t5.*t34.*2.0-Ixy6.*dQ2.*dQ3.*t2.*t3.*t5.*t34.*2.0-Ixy6.*dQ2.*dQ3.*t2.*t3.*t5.*t36.*2.0-Ixy5.*dQ2.*dQ3.*t5.*t7.*t8.*t34.*2.0+Ixy6.*dQ2.*dQ3.*t5.*t7.*t8.*t34.*2.0-Ixy5.*dQ1.*dQ5.*t4.*t9.*t10.*t32-Ixy5.*dQ2.*dQ5.*t2.*t8.*t10.*t34-Ixy5.*dQ2.*dQ5.*t3.*t7.*t10.*t34;
et61 = -Ixy5.*dQ1.*dQ5.*t4.*t9.*t10.*t33-Ixy5.*dQ3.*dQ5.*t2.*t8.*t10.*t34-Ixy5.*dQ3.*dQ5.*t3.*t7.*t10.*t34+Ixy6.*dQ1.*dQ5.*t4.*t9.*t10.*t32+Ixy6.*dQ2.*dQ3.*t5.*t7.*t8.*t36.*2.0+Ixy6.*dQ2.*dQ5.*t2.*t8.*t10.*t34+Ixy6.*dQ2.*dQ5.*t3.*t7.*t10.*t34+Ixy6.*dQ1.*dQ5.*t4.*t9.*t10.*t33+Ixy6.*dQ3.*dQ5.*t2.*t8.*t10.*t34+Ixy6.*dQ3.*dQ5.*t3.*t7.*t10.*t34-Ixy6.*dQ5.*dQ6.*t2.*t8.*t9.*t36.*2.0-Ixy6.*dQ5.*dQ6.*t3.*t7.*t9.*t36.*2.0+Ixy5.*dQ1.*dQ2.*t9.*t10.*t32.*t33.*4.0-Ixy6.*dQ4.*dQ6.*t2.*t3.*t35.*t36.*2.0+Ixy5.*dQ1.*dQ3.*t9.*t10.*t32.*t33.*4.0-Ixy6.*dQ1.*dQ2.*t9.*t10.*t32.*t33.*4.0-Ixy6.*dQ1.*dQ3.*t9.*t10.*t32.*t33.*4.0-Ixy6.*dQ1.*dQ2.*t9.*t10.*t32.*t36.*4.0-Ixy6.*dQ1.*dQ2.*t9.*t10.*t33.*t36.*4.0-Ixy6.*dQ1.*dQ3.*t9.*t10.*t32.*t36.*4.0-Ixy6.*dQ1.*dQ3.*t9.*t10.*t33.*t36.*4.0;
et62 = Ixy6.*dQ4.*dQ6.*t7.*t8.*t35.*t36.*2.0-Ixy5.*dQ1.*dQ4.*t5.*t32.*t33.*t34.*4.0+Ixy6.*dQ1.*dQ4.*t5.*t32.*t33.*t34.*4.0+Ixy6.*dQ1.*dQ4.*t5.*t32.*t33.*t36.*4.0+Ixy6.*dQ1.*dQ4.*t5.*t32.*t34.*t36.*4.0+Ixy6.*dQ1.*dQ4.*t5.*t33.*t34.*t36.*4.0+Ixy6.*dQ1.*dQ6.*t32.*t33.*t34.*t35.*2.0-Ixy6.*dQ1.*dQ6.*t32.*t33.*t34.*t36.*4.0-Ixy6.*dQ1.*dQ6.*t32.*t33.*t35.*t36.*4.0+Ixy6.*dQ1.*dQ6.*t32.*t34.*t35.*t36.*2.0+Ixy6.*dQ1.*dQ6.*t33.*t34.*t35.*t36.*2.0-Ixz3.*dQ1.*dQ2.*t2.*t3.*t7.*t8.*4.0-Ixz3.*dQ1.*dQ3.*t2.*t3.*t7.*t8.*4.0+Ixz5.*dQ1.*dQ5.*t2.*t3.*t7.*t8.*2.0+Ixz5.*dQ1.*dQ2.*t2.*t5.*t7.*t10.*2.0+Ixz5.*dQ1.*dQ3.*t2.*t5.*t7.*t10.*2.0+Ixz5.*dQ1.*dQ2.*t3.*t5.*t8.*t10.*2.0+Ixz5.*dQ1.*dQ3.*t3.*t5.*t8.*t10.*2.0-Ixz6.*dQ1.*dQ4.*t2.*t6.*t7.*t9-Ixz5.*dQ2.*dQ4.*t2.*t5.*t8.*t10.*2.0-Ixz5.*dQ2.*dQ4.*t3.*t5.*t7.*t10.*2.0;
et63 = -Ixz6.*dQ2.*dQ3.*t2.*t6.*t8.*t9-Ixz6.*dQ2.*dQ3.*t3.*t6.*t7.*t9-Ixz5.*dQ3.*dQ4.*t2.*t5.*t8.*t10.*2.0-Ixz5.*dQ3.*dQ4.*t3.*t5.*t7.*t10.*2.0-Ixz6.*dQ1.*dQ4.*t3.*t6.*t8.*t9-Ixz6.*dQ1.*dQ6.*t2.*t4.*t7.*t11-Ixz6.*dQ2.*dQ3.*t2.*t3.*t10.*t11-Ixz6.*dQ1.*dQ6.*t3.*t4.*t8.*t11-Ixz6.*dQ2.*dQ6.*t2.*t3.*t9.*t11-Ixz6.*dQ2.*dQ6.*t2.*t6.*t8.*t10-Ixz6.*dQ2.*dQ6.*t3.*t6.*t7.*t10-Ixz6.*dQ3.*dQ6.*t2.*t3.*t9.*t11-Ixz6.*dQ3.*dQ6.*t2.*t6.*t8.*t10-Ixz6.*dQ3.*dQ6.*t3.*t6.*t7.*t10+Ixz6.*dQ2.*dQ3.*t7.*t8.*t10.*t11+Ixz6.*dQ2.*dQ6.*t7.*t8.*t9.*t11+Ixz6.*dQ3.*dQ6.*t7.*t8.*t9.*t11-Ixz4.*dQ1.*dQ4.*t2.*t7.*t9.*t33.*2.0-Ixz4.*dQ1.*dQ4.*t3.*t8.*t9.*t32.*2.0+Ixz5.*dQ1.*dQ4.*t2.*t7.*t9.*t33.*2.0;
et64 = Ixz6.*dQ4.*dQ5.*t2.*t3.*t6.*t35.*2.0+Ixz5.*dQ1.*dQ4.*t3.*t8.*t9.*t32.*2.0+Ixz5.*dQ1.*dQ4.*t2.*t7.*t9.*t35.*2.0+Ixz5.*dQ2.*dQ3.*t2.*t8.*t9.*t35.*2.0+Ixz5.*dQ2.*dQ3.*t3.*t7.*t9.*t35.*2.0+Ixz5.*dQ1.*dQ4.*t3.*t8.*t9.*t35.*2.0+Ixz6.*dQ1.*dQ2.*t5.*t9.*t11.*t32.*2.0+Ixz6.*dQ1.*dQ2.*t5.*t9.*t11.*t33.*2.0+Ixz6.*dQ1.*dQ3.*t5.*t9.*t11.*t32.*2.0+Ixz6.*dQ1.*dQ3.*t5.*t9.*t11.*t33.*2.0+Ixz6.*dQ1.*dQ6.*t5.*t10.*t11.*t32-Ixz6.*dQ4.*dQ5.*t6.*t7.*t8.*t35.*2.0+Ixz6.*dQ1.*dQ6.*t5.*t10.*t11.*t33-Ixz6.*dQ1.*dQ2.*t4.*t6.*t32.*t33.*4.0-Ixz6.*dQ1.*dQ3.*t4.*t6.*t32.*t33.*4.0-Ixz6.*dQ1.*dQ2.*t4.*t6.*t32.*t35.*4.0-Ixz6.*dQ1.*dQ2.*t4.*t6.*t33.*t35.*4.0-Ixz6.*dQ1.*dQ3.*t4.*t6.*t32.*t35.*4.0-Ixz6.*dQ1.*dQ3.*t4.*t6.*t33.*t35.*4.0+Ixz6.*dQ1.*dQ4.*t10.*t11.*t32.*t33.*2.0+Ixz6.*dQ1.*dQ4.*t10.*t11.*t32.*t34.*2.0;
et65 = Ixz6.*dQ1.*dQ4.*t10.*t11.*t33.*t34.*2.0+Ixz5.*dQ1.*dQ2.*t4.*t32.*t33.*t35.*8.0+Ixz5.*dQ1.*dQ3.*t4.*t32.*t33.*t35.*8.0-Ixz6.*dQ1.*dQ5.*t6.*t32.*t33.*t34.*2.0+Ixz6.*dQ1.*dQ5.*t6.*t32.*t33.*t35.*4.0-Ixz6.*dQ1.*dQ5.*t6.*t32.*t34.*t35.*2.0-Ixz6.*dQ1.*dQ5.*t6.*t33.*t34.*t35.*2.0+Ixz5.*dQ1.*dQ5.*t32.*t33.*t34.*t35.*4.0+Iyx5.*dQ2.*dQ5.*t2.*t3.*t4.*t5+Iyx5.*dQ3.*dQ5.*t2.*t3.*t4.*t5-Iyx6.*dQ2.*dQ5.*t2.*t3.*t4.*t5-Iyx6.*dQ3.*dQ5.*t2.*t3.*t4.*t5-Iyx4.*dQ1.*dQ2.*t2.*t4.*t7.*t9.*2.0-Iyx4.*dQ1.*dQ4.*t2.*t3.*t7.*t8.*2.0-Iyx4.*dQ1.*dQ3.*t2.*t4.*t7.*t9.*2.0-Iyx4.*dQ1.*dQ2.*t3.*t4.*t8.*t9.*2.0-Iyx4.*dQ1.*dQ3.*t3.*t4.*t8.*t9.*2.0-Iyx5.*dQ1.*dQ4.*t2.*t4.*t7.*t10+Iyx6.*dQ1.*dQ6.*t2.*t3.*t7.*t8.*4.0-Iyx5.*dQ1.*dQ5.*t2.*t5.*t7.*t9;
et66 = -Iyx5.*dQ2.*dQ3.*t2.*t4.*t8.*t10-Iyx5.*dQ2.*dQ3.*t3.*t4.*t7.*t10+Iyx6.*dQ1.*dQ4.*t2.*t4.*t7.*t10-Iyx5.*dQ1.*dQ4.*t3.*t4.*t8.*t10+Iyx6.*dQ1.*dQ2.*t2.*t6.*t7.*t11.*4.0+Iyx6.*dQ1.*dQ5.*t2.*t5.*t7.*t9+Iyx6.*dQ2.*dQ3.*t2.*t4.*t8.*t10+Iyx6.*dQ2.*dQ3.*t3.*t4.*t7.*t10-Iyx5.*dQ1.*dQ5.*t3.*t5.*t8.*t9-Iyx5.*dQ2.*dQ5.*t4.*t5.*t7.*t8+Iyx6.*dQ1.*dQ3.*t2.*t6.*t7.*t11.*4.0+Iyx6.*dQ1.*dQ4.*t3.*t4.*t8.*t10-Iyx5.*dQ3.*dQ5.*t4.*t5.*t7.*t8+Iyx6.*dQ1.*dQ2.*t3.*t6.*t8.*t11.*4.0+Iyx6.*dQ1.*dQ5.*t3.*t5.*t8.*t9+Iyx6.*dQ2.*dQ5.*t4.*t5.*t7.*t8+Iyx6.*dQ2.*dQ6.*t2.*t4.*t8.*t9+Iyx6.*dQ2.*dQ6.*t3.*t4.*t7.*t9+Iyx6.*dQ1.*dQ3.*t3.*t6.*t8.*t11.*4.0+Iyx6.*dQ3.*dQ5.*t4.*t5.*t7.*t8+Iyx6.*dQ3.*dQ6.*t2.*t4.*t8.*t9+Iyx6.*dQ3.*dQ6.*t3.*t4.*t7.*t9;
et67 = Iyx6.*dQ1.*dQ5.*t5.*t6.*t10.*t11.*2.0+Iyx5.*dQ2.*dQ3.*t2.*t3.*t5.*t34.*2.0-Iyx6.*dQ2.*dQ3.*t2.*t3.*t5.*t34.*2.0-Iyx6.*dQ2.*dQ3.*t2.*t3.*t5.*t36.*2.0-Iyx5.*dQ2.*dQ3.*t5.*t7.*t8.*t34.*2.0+Iyx6.*dQ2.*dQ3.*t5.*t7.*t8.*t34.*2.0-Iyx5.*dQ1.*dQ5.*t4.*t9.*t10.*t32-Iyx5.*dQ2.*dQ5.*t2.*t8.*t10.*t34-Iyx5.*dQ2.*dQ5.*t3.*t7.*t10.*t34-Iyx5.*dQ1.*dQ5.*t4.*t9.*t10.*t33-Iyx5.*dQ3.*dQ5.*t2.*t8.*t10.*t34-Iyx5.*dQ3.*dQ5.*t3.*t7.*t10.*t34+Iyx6.*dQ1.*dQ5.*t4.*t9.*t10.*t32+Iyx6.*dQ2.*dQ3.*t5.*t7.*t8.*t36.*2.0+Iyx6.*dQ2.*dQ5.*t2.*t8.*t10.*t34+Iyx6.*dQ2.*dQ5.*t3.*t7.*t10.*t34+Iyx6.*dQ1.*dQ5.*t4.*t9.*t10.*t33+Iyx6.*dQ3.*dQ5.*t2.*t8.*t10.*t34+Iyx6.*dQ3.*dQ5.*t3.*t7.*t10.*t34-Iyx6.*dQ5.*dQ6.*t2.*t8.*t9.*t36.*2.0-Iyx6.*dQ5.*dQ6.*t3.*t7.*t9.*t36.*2.0;
et68 = Iyx5.*dQ1.*dQ2.*t9.*t10.*t32.*t33.*4.0-Iyx6.*dQ4.*dQ6.*t2.*t3.*t35.*t36.*2.0+Iyx5.*dQ1.*dQ3.*t9.*t10.*t32.*t33.*4.0-Iyx6.*dQ1.*dQ2.*t9.*t10.*t32.*t33.*4.0-Iyx6.*dQ1.*dQ3.*t9.*t10.*t32.*t33.*4.0-Iyx6.*dQ1.*dQ2.*t9.*t10.*t32.*t36.*4.0-Iyx6.*dQ1.*dQ2.*t9.*t10.*t33.*t36.*4.0-Iyx6.*dQ1.*dQ3.*t9.*t10.*t32.*t36.*4.0-Iyx6.*dQ1.*dQ3.*t9.*t10.*t33.*t36.*4.0+Iyx6.*dQ4.*dQ6.*t7.*t8.*t35.*t36.*2.0-Iyx5.*dQ1.*dQ4.*t5.*t32.*t33.*t34.*4.0+Iyx6.*dQ1.*dQ4.*t5.*t32.*t33.*t34.*4.0+Iyx6.*dQ1.*dQ4.*t5.*t32.*t33.*t36.*4.0+Iyx6.*dQ1.*dQ4.*t5.*t32.*t34.*t36.*4.0+Iyx6.*dQ1.*dQ4.*t5.*t33.*t34.*t36.*4.0+Iyx6.*dQ1.*dQ6.*t32.*t33.*t34.*t35.*2.0-Iyx6.*dQ1.*dQ6.*t32.*t33.*t34.*t36.*4.0-Iyx6.*dQ1.*dQ6.*t32.*t33.*t35.*t36.*4.0+Iyx6.*dQ1.*dQ6.*t32.*t34.*t35.*t36.*2.0+Iyx6.*dQ1.*dQ6.*t33.*t34.*t35.*t36.*2.0+Iyy4.*dQ2.*dQ3.*t2.*t3.*t4.*t9.*2.0;
et69 = Iyy5.*dQ2.*dQ3.*t2.*t3.*t4.*t9.*2.0-Iyy6.*dQ2.*dQ6.*t2.*t3.*t4.*t10-Iyy6.*dQ3.*dQ6.*t2.*t3.*t4.*t10+Iyy6.*dQ4.*dQ5.*t2.*t3.*t5.*t10.*2.0-Iyy6.*dQ5.*dQ6.*t2.*t4.*t5.*t8-Iyy6.*dQ5.*dQ6.*t3.*t4.*t5.*t7-Iyy4.*dQ2.*dQ3.*t4.*t7.*t8.*t9.*2.0-Iyy5.*dQ2.*dQ3.*t4.*t7.*t8.*t9.*2.0+Iyy6.*dQ4.*dQ6.*t2.*t3.*t6.*t11.*2.0+Iyy6.*dQ1.*dQ6.*t2.*t7.*t9.*t10.*2.0+Iyy6.*dQ1.*dQ6.*t3.*t8.*t9.*t10.*2.0+Iyy6.*dQ2.*dQ6.*t4.*t7.*t8.*t10+Iyy6.*dQ3.*dQ6.*t4.*t7.*t8.*t10+Iyy6.*dQ1.*dQ2.*t6.*t9.*t10.*t11.*2.0-Iyy6.*dQ4.*dQ5.*t5.*t7.*t8.*t10.*2.0-Iyy6.*dQ4.*dQ6.*t2.*t8.*t9.*t10-Iyy6.*dQ4.*dQ6.*t3.*t7.*t9.*t10+Iyy6.*dQ1.*dQ3.*t6.*t9.*t10.*t11.*2.0-Iyy6.*dQ4.*dQ6.*t6.*t7.*t8.*t11.*2.0-Iyy6.*dQ1.*dQ5.*t2.*t4.*t7.*t33.*4.0-Iyy6.*dQ1.*dQ5.*t3.*t4.*t8.*t32.*4.0;
et70 = Iyy6.*dQ1.*dQ2.*t4.*t5.*t10.*t32.*-4.0-Iyy6.*dQ1.*dQ5.*t2.*t4.*t7.*t35.*4.0-Iyy6.*dQ1.*dQ2.*t4.*t5.*t10.*t33.*4.0-Iyy6.*dQ1.*dQ3.*t4.*t5.*t10.*t32.*4.0-Iyy6.*dQ1.*dQ5.*t2.*t4.*t7.*t36.*2.0-Iyy6.*dQ1.*dQ3.*t4.*t5.*t10.*t33.*4.0-Iyy6.*dQ1.*dQ5.*t3.*t4.*t8.*t35.*4.0-Iyy6.*dQ2.*dQ5.*t2.*t3.*t9.*t35.*2.0-Iyy6.*dQ1.*dQ5.*t3.*t4.*t8.*t36.*2.0-Iyy6.*dQ1.*dQ6.*t4.*t5.*t9.*t32.*2.0-Iyy6.*dQ2.*dQ6.*t2.*t5.*t8.*t34.*2.0-Iyy6.*dQ2.*dQ6.*t3.*t5.*t7.*t34.*2.0-Iyy6.*dQ3.*dQ5.*t2.*t3.*t9.*t35.*2.0-Iyy6.*dQ1.*dQ2.*t4.*t5.*t10.*t36.*2.0-Iyy6.*dQ1.*dQ6.*t4.*t5.*t9.*t33.*2.0-Iyy6.*dQ3.*dQ6.*t2.*t5.*t8.*t34.*2.0-Iyy6.*dQ3.*dQ6.*t3.*t5.*t7.*t34.*2.0+Iyy6.*dQ4.*dQ5.*t2.*t4.*t8.*t35.*2.0+Iyy6.*dQ4.*dQ5.*t3.*t4.*t7.*t35.*2.0-Iyy6.*dQ1.*dQ3.*t4.*t5.*t10.*t36.*2.0;
et71 = Iyy6.*dQ1.*dQ4.*t5.*t6.*t11.*t32.*-2.0-Iyy6.*dQ2.*dQ6.*t2.*t5.*t8.*t36.*2.0-Iyy6.*dQ2.*dQ6.*t3.*t5.*t7.*t36.*2.0+Iyy6.*dQ4.*dQ5.*t2.*t4.*t8.*t36.*2.0+Iyy6.*dQ4.*dQ5.*t3.*t4.*t7.*t36.*2.0-Iyy6.*dQ1.*dQ4.*t5.*t6.*t11.*t33.*2.0-Iyy6.*dQ3.*dQ6.*t2.*t5.*t8.*t36.*2.0-Iyy6.*dQ3.*dQ6.*t3.*t5.*t7.*t36.*2.0+Iyy6.*dQ5.*dQ6.*t2.*t3.*t10.*t36.*2.0+Iyy6.*dQ2.*dQ5.*t7.*t8.*t9.*t35.*2.0+Iyy6.*dQ3.*dQ5.*t7.*t8.*t9.*t35.*2.0-Iyy6.*dQ5.*dQ6.*t7.*t8.*t10.*t36.*2.0-Iyy4.*dQ1.*dQ2.*t2.*t7.*t33.*t34.*4.0-Iyy4.*dQ1.*dQ2.*t3.*t8.*t32.*t34.*4.0-Iyy4.*dQ1.*dQ3.*t2.*t7.*t33.*t34.*4.0-Iyy5.*dQ1.*dQ2.*t2.*t7.*t33.*t34.*4.0-Iyy4.*dQ1.*dQ3.*t3.*t8.*t32.*t34.*4.0-Iyy5.*dQ1.*dQ2.*t3.*t8.*t32.*t34.*4.0-Iyy5.*dQ1.*dQ3.*t2.*t7.*t33.*t34.*4.0-Iyy5.*dQ1.*dQ3.*t3.*t8.*t32.*t34.*4.0;
et72 = Iyy6.*dQ1.*dQ2.*t2.*t7.*t33.*t35.*4.0-Iyy4.*dQ1.*dQ4.*t4.*t9.*t32.*t33.*4.0+Iyy6.*dQ1.*dQ2.*t2.*t7.*t33.*t36.*8.0-Iyy6.*dQ1.*dQ2.*t2.*t7.*t34.*t35.*2.0+Iyy6.*dQ1.*dQ2.*t3.*t8.*t32.*t35.*4.0+Iyy6.*dQ1.*dQ3.*t2.*t7.*t33.*t35.*4.0-Iyy5.*dQ1.*dQ4.*t4.*t9.*t32.*t33.*4.0+Iyy6.*dQ1.*dQ2.*t2.*t7.*t34.*t36.*2.0+Iyy6.*dQ1.*dQ2.*t3.*t8.*t32.*t36.*8.0+Iyy6.*dQ1.*dQ3.*t2.*t7.*t33.*t36.*8.0-Iyy6.*dQ1.*dQ3.*t2.*t7.*t34.*t35.*2.0+Iyy6.*dQ1.*dQ3.*t3.*t8.*t32.*t35.*4.0+Iyy6.*dQ1.*dQ2.*t2.*t7.*t35.*t36.*2.0-Iyy6.*dQ1.*dQ2.*t3.*t8.*t34.*t35.*2.0+Iyy6.*dQ1.*dQ3.*t2.*t7.*t34.*t36.*2.0+Iyy6.*dQ1.*dQ3.*t3.*t8.*t32.*t36.*8.0+Iyy6.*dQ1.*dQ2.*t3.*t8.*t34.*t36.*2.0+Iyy6.*dQ1.*dQ3.*t2.*t7.*t35.*t36.*2.0-Iyy6.*dQ1.*dQ3.*t3.*t8.*t34.*t35.*2.0+Iyy6.*dQ1.*dQ2.*t3.*t8.*t35.*t36.*2.0+Iyy6.*dQ1.*dQ3.*t3.*t8.*t34.*t36.*2.0;
et73 = Iyy6.*dQ1.*dQ4.*t4.*t9.*t32.*t35.*-2.0-Iyy6.*dQ2.*dQ4.*t2.*t8.*t34.*t35.*2.0-Iyy6.*dQ2.*dQ4.*t3.*t7.*t34.*t35.*2.0+Iyy6.*dQ1.*dQ3.*t3.*t8.*t35.*t36.*2.0+Iyy6.*dQ1.*dQ4.*t4.*t9.*t32.*t36.*2.0-Iyy6.*dQ1.*dQ4.*t4.*t9.*t33.*t35.*2.0+Iyy6.*dQ1.*dQ5.*t5.*t10.*t32.*t33.*4.0+Iyy6.*dQ2.*dQ4.*t2.*t8.*t34.*t36.*2.0+Iyy6.*dQ2.*dQ4.*t3.*t7.*t34.*t36.*2.0-Iyy6.*dQ3.*dQ4.*t2.*t8.*t34.*t35.*2.0-Iyy6.*dQ3.*dQ4.*t3.*t7.*t34.*t35.*2.0+Iyy6.*dQ1.*dQ4.*t4.*t9.*t33.*t36.*2.0-Iyy6.*dQ1.*dQ5.*t5.*t10.*t32.*t34.*2.0-Iyy6.*dQ2.*dQ4.*t2.*t8.*t35.*t36.*2.0-Iyy6.*dQ2.*dQ4.*t3.*t7.*t35.*t36.*2.0+Iyy6.*dQ3.*dQ4.*t2.*t8.*t34.*t36.*2.0+Iyy6.*dQ3.*dQ4.*t3.*t7.*t34.*t36.*2.0-Iyy6.*dQ1.*dQ5.*t5.*t10.*t33.*t34.*2.0-Iyy6.*dQ3.*dQ4.*t2.*t8.*t35.*t36.*2.0-Iyy6.*dQ3.*dQ4.*t3.*t7.*t35.*t36.*2.0;
et74 = Iyy6.*dQ1.*dQ5.*t5.*t10.*t32.*t36.*2.0+Iyy6.*dQ1.*dQ6.*t6.*t11.*t32.*t33.*8.0+Iyy6.*dQ1.*dQ5.*t5.*t10.*t33.*t36.*2.0+Iyy6.*dQ1.*dQ6.*t6.*t11.*t32.*t34.*2.0+Iyy6.*dQ1.*dQ6.*t6.*t11.*t32.*t35.*2.0+Iyy6.*dQ1.*dQ6.*t6.*t11.*t33.*t34.*2.0+Iyy6.*dQ1.*dQ6.*t6.*t11.*t33.*t35.*2.0+Iyz5.*dQ1.*dQ4.*t2.*t4.*t5.*t7+Iyz5.*dQ2.*dQ3.*t2.*t4.*t5.*t8+Iyz5.*dQ2.*dQ3.*t3.*t4.*t5.*t7+Iyz5.*dQ1.*dQ4.*t3.*t4.*t5.*t8+Iyz5.*dQ2.*dQ5.*t2.*t3.*t4.*t10+Iyz5.*dQ3.*dQ5.*t2.*t3.*t4.*t10-Iyz6.*dQ1.*dQ6.*t2.*t4.*t6.*t7-Iyz6.*dQ2.*dQ3.*t2.*t3.*t6.*t10-Iyz6.*dQ1.*dQ6.*t3.*t4.*t6.*t8-Iyz6.*dQ2.*dQ6.*t2.*t3.*t6.*t9-Iyz6.*dQ3.*dQ6.*t2.*t3.*t6.*t9-Iyz5.*dQ1.*dQ5.*t2.*t7.*t9.*t10+Iyz6.*dQ1.*dQ4.*t2.*t7.*t9.*t11-Iyz5.*dQ1.*dQ5.*t3.*t8.*t9.*t10-Iyz5.*dQ2.*dQ5.*t4.*t7.*t8.*t10;
et75 = Iyz6.*dQ2.*dQ3.*t2.*t8.*t9.*t11+Iyz6.*dQ2.*dQ3.*t3.*t7.*t9.*t11-Iyz5.*dQ3.*dQ5.*t4.*t7.*t8.*t10+Iyz6.*dQ1.*dQ4.*t3.*t8.*t9.*t11+Iyz6.*dQ2.*dQ3.*t6.*t7.*t8.*t10+Iyz6.*dQ2.*dQ6.*t6.*t7.*t8.*t9+Iyz6.*dQ2.*dQ6.*t2.*t8.*t10.*t11+Iyz6.*dQ2.*dQ6.*t3.*t7.*t10.*t11+Iyz6.*dQ3.*dQ6.*t6.*t7.*t8.*t9+Iyz6.*dQ3.*dQ6.*t2.*t8.*t10.*t11+Iyz6.*dQ3.*dQ6.*t3.*t7.*t10.*t11-Iyz4.*dQ1.*dQ4.*t2.*t4.*t7.*t33.*2.0-Iyz4.*dQ1.*dQ4.*t3.*t4.*t8.*t32.*2.0+Iyz5.*dQ2.*dQ3.*t2.*t3.*t10.*t34.*2.0+Iyz5.*dQ1.*dQ5.*t4.*t5.*t9.*t32+Iyz5.*dQ2.*dQ5.*t2.*t5.*t8.*t34+Iyz5.*dQ2.*dQ5.*t3.*t5.*t7.*t34+Iyz6.*dQ1.*dQ2.*t5.*t6.*t9.*t32.*2.0+Iyz5.*dQ1.*dQ5.*t4.*t5.*t9.*t33+Iyz5.*dQ3.*dQ5.*t2.*t5.*t8.*t34+Iyz5.*dQ3.*dQ5.*t3.*t5.*t7.*t34+Iyz6.*dQ1.*dQ2.*t5.*t6.*t9.*t33.*2.0+Iyz6.*dQ1.*dQ3.*t5.*t6.*t9.*t32.*2.0;
et76 = Iyz6.*dQ1.*dQ3.*t5.*t6.*t9.*t33.*2.0+Iyz6.*dQ1.*dQ6.*t5.*t6.*t10.*t32-Iyz6.*dQ4.*dQ5.*t2.*t3.*t11.*t35.*2.0+Iyz6.*dQ1.*dQ6.*t5.*t6.*t10.*t33-Iyz5.*dQ2.*dQ3.*t7.*t8.*t10.*t34.*2.0+Iyz6.*dQ4.*dQ5.*t7.*t8.*t11.*t35.*2.0-Iyz5.*dQ1.*dQ2.*t5.*t9.*t32.*t33.*4.0-Iyz5.*dQ1.*dQ3.*t5.*t9.*t32.*t33.*4.0+Iyz6.*dQ1.*dQ2.*t4.*t11.*t32.*t33.*4.0+Iyz6.*dQ1.*dQ3.*t4.*t11.*t32.*t33.*4.0+Iyz6.*dQ1.*dQ2.*t4.*t11.*t32.*t35.*4.0+Iyz6.*dQ1.*dQ2.*t4.*t11.*t33.*t35.*4.0+Iyz6.*dQ1.*dQ3.*t4.*t11.*t32.*t35.*4.0+Iyz6.*dQ1.*dQ4.*t6.*t10.*t32.*t33.*2.0+Iyz6.*dQ1.*dQ3.*t4.*t11.*t33.*t35.*4.0+Iyz6.*dQ1.*dQ4.*t6.*t10.*t32.*t34.*2.0+Iyz6.*dQ1.*dQ4.*t6.*t10.*t33.*t34.*2.0-Iyz5.*dQ1.*dQ4.*t10.*t32.*t33.*t34.*4.0+Iyz6.*dQ1.*dQ5.*t11.*t32.*t33.*t34.*2.0-Iyz6.*dQ1.*dQ5.*t11.*t32.*t33.*t35.*4.0+Iyz6.*dQ1.*dQ5.*t11.*t32.*t34.*t35.*2.0;
et77 = Iyz6.*dQ1.*dQ5.*t11.*t33.*t34.*t35.*2.0-Izx3.*dQ1.*dQ2.*t2.*t3.*t7.*t8.*4.0-Izx3.*dQ1.*dQ3.*t2.*t3.*t7.*t8.*4.0+Izx5.*dQ1.*dQ5.*t2.*t3.*t7.*t8.*2.0+Izx5.*dQ1.*dQ2.*t2.*t5.*t7.*t10.*2.0+Izx5.*dQ1.*dQ3.*t2.*t5.*t7.*t10.*2.0+Izx5.*dQ1.*dQ2.*t3.*t5.*t8.*t10.*2.0+Izx5.*dQ1.*dQ3.*t3.*t5.*t8.*t10.*2.0-Izx6.*dQ1.*dQ4.*t2.*t6.*t7.*t9-Izx5.*dQ2.*dQ4.*t2.*t5.*t8.*t10.*2.0-Izx5.*dQ2.*dQ4.*t3.*t5.*t7.*t10.*2.0-Izx6.*dQ2.*dQ3.*t2.*t6.*t8.*t9-Izx6.*dQ2.*dQ3.*t3.*t6.*t7.*t9-Izx5.*dQ3.*dQ4.*t2.*t5.*t8.*t10.*2.0-Izx5.*dQ3.*dQ4.*t3.*t5.*t7.*t10.*2.0-Izx6.*dQ1.*dQ4.*t3.*t6.*t8.*t9-Izx6.*dQ1.*dQ6.*t2.*t4.*t7.*t11-Izx6.*dQ2.*dQ3.*t2.*t3.*t10.*t11-Izx6.*dQ1.*dQ6.*t3.*t4.*t8.*t11-Izx6.*dQ2.*dQ6.*t2.*t3.*t9.*t11;
et78 = -Izx6.*dQ2.*dQ6.*t2.*t6.*t8.*t10-Izx6.*dQ2.*dQ6.*t3.*t6.*t7.*t10-Izx6.*dQ3.*dQ6.*t2.*t3.*t9.*t11-Izx6.*dQ3.*dQ6.*t2.*t6.*t8.*t10-Izx6.*dQ3.*dQ6.*t3.*t6.*t7.*t10+Izx6.*dQ2.*dQ3.*t7.*t8.*t10.*t11+Izx6.*dQ2.*dQ6.*t7.*t8.*t9.*t11+Izx6.*dQ3.*dQ6.*t7.*t8.*t9.*t11-Izx4.*dQ1.*dQ4.*t2.*t7.*t9.*t33.*2.0-Izx4.*dQ1.*dQ4.*t3.*t8.*t9.*t32.*2.0+Izx5.*dQ1.*dQ4.*t2.*t7.*t9.*t33.*2.0+Izx6.*dQ4.*dQ5.*t2.*t3.*t6.*t35.*2.0+Izx5.*dQ1.*dQ4.*t3.*t8.*t9.*t32.*2.0+Izx5.*dQ1.*dQ4.*t2.*t7.*t9.*t35.*2.0+Izx5.*dQ2.*dQ3.*t2.*t8.*t9.*t35.*2.0+Izx5.*dQ2.*dQ3.*t3.*t7.*t9.*t35.*2.0+Izx5.*dQ1.*dQ4.*t3.*t8.*t9.*t35.*2.0+Izx6.*dQ1.*dQ2.*t5.*t9.*t11.*t32.*2.0+Izx6.*dQ1.*dQ2.*t5.*t9.*t11.*t33.*2.0+Izx6.*dQ1.*dQ3.*t5.*t9.*t11.*t32.*2.0+Izx6.*dQ1.*dQ3.*t5.*t9.*t11.*t33.*2.0;
et79 = Izx6.*dQ1.*dQ6.*t5.*t10.*t11.*t32-Izx6.*dQ4.*dQ5.*t6.*t7.*t8.*t35.*2.0+Izx6.*dQ1.*dQ6.*t5.*t10.*t11.*t33-Izx6.*dQ1.*dQ2.*t4.*t6.*t32.*t33.*4.0-Izx6.*dQ1.*dQ3.*t4.*t6.*t32.*t33.*4.0-Izx6.*dQ1.*dQ2.*t4.*t6.*t32.*t35.*4.0-Izx6.*dQ1.*dQ2.*t4.*t6.*t33.*t35.*4.0-Izx6.*dQ1.*dQ3.*t4.*t6.*t32.*t35.*4.0-Izx6.*dQ1.*dQ3.*t4.*t6.*t33.*t35.*4.0+Izx6.*dQ1.*dQ4.*t10.*t11.*t32.*t33.*2.0+Izx6.*dQ1.*dQ4.*t10.*t11.*t32.*t34.*2.0+Izx6.*dQ1.*dQ4.*t10.*t11.*t33.*t34.*2.0+Izx5.*dQ1.*dQ2.*t4.*t32.*t33.*t35.*8.0+Izx5.*dQ1.*dQ3.*t4.*t32.*t33.*t35.*8.0-Izx6.*dQ1.*dQ5.*t6.*t32.*t33.*t34.*2.0+Izx6.*dQ1.*dQ5.*t6.*t32.*t33.*t35.*4.0-Izx6.*dQ1.*dQ5.*t6.*t32.*t34.*t35.*2.0-Izx6.*dQ1.*dQ5.*t6.*t33.*t34.*t35.*2.0+Izx5.*dQ1.*dQ5.*t32.*t33.*t34.*t35.*4.0+Izy5.*dQ1.*dQ4.*t2.*t4.*t5.*t7+Izy5.*dQ2.*dQ3.*t2.*t4.*t5.*t8;
et80 = Izy5.*dQ2.*dQ3.*t3.*t4.*t5.*t7+Izy5.*dQ1.*dQ4.*t3.*t4.*t5.*t8+Izy5.*dQ2.*dQ5.*t2.*t3.*t4.*t10+Izy5.*dQ3.*dQ5.*t2.*t3.*t4.*t10-Izy6.*dQ1.*dQ6.*t2.*t4.*t6.*t7-Izy6.*dQ2.*dQ3.*t2.*t3.*t6.*t10-Izy6.*dQ1.*dQ6.*t3.*t4.*t6.*t8-Izy6.*dQ2.*dQ6.*t2.*t3.*t6.*t9-Izy6.*dQ3.*dQ6.*t2.*t3.*t6.*t9-Izy5.*dQ1.*dQ5.*t2.*t7.*t9.*t10+Izy6.*dQ1.*dQ4.*t2.*t7.*t9.*t11-Izy5.*dQ1.*dQ5.*t3.*t8.*t9.*t10-Izy5.*dQ2.*dQ5.*t4.*t7.*t8.*t10+Izy6.*dQ2.*dQ3.*t2.*t8.*t9.*t11+Izy6.*dQ2.*dQ3.*t3.*t7.*t9.*t11-Izy5.*dQ3.*dQ5.*t4.*t7.*t8.*t10+Izy6.*dQ1.*dQ4.*t3.*t8.*t9.*t11+Izy6.*dQ2.*dQ3.*t6.*t7.*t8.*t10+Izy6.*dQ2.*dQ6.*t6.*t7.*t8.*t9+Izy6.*dQ2.*dQ6.*t2.*t8.*t10.*t11+Izy6.*dQ2.*dQ6.*t3.*t7.*t10.*t11+Izy6.*dQ3.*dQ6.*t6.*t7.*t8.*t9;
et81 = Izy6.*dQ3.*dQ6.*t2.*t8.*t10.*t11+Izy6.*dQ3.*dQ6.*t3.*t7.*t10.*t11-Izy4.*dQ1.*dQ4.*t2.*t4.*t7.*t33.*2.0-Izy4.*dQ1.*dQ4.*t3.*t4.*t8.*t32.*2.0+Izy5.*dQ2.*dQ3.*t2.*t3.*t10.*t34.*2.0+Izy5.*dQ1.*dQ5.*t4.*t5.*t9.*t32+Izy5.*dQ2.*dQ5.*t2.*t5.*t8.*t34+Izy5.*dQ2.*dQ5.*t3.*t5.*t7.*t34+Izy6.*dQ1.*dQ2.*t5.*t6.*t9.*t32.*2.0+Izy5.*dQ1.*dQ5.*t4.*t5.*t9.*t33+Izy5.*dQ3.*dQ5.*t2.*t5.*t8.*t34+Izy5.*dQ3.*dQ5.*t3.*t5.*t7.*t34+Izy6.*dQ1.*dQ2.*t5.*t6.*t9.*t33.*2.0+Izy6.*dQ1.*dQ3.*t5.*t6.*t9.*t32.*2.0+Izy6.*dQ1.*dQ3.*t5.*t6.*t9.*t33.*2.0+Izy6.*dQ1.*dQ6.*t5.*t6.*t10.*t32-Izy6.*dQ4.*dQ5.*t2.*t3.*t11.*t35.*2.0+Izy6.*dQ1.*dQ6.*t5.*t6.*t10.*t33-Izy5.*dQ2.*dQ3.*t7.*t8.*t10.*t34.*2.0+Izy6.*dQ4.*dQ5.*t7.*t8.*t11.*t35.*2.0-Izy5.*dQ1.*dQ2.*t5.*t9.*t32.*t33.*4.0-Izy5.*dQ1.*dQ3.*t5.*t9.*t32.*t33.*4.0;
et82 = Izy6.*dQ1.*dQ2.*t4.*t11.*t32.*t33.*4.0+Izy6.*dQ1.*dQ3.*t4.*t11.*t32.*t33.*4.0+Izy6.*dQ1.*dQ2.*t4.*t11.*t32.*t35.*4.0+Izy6.*dQ1.*dQ2.*t4.*t11.*t33.*t35.*4.0+Izy6.*dQ1.*dQ3.*t4.*t11.*t32.*t35.*4.0+Izy6.*dQ1.*dQ4.*t6.*t10.*t32.*t33.*2.0+Izy6.*dQ1.*dQ3.*t4.*t11.*t33.*t35.*4.0+Izy6.*dQ1.*dQ4.*t6.*t10.*t32.*t34.*2.0+Izy6.*dQ1.*dQ4.*t6.*t10.*t33.*t34.*2.0-Izy5.*dQ1.*dQ4.*t10.*t32.*t33.*t34.*4.0+Izy6.*dQ1.*dQ5.*t11.*t32.*t33.*t34.*2.0-Izy6.*dQ1.*dQ5.*t11.*t32.*t33.*t35.*4.0+Izy6.*dQ1.*dQ5.*t11.*t32.*t34.*t35.*2.0+Izy6.*dQ1.*dQ5.*t11.*t33.*t34.*t35.*2.0-Izz5.*dQ2.*dQ3.*t2.*t3.*t4.*t9.*2.0-Izz6.*dQ2.*dQ3.*t2.*t3.*t4.*t9.*2.0-Izz6.*dQ2.*dQ6.*t2.*t3.*t4.*t10-Izz5.*dQ4.*dQ5.*t2.*t3.*t5.*t10.*2.0-Izz6.*dQ3.*dQ6.*t2.*t3.*t4.*t10-Izz6.*dQ4.*dQ5.*t2.*t3.*t5.*t10.*2.0-Izz6.*dQ5.*dQ6.*t2.*t4.*t5.*t8;
et83 = -Izz6.*dQ5.*dQ6.*t3.*t4.*t5.*t7+Izz5.*dQ2.*dQ3.*t4.*t7.*t8.*t9.*2.0+Izz6.*dQ2.*dQ3.*t4.*t7.*t8.*t9.*2.0+Izz6.*dQ2.*dQ6.*t4.*t7.*t8.*t10+Izz5.*dQ4.*dQ5.*t5.*t7.*t8.*t10.*2.0+Izz6.*dQ3.*dQ6.*t4.*t7.*t8.*t10+Izz6.*dQ4.*dQ5.*t5.*t7.*t8.*t10.*2.0+Izz6.*dQ4.*dQ6.*t2.*t8.*t9.*t10+Izz6.*dQ4.*dQ6.*t3.*t7.*t9.*t10+Izz5.*dQ1.*dQ5.*t2.*t4.*t7.*t33.*4.0+Izz5.*dQ1.*dQ5.*t3.*t4.*t8.*t32.*4.0+Izz6.*dQ1.*dQ5.*t2.*t4.*t7.*t33.*4.0+Izz5.*dQ1.*dQ2.*t4.*t5.*t10.*t32.*4.0+Izz5.*dQ1.*dQ5.*t2.*t4.*t7.*t35.*4.0+Izz6.*dQ1.*dQ5.*t3.*t4.*t8.*t32.*4.0+Izz5.*dQ1.*dQ2.*t4.*t5.*t10.*t33.*4.0+Izz5.*dQ1.*dQ3.*t4.*t5.*t10.*t32.*4.0+Izz6.*dQ1.*dQ2.*t4.*t5.*t10.*t32.*4.0+Izz6.*dQ1.*dQ5.*t2.*t4.*t7.*t35.*4.0+Izz5.*dQ1.*dQ3.*t4.*t5.*t10.*t33.*4.0+Izz5.*dQ1.*dQ5.*t3.*t4.*t8.*t35.*4.0+Izz5.*dQ2.*dQ5.*t2.*t3.*t9.*t35.*2.0;
et84 = Izz6.*dQ1.*dQ2.*t4.*t5.*t10.*t33.*4.0+Izz6.*dQ1.*dQ3.*t4.*t5.*t10.*t32.*4.0+Izz5.*dQ3.*dQ5.*t2.*t3.*t9.*t35.*2.0+Izz6.*dQ1.*dQ3.*t4.*t5.*t10.*t33.*4.0+Izz6.*dQ1.*dQ5.*t3.*t4.*t8.*t35.*4.0+Izz6.*dQ2.*dQ5.*t2.*t3.*t9.*t35.*2.0-Izz5.*dQ4.*dQ5.*t2.*t4.*t8.*t35.*2.0-Izz5.*dQ4.*dQ5.*t3.*t4.*t7.*t35.*2.0+Izz6.*dQ3.*dQ5.*t2.*t3.*t9.*t35.*2.0-Izz6.*dQ4.*dQ5.*t2.*t4.*t8.*t35.*2.0-Izz6.*dQ4.*dQ5.*t3.*t4.*t7.*t35.*2.0-Izz5.*dQ2.*dQ5.*t7.*t8.*t9.*t35.*2.0-Izz5.*dQ3.*dQ5.*t7.*t8.*t9.*t35.*2.0-Izz6.*dQ2.*dQ5.*t7.*t8.*t9.*t35.*2.0-Izz6.*dQ3.*dQ5.*t7.*t8.*t9.*t35.*2.0+Izz5.*dQ1.*dQ2.*t2.*t7.*t33.*t34.*4.0-Izz5.*dQ1.*dQ2.*t2.*t7.*t33.*t35.*4.0+Izz5.*dQ1.*dQ2.*t3.*t8.*t32.*t34.*4.0+Izz5.*dQ1.*dQ3.*t2.*t7.*t33.*t34.*4.0+Izz6.*dQ1.*dQ2.*t2.*t7.*t33.*t34.*4.0+Izz5.*dQ1.*dQ2.*t2.*t7.*t34.*t35.*2.0;
et85 = Izz5.*dQ1.*dQ2.*t3.*t8.*t32.*t35.*-4.0-Izz5.*dQ1.*dQ3.*t2.*t7.*t33.*t35.*4.0+Izz5.*dQ1.*dQ3.*t3.*t8.*t32.*t34.*4.0-Izz6.*dQ1.*dQ2.*t2.*t7.*t33.*t35.*4.0+Izz6.*dQ1.*dQ2.*t3.*t8.*t32.*t34.*4.0+Izz6.*dQ1.*dQ3.*t2.*t7.*t33.*t34.*4.0+Izz5.*dQ1.*dQ3.*t2.*t7.*t34.*t35.*2.0-Izz5.*dQ1.*dQ3.*t3.*t8.*t32.*t35.*4.0+Izz6.*dQ1.*dQ2.*t2.*t7.*t34.*t35.*2.0-Izz6.*dQ1.*dQ2.*t3.*t8.*t32.*t35.*4.0-Izz6.*dQ1.*dQ3.*t2.*t7.*t33.*t35.*4.0+Izz6.*dQ1.*dQ3.*t3.*t8.*t32.*t34.*4.0+Izz5.*dQ1.*dQ2.*t3.*t8.*t34.*t35.*2.0+Izz5.*dQ1.*dQ4.*t4.*t9.*t32.*t33.*4.0+Izz6.*dQ1.*dQ3.*t2.*t7.*t34.*t35.*2.0-Izz6.*dQ1.*dQ3.*t3.*t8.*t32.*t35.*4.0+Izz5.*dQ1.*dQ3.*t3.*t8.*t34.*t35.*2.0+Izz6.*dQ1.*dQ2.*t3.*t8.*t34.*t35.*2.0+Izz6.*dQ1.*dQ4.*t4.*t9.*t32.*t33.*4.0+Izz5.*dQ1.*dQ4.*t4.*t9.*t32.*t35.*2.0+Izz5.*dQ2.*dQ4.*t2.*t8.*t34.*t35.*2.0;
et86 = Izz5.*dQ2.*dQ4.*t3.*t7.*t34.*t35.*2.0+Izz6.*dQ1.*dQ3.*t3.*t8.*t34.*t35.*2.0+Izz5.*dQ1.*dQ4.*t4.*t9.*t33.*t35.*2.0-Izz5.*dQ1.*dQ5.*t5.*t10.*t32.*t33.*4.0+Izz5.*dQ3.*dQ4.*t2.*t8.*t34.*t35.*2.0+Izz5.*dQ3.*dQ4.*t3.*t7.*t34.*t35.*2.0+Izz6.*dQ1.*dQ4.*t4.*t9.*t32.*t35.*2.0+Izz6.*dQ2.*dQ4.*t2.*t8.*t34.*t35.*2.0+Izz6.*dQ2.*dQ4.*t3.*t7.*t34.*t35.*2.0+Izz5.*dQ1.*dQ5.*t5.*t10.*t32.*t34.*2.0+Izz6.*dQ1.*dQ4.*t4.*t9.*t33.*t35.*2.0-Izz6.*dQ1.*dQ5.*t5.*t10.*t32.*t33.*4.0+Izz6.*dQ3.*dQ4.*t2.*t8.*t34.*t35.*2.0+Izz6.*dQ3.*dQ4.*t3.*t7.*t34.*t35.*2.0+Izz5.*dQ1.*dQ5.*t5.*t10.*t33.*t34.*2.0+Izz6.*dQ1.*dQ5.*t5.*t10.*t32.*t34.*2.0+Izz6.*dQ1.*dQ5.*t5.*t10.*t33.*t34.*2.0-dQ1.*dQ5.*m5.*t2.*t4.*t7.*t16.*2.0-dQ1.*dQ5.*m5.*t3.*t4.*t8.*t16.*2.0-dQ1.*dQ2.*m5.*t4.*t5.*t10.*t16.*2.0-dQ1.*dQ3.*m5.*t4.*t5.*t10.*t16.*2.0;
et87 = dQ4.*dQ5.*m5.*t2.*t4.*t8.*t16.*2.0+dQ4.*dQ5.*m5.*t3.*t4.*t7.*t16.*2.0-dQ1.*dQ5.*m6.*t2.*t4.*t7.*t20.*2.0+dQ1.*dQ5.*m6.*t2.*t4.*t7.*t22.*2.0-dQ1.*dQ5.*m6.*t3.*t4.*t8.*t20.*2.0-dQ1.*dQ2.*m6.*t4.*t5.*t10.*t20.*2.0-dQ1.*dQ3.*m6.*t4.*t5.*t10.*t20.*2.0+dQ1.*dQ5.*m5.*t2.*t4.*t7.*t25.*2.0+dQ1.*dQ5.*m6.*t3.*t4.*t8.*t22.*2.0+dQ2.*dQ5.*m6.*t2.*t3.*t9.*t22.*2.0-dQ2.*dQ6.*m6.*t2.*t5.*t8.*t20.*2.0-dQ2.*dQ6.*m6.*t3.*t5.*t7.*t20.*2.0+dQ4.*dQ5.*m6.*t2.*t4.*t8.*t20.*2.0+dQ4.*dQ5.*m6.*t3.*t4.*t7.*t20.*2.0-dQ5.*dQ6.*m6.*t2.*t3.*t10.*t17.*2.0+dQ1.*dQ2.*m6.*t4.*t5.*t10.*t22.*2.0+dQ3.*dQ5.*m6.*t2.*t3.*t9.*t22.*2.0-dQ3.*dQ6.*m6.*t2.*t5.*t8.*t20.*2.0-dQ3.*dQ6.*m6.*t3.*t5.*t7.*t20.*2.0+dQ1.*dQ3.*m6.*t4.*t5.*t10.*t22.*2.0+dQ1.*dQ5.*m5.*t3.*t4.*t8.*t25.*2.0;
et88 = dQ1.*dQ5.*m6.*t2.*t4.*t7.*t26.*2.0+dQ2.*dQ5.*m5.*t2.*t3.*t9.*t25.*2.0+dQ1.*dQ2.*m5.*t4.*t5.*t10.*t25.*2.0+dQ3.*dQ5.*m5.*t2.*t3.*t9.*t25.*2.0+dQ1.*dQ3.*m5.*t4.*t5.*t10.*t25.*2.0+dQ1.*dQ5.*m6.*t3.*t4.*t8.*t26.*2.0+dQ2.*dQ5.*m6.*t2.*t3.*t9.*t26.*2.0+dQ1.*dQ2.*m6.*t4.*t5.*t10.*t26.*2.0+dQ3.*dQ5.*m6.*t2.*t3.*t9.*t26.*2.0+dQ1.*dQ3.*m6.*t4.*t5.*t10.*t26.*2.0-dQ2.*dQ5.*m6.*t7.*t8.*t9.*t22.*2.0+dQ5.*dQ6.*m6.*t7.*t8.*t10.*t17.*2.0-dQ3.*dQ5.*m6.*t7.*t8.*t9.*t22.*2.0-dQ2.*dQ5.*m5.*t7.*t8.*t9.*t25.*2.0-dQ1.*dQ2.*m3.*t2.*t7.*t14.*t33.*4.0-dQ1.*dQ2.*m4.*t2.*t7.*t13.*t33.*4.0-dQ3.*dQ5.*m5.*t7.*t8.*t9.*t25.*2.0-dQ1.*dQ2.*m3.*t3.*t8.*t14.*t32.*4.0-dQ1.*dQ2.*m4.*t3.*t8.*t13.*t32.*4.0-dQ1.*dQ2.*m5.*t2.*t7.*t13.*t33.*4.0-dQ1.*dQ3.*m3.*t2.*t7.*t14.*t33.*4.0;
et89 = dQ1.*dQ3.*m4.*t2.*t7.*t13.*t33.*-4.0-dQ2.*dQ5.*m6.*t7.*t8.*t9.*t26.*2.0-dQ1.*dQ2.*m5.*t3.*t8.*t13.*t32.*4.0-dQ1.*dQ2.*m6.*t2.*t7.*t13.*t33.*4.0-dQ1.*dQ3.*m3.*t3.*t8.*t14.*t32.*4.0-dQ1.*dQ3.*m4.*t3.*t8.*t13.*t32.*4.0-dQ1.*dQ3.*m5.*t2.*t7.*t13.*t33.*4.0-dQ3.*dQ5.*m6.*t7.*t8.*t9.*t26.*2.0+dQ1.*dQ2.*m4.*t2.*t7.*t15.*t34.*2.0-dQ1.*dQ2.*m6.*t3.*t8.*t13.*t32.*4.0-dQ1.*dQ3.*m5.*t3.*t8.*t13.*t32.*4.0-dQ1.*dQ3.*m6.*t2.*t7.*t13.*t33.*4.0+dQ1.*dQ2.*m5.*t2.*t7.*t16.*t33.*4.0+dQ1.*dQ3.*m4.*t2.*t7.*t15.*t34.*2.0-dQ1.*dQ3.*m6.*t3.*t8.*t13.*t32.*4.0-dQ1.*dQ2.*m4.*t2.*t7.*t18.*t33.*4.0+dQ1.*dQ2.*m4.*t3.*t8.*t15.*t34.*2.0+dQ1.*dQ2.*m5.*t3.*t8.*t16.*t32.*4.0+dQ1.*dQ3.*m5.*t2.*t7.*t16.*t33.*4.0-dQ1.*dQ2.*m4.*t2.*t7.*t18.*t34.*2.0;
et90 = dQ1.*dQ2.*m4.*t3.*t8.*t18.*t32.*-4.0+dQ1.*dQ2.*m5.*t2.*t7.*t16.*t35.*2.0-dQ1.*dQ2.*m6.*t2.*t7.*t17.*t33.*4.0-dQ1.*dQ3.*m4.*t2.*t7.*t18.*t33.*4.0+dQ1.*dQ3.*m4.*t3.*t8.*t15.*t34.*2.0+dQ1.*dQ3.*m5.*t3.*t8.*t16.*t32.*4.0-dQ1.*dQ2.*m5.*t2.*t7.*t19.*t33.*4.0-dQ1.*dQ2.*m6.*t2.*t7.*t17.*t34.*2.0-dQ1.*dQ2.*m6.*t3.*t8.*t17.*t32.*4.0-dQ1.*dQ3.*m4.*t2.*t7.*t18.*t34.*2.0-dQ1.*dQ3.*m4.*t3.*t8.*t18.*t32.*4.0+dQ1.*dQ3.*m5.*t2.*t7.*t16.*t35.*2.0-dQ1.*dQ3.*m6.*t2.*t7.*t17.*t33.*4.0+dQ1.*dQ4.*m4.*t4.*t9.*t15.*t32.*2.0+dQ2.*dQ4.*m4.*t2.*t8.*t15.*t34.*2.0+dQ2.*dQ4.*m4.*t3.*t7.*t15.*t34.*2.0-dQ1.*dQ2.*m4.*t3.*t8.*t18.*t34.*2.0-dQ1.*dQ2.*m5.*t2.*t7.*t19.*t34.*2.0+dQ1.*dQ2.*m5.*t3.*t8.*t16.*t35.*2.0-dQ1.*dQ2.*m5.*t3.*t8.*t19.*t32.*4.0;
et91 = dQ1.*dQ3.*m5.*t2.*t7.*t19.*t33.*-4.0-dQ1.*dQ3.*m6.*t2.*t7.*t17.*t34.*2.0-dQ1.*dQ3.*m6.*t3.*t8.*t17.*t32.*4.0+dQ1.*dQ4.*m4.*t4.*t9.*t15.*t33.*2.0+dQ3.*dQ4.*m4.*t2.*t8.*t15.*t34.*2.0+dQ3.*dQ4.*m4.*t3.*t7.*t15.*t34.*2.0+dQ1.*dQ2.*m3.*t2.*t7.*t23.*t33.*4.0+dQ1.*dQ2.*m5.*t2.*t7.*t21.*t33.*4.0-dQ1.*dQ2.*m6.*t2.*t7.*t17.*t36.*4.0+dQ1.*dQ2.*m6.*t2.*t7.*t20.*t33.*4.0-dQ1.*dQ2.*m6.*t3.*t8.*t17.*t34.*2.0-dQ1.*dQ3.*m4.*t3.*t8.*t18.*t34.*2.0-dQ1.*dQ3.*m5.*t2.*t7.*t19.*t34.*2.0+dQ1.*dQ3.*m5.*t3.*t8.*t16.*t35.*2.0-dQ1.*dQ3.*m5.*t3.*t8.*t19.*t32.*4.0+dQ1.*dQ2.*m3.*t3.*t8.*t23.*t32.*4.0-dQ1.*dQ2.*m5.*t3.*t8.*t19.*t34.*2.0+dQ1.*dQ2.*m5.*t3.*t8.*t21.*t32.*4.0+dQ1.*dQ2.*m6.*t2.*t7.*t21.*t33.*4.0+dQ1.*dQ2.*m6.*t3.*t8.*t20.*t32.*4.0+dQ1.*dQ3.*m3.*t2.*t7.*t23.*t33.*4.0;
et92 = dQ1.*dQ3.*m5.*t2.*t7.*t21.*t33.*4.0-dQ1.*dQ3.*m6.*t2.*t7.*t17.*t36.*4.0+dQ1.*dQ3.*m6.*t2.*t7.*t20.*t33.*4.0-dQ1.*dQ3.*m6.*t3.*t8.*t17.*t34.*2.0-dQ1.*dQ4.*m4.*t4.*t9.*t18.*t32.*2.0-dQ2.*dQ4.*m4.*t2.*t8.*t18.*t34.*2.0-dQ2.*dQ4.*m4.*t3.*t7.*t18.*t34.*2.0-dQ2.*dQ4.*m5.*t2.*t8.*t16.*t35.*2.0-dQ2.*dQ4.*m5.*t3.*t7.*t16.*t35.*2.0+dQ1.*dQ2.*m4.*t2.*t7.*t24.*t33.*4.0+dQ1.*dQ2.*m6.*t2.*t7.*t20.*t35.*2.0-dQ1.*dQ2.*m6.*t3.*t8.*t17.*t36.*4.0+dQ1.*dQ2.*m6.*t3.*t8.*t21.*t32.*4.0+dQ1.*dQ3.*m3.*t3.*t8.*t23.*t32.*4.0-dQ1.*dQ3.*m5.*t3.*t8.*t19.*t34.*2.0+dQ1.*dQ3.*m5.*t3.*t8.*t21.*t32.*4.0+dQ1.*dQ3.*m6.*t2.*t7.*t21.*t33.*4.0+dQ1.*dQ3.*m6.*t3.*t8.*t20.*t32.*4.0-dQ1.*dQ4.*m4.*t4.*t9.*t18.*t33.*2.0-dQ1.*dQ4.*m6.*t4.*t9.*t17.*t32.*2.0;
et93 = dQ2.*dQ4.*m6.*t2.*t8.*t17.*t34.*-2.0-dQ2.*dQ4.*m6.*t3.*t7.*t17.*t34.*2.0-dQ3.*dQ4.*m4.*t2.*t8.*t18.*t34.*2.0-dQ3.*dQ4.*m4.*t3.*t7.*t18.*t34.*2.0-dQ3.*dQ4.*m5.*t2.*t8.*t16.*t35.*2.0-dQ3.*dQ4.*m5.*t3.*t7.*t16.*t35.*2.0+dQ1.*dQ2.*m4.*t3.*t8.*t24.*t32.*4.0+dQ1.*dQ2.*m6.*t2.*t7.*t20.*t36.*4.0+dQ1.*dQ2.*m6.*t2.*t7.*t22.*t34.*2.0+dQ1.*dQ3.*m4.*t2.*t7.*t24.*t33.*4.0+dQ1.*dQ3.*m6.*t2.*t7.*t20.*t35.*2.0-dQ1.*dQ3.*m6.*t3.*t8.*t17.*t36.*4.0+dQ1.*dQ3.*m6.*t3.*t8.*t21.*t32.*4.0-dQ1.*dQ4.*m5.*t4.*t9.*t19.*t32.*2.0-dQ1.*dQ4.*m6.*t4.*t9.*t17.*t33.*2.0+dQ1.*dQ5.*m5.*t5.*t10.*t16.*t32.*2.0-dQ2.*dQ4.*m5.*t2.*t8.*t19.*t34.*2.0-dQ2.*dQ4.*m5.*t3.*t7.*t19.*t34.*2.0-dQ3.*dQ4.*m6.*t2.*t8.*t17.*t34.*2.0-dQ3.*dQ4.*m6.*t3.*t7.*t17.*t34.*2.0;
et94 = dQ1.*dQ2.*m6.*t2.*t7.*t22.*t35.*-2.0+dQ1.*dQ2.*m6.*t3.*t8.*t20.*t35.*2.0+dQ1.*dQ3.*m4.*t3.*t8.*t24.*t32.*4.0+dQ1.*dQ3.*m6.*t2.*t7.*t20.*t36.*4.0+dQ1.*dQ3.*m6.*t2.*t7.*t22.*t34.*2.0-dQ1.*dQ4.*m5.*t4.*t9.*t19.*t33.*2.0+dQ1.*dQ5.*m5.*t5.*t10.*t16.*t33.*2.0-dQ3.*dQ4.*m5.*t2.*t8.*t19.*t34.*2.0-dQ3.*dQ4.*m5.*t3.*t7.*t19.*t34.*2.0+dQ1.*dQ2.*m5.*t2.*t7.*t25.*t34.*2.0+dQ1.*dQ2.*m6.*t3.*t8.*t20.*t36.*4.0+dQ1.*dQ2.*m6.*t3.*t8.*t22.*t34.*2.0-dQ1.*dQ3.*m6.*t2.*t7.*t22.*t35.*2.0+dQ1.*dQ3.*m6.*t3.*t8.*t20.*t35.*2.0-dQ1.*dQ2.*m5.*t2.*t7.*t25.*t35.*2.0-dQ1.*dQ2.*m6.*t3.*t8.*t22.*t35.*2.0+dQ1.*dQ3.*m5.*t2.*t7.*t25.*t34.*2.0+dQ1.*dQ3.*m6.*t3.*t8.*t20.*t36.*4.0+dQ1.*dQ3.*m6.*t3.*t8.*t22.*t34.*2.0-dQ2.*dQ4.*m6.*t2.*t8.*t20.*t35.*2.0-dQ2.*dQ4.*m6.*t3.*t7.*t20.*t35.*2.0;
et95 = dQ1.*dQ2.*m5.*t3.*t8.*t25.*t34.*2.0+dQ1.*dQ2.*m6.*t2.*t7.*t26.*t34.*2.0-dQ1.*dQ3.*m5.*t2.*t7.*t25.*t35.*2.0-dQ1.*dQ3.*m6.*t3.*t8.*t22.*t35.*2.0+dQ1.*dQ4.*m6.*t4.*t9.*t22.*t32.*2.0+dQ2.*dQ4.*m6.*t2.*t8.*t22.*t34.*2.0+dQ2.*dQ4.*m6.*t3.*t7.*t22.*t34.*2.0-dQ3.*dQ4.*m6.*t2.*t8.*t20.*t35.*2.0-dQ3.*dQ4.*m6.*t3.*t7.*t20.*t35.*2.0-dQ1.*dQ2.*m5.*t3.*t8.*t25.*t35.*2.0-dQ1.*dQ2.*m6.*t2.*t7.*t26.*t35.*2.0+dQ1.*dQ3.*m5.*t3.*t8.*t25.*t34.*2.0+dQ1.*dQ3.*m6.*t2.*t7.*t26.*t34.*2.0+dQ1.*dQ4.*m6.*t4.*t9.*t22.*t33.*2.0+dQ1.*dQ5.*m6.*t5.*t10.*t20.*t32.*2.0-dQ1.*dQ6.*m6.*t6.*t11.*t17.*t32.*4.0+dQ2.*dQ4.*m6.*t2.*t8.*t22.*t35.*2.0+dQ2.*dQ4.*m6.*t3.*t7.*t22.*t35.*2.0+dQ3.*dQ4.*m6.*t2.*t8.*t22.*t34.*2.0+dQ3.*dQ4.*m6.*t3.*t7.*t22.*t34.*2.0+dQ1.*dQ2.*m6.*t3.*t8.*t26.*t34.*2.0;
et96 = dQ1.*dQ3.*m5.*t3.*t8.*t25.*t35.*-2.0-dQ1.*dQ3.*m6.*t2.*t7.*t26.*t35.*2.0+dQ1.*dQ4.*m5.*t4.*t9.*t25.*t32.*2.0-dQ1.*dQ5.*m6.*t5.*t10.*t17.*t36.*2.0+dQ1.*dQ5.*m6.*t5.*t10.*t20.*t33.*2.0-dQ1.*dQ6.*m6.*t6.*t11.*t17.*t33.*4.0+dQ2.*dQ4.*m5.*t2.*t8.*t25.*t34.*2.0+dQ2.*dQ4.*m5.*t3.*t7.*t25.*t34.*2.0+dQ3.*dQ4.*m6.*t2.*t8.*t22.*t35.*2.0+dQ3.*dQ4.*m6.*t3.*t7.*t22.*t35.*2.0-dQ1.*dQ2.*m6.*t3.*t8.*t26.*t35.*2.0+dQ1.*dQ3.*m6.*t3.*t8.*t26.*t34.*2.0+dQ1.*dQ4.*m5.*t4.*t9.*t25.*t33.*2.0-dQ1.*dQ5.*m6.*t5.*t10.*t22.*t32.*2.0+dQ2.*dQ4.*m5.*t2.*t8.*t25.*t35.*2.0+dQ2.*dQ4.*m5.*t3.*t7.*t25.*t35.*2.0+dQ3.*dQ4.*m5.*t2.*t8.*t25.*t34.*2.0+dQ3.*dQ4.*m5.*t3.*t7.*t25.*t34.*2.0-dQ1.*dQ3.*m6.*t3.*t8.*t26.*t35.*2.0+dQ1.*dQ4.*m6.*t4.*t9.*t26.*t32.*2.0-dQ1.*dQ5.*m6.*t5.*t10.*t22.*t33.*2.0;
et97 = dQ1.*dQ6.*m6.*t6.*t11.*t17.*t35.*-2.0+dQ1.*dQ6.*m6.*t6.*t11.*t20.*t32.*4.0+dQ2.*dQ4.*m6.*t2.*t8.*t26.*t34.*2.0+dQ2.*dQ4.*m6.*t3.*t7.*t26.*t34.*2.0+dQ3.*dQ4.*m5.*t2.*t8.*t25.*t35.*2.0+dQ3.*dQ4.*m5.*t3.*t7.*t25.*t35.*2.0+dQ1.*dQ4.*m6.*t4.*t9.*t26.*t33.*2.0-dQ1.*dQ5.*m5.*t5.*t10.*t25.*t32.*2.0+dQ1.*dQ5.*m6.*t5.*t10.*t20.*t36.*2.0+dQ1.*dQ6.*m6.*t6.*t11.*t20.*t33.*4.0+dQ2.*dQ4.*m6.*t2.*t8.*t26.*t35.*2.0+dQ2.*dQ4.*m6.*t3.*t7.*t26.*t35.*2.0+dQ3.*dQ4.*m6.*t2.*t8.*t26.*t34.*2.0+dQ3.*dQ4.*m6.*t3.*t7.*t26.*t34.*2.0-dQ1.*dQ5.*m5.*t5.*t10.*t25.*t33.*2.0+dQ3.*dQ4.*m6.*t2.*t8.*t26.*t35.*2.0+dQ3.*dQ4.*m6.*t3.*t7.*t26.*t35.*2.0-dQ1.*dQ5.*m6.*t5.*t10.*t26.*t32.*2.0+dQ1.*dQ6.*m6.*t6.*t11.*t20.*t35.*2.0-dQ1.*dQ5.*m6.*t5.*t10.*t26.*t33.*2.0-t3.*t5.*t6.*t7.*t11.*t34.*t130.*8.0;
et98 = t3.*t5.*t6.*t7.*t11.*t34.*t138.*8.0-t3.*t4.*t7.*t9.*t35.*t36.*t130.*4.0+t3.*t4.*t7.*t9.*t35.*t36.*t138.*4.0+t4.*t6.*t7.*t8.*t10.*t11.*t238.*4.0-t4.*t6.*t7.*t8.*t10.*t11.*t242.*4.0-Lx2.*Lx3.*dQ1.*dQ2.*m4.*t2.*t3.*t7.*4.0-Lx2.*Lx3.*dQ1.*dQ2.*m5.*t2.*t3.*t7.*4.0-Lx2.*Lx3.*dQ1.*dQ3.*m4.*t2.*t3.*t7.*2.0-Lx2.*Lx3.*dQ1.*dQ2.*m6.*t2.*t3.*t7.*4.0-Lx2.*Lx3.*dQ1.*dQ3.*m5.*t2.*t3.*t7.*2.0-Lx2.*Lx3.*dQ1.*dQ3.*m6.*t2.*t3.*t7.*2.0-Lx2.*Lxcm3.*dQ1.*dQ2.*m3.*t2.*t3.*t7.*4.0-Lx2.*Lxcm3.*dQ1.*dQ3.*m3.*t2.*t3.*t7.*2.0+Lx3.*Lxcm4.*dQ1.*dQ2.*m4.*t2.*t4.*t7.*4.0+Lx3.*Lxcm4.*dQ1.*dQ3.*m4.*t2.*t4.*t7.*4.0+Lx3.*Lxcm4.*dQ1.*dQ2.*m4.*t3.*t4.*t8.*4.0+Lx3.*Lxcm4.*dQ1.*dQ3.*m4.*t3.*t4.*t8.*4.0+Lx3.*Lxcm4.*dQ2.*dQ3.*m4.*t2.*t3.*t9.*2.0+Lx2.*Lxcm5.*dQ1.*dQ2.*m5.*t4.*t5.*t8.*2.0;
et99 = Lx3.*Lxcm5.*dQ1.*dQ5.*m5.*t2.*t5.*t7.*2.0+Lx3.*Lxcm5.*dQ1.*dQ5.*m5.*t3.*t5.*t8.*2.0+Lx2.*Lxcm6.*dQ1.*dQ2.*m6.*t3.*t6.*t10.*2.0-Lx2.*Lxcm5.*dQ4.*dQ5.*m5.*t2.*t4.*t10.*2.0-Lx3.*Lxcm4.*dQ2.*dQ3.*m4.*t7.*t8.*t9.*2.0-Lx3.*Lxcm6.*dQ1.*dQ4.*m6.*t5.*t6.*t9.*2.0-Lx2.*Lxcm6.*dQ4.*dQ6.*m6.*t2.*t6.*t9.*2.0-Lx3.*Lxcm6.*dQ1.*dQ5.*m6.*t4.*t6.*t10.*2.0-Lx3.*Lxcm6.*dQ1.*dQ6.*m6.*t4.*t5.*t11.*2.0-Lx2.*Lxcm6.*dQ1.*dQ2.*m6.*t8.*t9.*t11.*2.0-Lx2.*Lxcm4.*dQ1.*dQ2.*m4.*t4.*t8.*t32.*4.0-Lx2.*Lxcm4.*dQ1.*dQ3.*m4.*t4.*t8.*t32.*2.0-Lx2.*Lxcm4.*dQ1.*dQ4.*m4.*t3.*t9.*t32.*2.0-Lx2.*Lxcm5.*dQ1.*dQ2.*m5.*t3.*t10.*t32.*4.0-Lx2.*Lxcm5.*dQ1.*dQ3.*m5.*t3.*t10.*t32.*2.0-Lx2.*Lxcm5.*dQ1.*dQ5.*m5.*t5.*t8.*t32.*2.0+Lx3.*Lxcm5.*dQ1.*dQ4.*m5.*t5.*t9.*t32.*2.0+Lx3.*Lxcm5.*dQ1.*dQ4.*m5.*t5.*t9.*t33.*2.0;
et100 = Lx3.*Lxcm5.*dQ1.*dQ5.*m5.*t4.*t10.*t32.*2.0+Lx3.*Lxcm5.*dQ1.*dQ5.*m5.*t4.*t10.*t33.*2.0+Lx3.*Lxcm6.*dQ1.*dQ2.*m6.*t6.*t10.*t32.*4.0+Lx3.*Lxcm6.*dQ1.*dQ2.*m6.*t6.*t10.*t33.*4.0+Lx3.*Lxcm6.*dQ1.*dQ3.*m6.*t6.*t10.*t32.*4.0+Lx3.*Lxcm6.*dQ1.*dQ4.*m6.*t4.*t11.*t32.*2.0+Lx3.*Lxcm6.*dQ1.*dQ3.*m6.*t6.*t10.*t33.*4.0+Lx3.*Lxcm6.*dQ1.*dQ4.*m6.*t4.*t11.*t33.*2.0+Lx3.*Lxcm6.*dQ1.*dQ6.*m6.*t6.*t9.*t32.*2.0+Lx3.*Lxcm6.*dQ1.*dQ6.*m6.*t6.*t9.*t33.*2.0-Lx3.*Lxcm4.*dQ1.*dQ4.*m4.*t9.*t32.*t33.*4.0-Lx3.*Lxcm5.*dQ1.*dQ2.*m5.*t10.*t32.*t33.*8.0-Lx3.*Lxcm5.*dQ1.*dQ3.*m5.*t10.*t32.*t33.*8.0+Lx3.*Lycm4.*dQ2.*dQ3.*m4.*t2.*t3.*t4.*2.0+Lx3.*Lycm5.*dQ2.*dQ3.*m5.*t2.*t3.*t4.*2.0-Lx3.*Lycm4.*dQ1.*dQ2.*m4.*t2.*t7.*t9.*4.0-Lx3.*Lycm4.*dQ1.*dQ3.*m4.*t2.*t7.*t9.*4.0-Lx3.*Lycm4.*dQ1.*dQ2.*m4.*t3.*t8.*t9.*4.0-Lx3.*Lycm5.*dQ1.*dQ2.*m5.*t2.*t7.*t9.*4.0;
et101 = Lx3.*Lycm4.*dQ1.*dQ3.*m4.*t3.*t8.*t9.*-4.0-Lx3.*Lycm4.*dQ2.*dQ3.*m4.*t4.*t7.*t8.*2.0-Lx3.*Lycm5.*dQ1.*dQ3.*m5.*t2.*t7.*t9.*4.0-Lx3.*Lycm5.*dQ1.*dQ2.*m5.*t3.*t8.*t9.*4.0-Lx3.*Lycm5.*dQ1.*dQ3.*m5.*t3.*t8.*t9.*4.0-Lx3.*Lycm5.*dQ2.*dQ3.*m5.*t4.*t7.*t8.*2.0-Lx3.*Lycm6.*dQ1.*dQ6.*m6.*t4.*t5.*t6.*2.0-Lx2.*Lycm6.*dQ1.*dQ2.*m6.*t6.*t8.*t9.*2.0-Lx2.*Lycm6.*dQ1.*dQ2.*m6.*t3.*t10.*t11.*2.0+Lx3.*Lycm6.*dQ1.*dQ4.*m6.*t5.*t9.*t11.*2.0+Lx2.*Lycm6.*dQ4.*dQ6.*m6.*t2.*t9.*t11.*2.0+Lx3.*Lycm6.*dQ1.*dQ5.*m6.*t4.*t10.*t11.*2.0-Lx2.*Lycm4.*dQ1.*dQ4.*m4.*t3.*t4.*t32.*2.0-Lx2.*Lycm5.*dQ1.*dQ4.*m5.*t3.*t4.*t32.*2.0+Lx2.*Lycm4.*dQ1.*dQ2.*m4.*t8.*t9.*t32.*4.0+Lx3.*Lycm6.*dQ1.*dQ4.*m6.*t4.*t6.*t32.*2.0+Lx2.*Lycm4.*dQ1.*dQ3.*m4.*t8.*t9.*t32.*2.0+Lx3.*Lycm6.*dQ1.*dQ4.*m6.*t4.*t6.*t33.*2.0;
et102 = Lx2.*Lycm5.*dQ1.*dQ2.*m5.*t8.*t9.*t32.*4.0+Lx2.*Lycm5.*dQ1.*dQ3.*m5.*t8.*t9.*t32.*2.0-Lx3.*Lycm6.*dQ1.*dQ2.*m6.*t10.*t11.*t32.*4.0-Lx3.*Lycm6.*dQ1.*dQ2.*m6.*t10.*t11.*t33.*4.0-Lx3.*Lycm6.*dQ1.*dQ3.*m6.*t10.*t11.*t32.*4.0-Lx3.*Lycm6.*dQ1.*dQ3.*m6.*t10.*t11.*t33.*4.0-Lx3.*Lycm6.*dQ1.*dQ6.*m6.*t9.*t11.*t32.*2.0-Lx3.*Lycm6.*dQ1.*dQ6.*m6.*t9.*t11.*t33.*2.0-Lx3.*Lycm4.*dQ1.*dQ4.*m4.*t4.*t32.*t33.*4.0-Lx3.*Lycm5.*dQ1.*dQ4.*m5.*t4.*t32.*t33.*4.0-Lxcm5.*Lycm5.*dQ2.*dQ3.*m5.*t2.*t3.*t5.*2.0+Lxcm6.*Lycm6.*dQ2.*dQ3.*m6.*t2.*t3.*t5.*2.0+Lxcm5.*Lycm5.*dQ2.*dQ3.*m5.*t5.*t7.*t8.*2.0-Lxcm6.*Lycm6.*dQ2.*dQ3.*m6.*t5.*t7.*t8.*2.0+Lxcm6.*Lycm6.*dQ5.*dQ6.*m6.*t2.*t8.*t9.*2.0+Lxcm6.*Lycm6.*dQ5.*dQ6.*m6.*t3.*t7.*t9.*2.0+Lxcm4.*Lycm4.*dQ2.*dQ3.*m4.*t2.*t3.*t34.*4.0-Lxcm4.*Lycm4.*dQ2.*dQ3.*m4.*t7.*t8.*t34.*4.0;
et103 = Lxcm6.*Lycm6.*dQ4.*dQ6.*m6.*t2.*t3.*t35.*2.0-Lxcm5.*Lycm5.*dQ1.*dQ2.*m5.*t9.*t10.*t32.*4.0+Lxcm6.*Lycm6.*dQ4.*dQ6.*m6.*t2.*t3.*t36.*4.0-Lxcm5.*Lycm5.*dQ1.*dQ2.*m5.*t9.*t10.*t33.*4.0-Lxcm5.*Lycm5.*dQ1.*dQ3.*m5.*t9.*t10.*t32.*4.0-Lxcm5.*Lycm5.*dQ1.*dQ3.*m5.*t9.*t10.*t33.*4.0+Lxcm6.*Lycm6.*dQ1.*dQ2.*m6.*t9.*t10.*t32.*4.0+Lxcm6.*Lycm6.*dQ1.*dQ2.*m6.*t9.*t10.*t33.*4.0+Lxcm6.*Lycm6.*dQ1.*dQ3.*m6.*t9.*t10.*t32.*4.0+Lxcm6.*Lycm6.*dQ1.*dQ3.*m6.*t9.*t10.*t33.*4.0+Lxcm6.*Lycm6.*dQ1.*dQ2.*m6.*t9.*t10.*t36.*4.0+Lxcm6.*Lycm6.*dQ1.*dQ3.*m6.*t9.*t10.*t36.*4.0-Lxcm6.*Lycm6.*dQ4.*dQ6.*m6.*t7.*t8.*t35.*2.0-Lxcm6.*Lycm6.*dQ4.*dQ6.*m6.*t7.*t8.*t36.*4.0+Lxcm5.*Lycm5.*dQ1.*dQ4.*m5.*t5.*t32.*t33.*4.0+Lxcm5.*Lycm5.*dQ1.*dQ4.*m5.*t5.*t32.*t34.*4.0+Lxcm5.*Lycm5.*dQ1.*dQ4.*m5.*t5.*t33.*t34.*4.0-Lxcm6.*Lycm6.*dQ1.*dQ4.*m6.*t5.*t32.*t33.*4.0-Lxcm6.*Lycm6.*dQ1.*dQ4.*m6.*t5.*t32.*t34.*4.0;
et104 = Lxcm6.*Lycm6.*dQ1.*dQ4.*m6.*t5.*t33.*t34.*-4.0-Lxcm6.*Lycm6.*dQ1.*dQ4.*m6.*t5.*t32.*t36.*4.0-Lxcm6.*Lycm6.*dQ1.*dQ4.*m6.*t5.*t33.*t36.*4.0-Lxcm4.*Lycm4.*dQ1.*dQ4.*m4.*t32.*t33.*t34.*8.0+Lxcm6.*Lycm6.*dQ1.*dQ6.*m6.*t32.*t33.*t34.*4.0+Lxcm6.*Lycm6.*dQ1.*dQ6.*m6.*t32.*t33.*t35.*4.0+Lxcm6.*Lycm6.*dQ1.*dQ6.*m6.*t32.*t33.*t36.*1.6e+1-Lxcm6.*Lycm6.*dQ1.*dQ6.*m6.*t32.*t34.*t35.*2.0+Lxcm6.*Lycm6.*dQ1.*dQ6.*m6.*t32.*t34.*t36.*4.0-Lxcm6.*Lycm6.*dQ1.*dQ6.*m6.*t33.*t34.*t35.*2.0+Lxcm6.*Lycm6.*dQ1.*dQ6.*m6.*t32.*t35.*t36.*4.0+Lxcm6.*Lycm6.*dQ1.*dQ6.*m6.*t33.*t34.*t36.*4.0+Lxcm6.*Lycm6.*dQ1.*dQ6.*m6.*t33.*t35.*t36.*4.0-Lx2.*Lz4.*dQ1.*dQ2.*m5.*t2.*t7.*t8.*4.0-Lx2.*Lz4.*dQ1.*dQ2.*m6.*t2.*t7.*t8.*4.0-Lx2.*Lz4.*dQ1.*dQ3.*m5.*t2.*t7.*t8.*2.0-Lx2.*Lz4.*dQ1.*dQ3.*m6.*t2.*t7.*t8.*2.0+Lx2.*Lz5.*dQ4.*dQ5.*m6.*t2.*t4.*t5.*2.0;
et105 = Lx2.*Lz5.*dQ1.*dQ2.*m6.*t4.*t8.*t10.*2.0+Lx3.*Lz5.*dQ1.*dQ5.*m6.*t2.*t7.*t10.*2.0+Lx3.*Lz5.*dQ1.*dQ5.*m6.*t3.*t8.*t10.*2.0+Lx2.*Lz5.*dQ1.*dQ2.*m6.*t3.*t5.*t32.*4.0+Lx2.*Lz5.*dQ1.*dQ3.*m6.*t3.*t5.*t32.*2.0-Lx3.*Lz5.*dQ1.*dQ5.*m6.*t4.*t5.*t32.*2.0-Lx3.*Lz5.*dQ1.*dQ5.*m6.*t4.*t5.*t33.*2.0-Lx2.*Lz5.*dQ1.*dQ5.*m6.*t8.*t10.*t32.*2.0+Lx3.*Lz5.*dQ1.*dQ4.*m6.*t9.*t10.*t32.*2.0+Lx3.*Lz5.*dQ1.*dQ4.*m6.*t9.*t10.*t33.*2.0+Lx3.*Lz5.*dQ1.*dQ2.*m6.*t5.*t32.*t33.*8.0+Lx3.*Lz5.*dQ1.*dQ3.*m6.*t5.*t32.*t33.*8.0-Lx2.*Lzcm3.*dQ1.*dQ2.*m3.*t2.*t7.*t8.*4.0-Lx2.*Lzcm3.*dQ1.*dQ3.*m3.*t2.*t7.*t8.*2.0-Lx2.*Lzcm4.*dQ1.*dQ2.*m4.*t2.*t7.*t8.*4.0-Lx2.*Lzcm4.*dQ1.*dQ3.*m4.*t2.*t7.*t8.*2.0+Lx2.*Lzcm5.*dQ4.*dQ5.*m5.*t2.*t4.*t5.*2.0+Lx2.*Lzcm6.*dQ4.*dQ5.*m6.*t2.*t4.*t5.*2.0+Lxcm6.*Lz4.*dQ1.*dQ2.*m6.*t4.*t5.*t6.*2.0;
et106 = Lxcm6.*Lz4.*dQ1.*dQ3.*m6.*t4.*t5.*t6.*2.0+Lxcm5.*Lz4.*dQ1.*dQ2.*m5.*t2.*t7.*t10.*4.0+Lx2.*Lzcm5.*dQ1.*dQ2.*m5.*t4.*t8.*t10.*2.0+Lxcm5.*Lz4.*dQ1.*dQ3.*m5.*t2.*t7.*t10.*4.0-Lxcm6.*Lz5.*dQ4.*dQ5.*m6.*t2.*t3.*t6.*2.0+Lx3.*Lzcm5.*dQ1.*dQ5.*m5.*t2.*t7.*t10.*2.0+Lxcm5.*Lz4.*dQ1.*dQ2.*m5.*t3.*t8.*t10.*4.0+Lx2.*Lzcm6.*dQ1.*dQ2.*m6.*t4.*t8.*t10.*2.0+Lxcm5.*Lz4.*dQ1.*dQ3.*m5.*t3.*t8.*t10.*4.0+Lx3.*Lzcm5.*dQ1.*dQ5.*m5.*t3.*t8.*t10.*2.0+Lx3.*Lzcm6.*dQ1.*dQ5.*m6.*t2.*t7.*t10.*2.0+Lx3.*Lzcm6.*dQ1.*dQ5.*m6.*t3.*t8.*t10.*2.0-Lxcm6.*Lz5.*dQ1.*dQ2.*m6.*t5.*t9.*t11.*2.0-Lxcm6.*Lz5.*dQ1.*dQ3.*m6.*t5.*t9.*t11.*2.0+Lxcm6.*Lz5.*dQ4.*dQ5.*m6.*t6.*t7.*t8.*2.0-Lxcm6.*Lz5.*dQ1.*dQ6.*m6.*t5.*t10.*t11.*2.0+Lx2.*Lzcm5.*dQ1.*dQ2.*m5.*t3.*t5.*t32.*4.0+Lx2.*Lzcm5.*dQ1.*dQ3.*m5.*t3.*t5.*t32.*2.0+Lx2.*Lzcm6.*dQ1.*dQ2.*m6.*t3.*t5.*t32.*4.0;
et107 = Lx2.*Lzcm6.*dQ1.*dQ3.*m6.*t3.*t5.*t32.*2.0-Lxcm5.*Lz4.*dQ1.*dQ2.*m5.*t4.*t5.*t32.*4.0-Lxcm5.*Lz4.*dQ1.*dQ2.*m5.*t4.*t5.*t33.*4.0-Lxcm5.*Lz4.*dQ1.*dQ3.*m5.*t4.*t5.*t32.*4.0-Lx3.*Lzcm5.*dQ1.*dQ5.*m5.*t4.*t5.*t32.*2.0-Lxcm5.*Lz4.*dQ1.*dQ3.*m5.*t4.*t5.*t33.*4.0-Lx3.*Lzcm5.*dQ1.*dQ5.*m5.*t4.*t5.*t33.*2.0-Lx3.*Lzcm6.*dQ1.*dQ5.*m6.*t4.*t5.*t32.*2.0+Lxcm6.*Lz5.*dQ1.*dQ2.*m6.*t4.*t6.*t32.*4.0-Lx3.*Lzcm6.*dQ1.*dQ5.*m6.*t4.*t5.*t33.*2.0+Lxcm6.*Lz5.*dQ1.*dQ2.*m6.*t4.*t6.*t33.*4.0+Lxcm6.*Lz5.*dQ1.*dQ3.*m6.*t4.*t6.*t32.*4.0+Lxcm6.*Lz5.*dQ1.*dQ3.*m6.*t4.*t6.*t33.*4.0-Lxcm6.*Lz4.*dQ1.*dQ5.*m6.*t5.*t6.*t32.*2.0+Lxcm6.*Lz5.*dQ1.*dQ2.*m6.*t4.*t6.*t35.*4.0-Lxcm6.*Lz4.*dQ1.*dQ5.*m6.*t5.*t6.*t33.*2.0+Lxcm6.*Lz5.*dQ1.*dQ3.*m6.*t4.*t6.*t35.*4.0-Lx2.*Lzcm5.*dQ1.*dQ5.*m5.*t8.*t10.*t32.*2.0;
et108 = Lx3.*Lzcm5.*dQ1.*dQ4.*m5.*t9.*t10.*t32.*2.0-Lx2.*Lzcm6.*dQ1.*dQ5.*m6.*t8.*t10.*t32.*2.0+Lx3.*Lzcm5.*dQ1.*dQ4.*m5.*t9.*t10.*t33.*2.0+Lx3.*Lzcm6.*dQ1.*dQ4.*m6.*t9.*t10.*t32.*2.0+Lxcm6.*Lz4.*dQ1.*dQ2.*m6.*t9.*t11.*t32.*4.0+Lx3.*Lzcm6.*dQ1.*dQ4.*m6.*t9.*t10.*t33.*2.0+Lxcm6.*Lz4.*dQ1.*dQ2.*m6.*t9.*t11.*t33.*4.0+Lxcm6.*Lz4.*dQ1.*dQ3.*m6.*t9.*t11.*t32.*4.0+Lxcm6.*Lz4.*dQ1.*dQ3.*m6.*t9.*t11.*t33.*4.0-Lxcm6.*Lz5.*dQ1.*dQ4.*m6.*t10.*t11.*t32.*2.0+Lxcm6.*Lz4.*dQ1.*dQ6.*m6.*t10.*t11.*t32.*2.0-Lxcm6.*Lz5.*dQ1.*dQ4.*m6.*t10.*t11.*t33.*2.0+Lxcm6.*Lz4.*dQ1.*dQ6.*m6.*t10.*t11.*t33.*2.0+Lx3.*Lzcm5.*dQ1.*dQ2.*m5.*t5.*t32.*t33.*8.0+Lx3.*Lzcm5.*dQ1.*dQ3.*m5.*t5.*t32.*t33.*8.0+Lx3.*Lzcm6.*dQ1.*dQ2.*m6.*t5.*t32.*t33.*8.0+Lx3.*Lzcm6.*dQ1.*dQ3.*m6.*t5.*t32.*t33.*8.0+Lxcm5.*Lz4.*dQ1.*dQ5.*m5.*t5.*t32.*t33.*4.0-Lxcm6.*Lz5.*dQ1.*dQ5.*m6.*t6.*t32.*t33.*4.0;
et109 = Lxcm6.*Lz5.*dQ1.*dQ5.*m6.*t6.*t32.*t34.*2.0-Lxcm6.*Lz5.*dQ1.*dQ5.*m6.*t6.*t32.*t35.*4.0+Lxcm6.*Lz5.*dQ1.*dQ5.*m6.*t6.*t33.*t34.*2.0-Lxcm6.*Lz5.*dQ1.*dQ5.*m6.*t6.*t33.*t35.*4.0+Lxcm4.*Lzcm4.*dQ1.*dQ4.*m4.*t2.*t7.*t9.*2.0+Lxcm4.*Lzcm4.*dQ2.*dQ3.*m4.*t2.*t8.*t9.*2.0+Lxcm4.*Lzcm4.*dQ2.*dQ3.*m4.*t3.*t7.*t9.*2.0+Lxcm4.*Lzcm4.*dQ1.*dQ4.*m4.*t3.*t8.*t9.*2.0-Lxcm5.*Lzcm5.*dQ1.*dQ4.*m5.*t2.*t7.*t9.*2.0-Lxcm6.*Lzcm6.*dQ4.*dQ5.*m6.*t2.*t3.*t6.*2.0-Lxcm5.*Lzcm5.*dQ2.*dQ3.*m5.*t2.*t8.*t9.*2.0-Lxcm5.*Lzcm5.*dQ2.*dQ3.*m5.*t3.*t7.*t9.*2.0-Lxcm5.*Lzcm5.*dQ1.*dQ4.*m5.*t3.*t8.*t9.*2.0-Lxcm6.*Lzcm6.*dQ1.*dQ2.*m6.*t5.*t9.*t11.*2.0-Lxcm6.*Lzcm6.*dQ1.*dQ3.*m6.*t5.*t9.*t11.*2.0+Lxcm6.*Lzcm6.*dQ4.*dQ5.*m6.*t6.*t7.*t8.*2.0-Lxcm6.*Lzcm6.*dQ1.*dQ6.*m6.*t5.*t10.*t11.*2.0+Lxcm6.*Lzcm6.*dQ1.*dQ2.*m6.*t4.*t6.*t32.*4.0+Lxcm5.*Lzcm5.*dQ4.*dQ5.*m5.*t2.*t3.*t35.*4.0;
et110 = Lxcm6.*Lzcm6.*dQ1.*dQ2.*m6.*t4.*t6.*t33.*4.0+Lxcm6.*Lzcm6.*dQ1.*dQ3.*m6.*t4.*t6.*t32.*4.0+Lxcm6.*Lzcm6.*dQ1.*dQ3.*m6.*t4.*t6.*t33.*4.0+Lxcm6.*Lzcm6.*dQ1.*dQ2.*m6.*t4.*t6.*t35.*4.0+Lxcm6.*Lzcm6.*dQ1.*dQ3.*m6.*t4.*t6.*t35.*4.0-Lxcm5.*Lzcm5.*dQ4.*dQ5.*m5.*t7.*t8.*t35.*4.0-Lxcm6.*Lzcm6.*dQ1.*dQ4.*m6.*t10.*t11.*t32.*2.0-Lxcm6.*Lzcm6.*dQ1.*dQ4.*m6.*t10.*t11.*t33.*2.0+Lxcm4.*Lzcm4.*dQ1.*dQ2.*m4.*t4.*t32.*t33.*8.0+Lxcm4.*Lzcm4.*dQ1.*dQ3.*m4.*t4.*t32.*t33.*8.0-Lxcm5.*Lzcm5.*dQ1.*dQ2.*m5.*t4.*t32.*t33.*8.0-Lxcm5.*Lzcm5.*dQ1.*dQ3.*m5.*t4.*t32.*t33.*8.0-Lxcm5.*Lzcm5.*dQ1.*dQ2.*m5.*t4.*t32.*t35.*8.0-Lxcm5.*Lzcm5.*dQ1.*dQ2.*m5.*t4.*t33.*t35.*8.0-Lxcm5.*Lzcm5.*dQ1.*dQ3.*m5.*t4.*t32.*t35.*8.0-Lxcm5.*Lzcm5.*dQ1.*dQ3.*m5.*t4.*t33.*t35.*8.0-Lxcm6.*Lzcm6.*dQ1.*dQ5.*m6.*t6.*t32.*t33.*4.0+Lxcm6.*Lzcm6.*dQ1.*dQ5.*m6.*t6.*t32.*t34.*2.0;
et111 = Lxcm6.*Lzcm6.*dQ1.*dQ5.*m6.*t6.*t32.*t35.*-4.0+Lxcm6.*Lzcm6.*dQ1.*dQ5.*m6.*t6.*t33.*t34.*2.0-Lxcm6.*Lzcm6.*dQ1.*dQ5.*m6.*t6.*t33.*t35.*4.0-Lxcm5.*Lzcm5.*dQ1.*dQ5.*m5.*t32.*t33.*t34.*4.0+Lxcm5.*Lzcm5.*dQ1.*dQ5.*m5.*t32.*t33.*t35.*8.0-Lxcm5.*Lzcm5.*dQ1.*dQ5.*m5.*t32.*t34.*t35.*4.0-Lxcm5.*Lzcm5.*dQ1.*dQ5.*m5.*t33.*t34.*t35.*4.0+Lycm5.*Lz4.*dQ1.*dQ4.*m5.*t2.*t4.*t7.*2.0+Lycm5.*Lz4.*dQ2.*dQ3.*m5.*t2.*t4.*t8.*2.0+Lycm5.*Lz4.*dQ2.*dQ3.*m5.*t3.*t4.*t7.*2.0+Lycm5.*Lz4.*dQ1.*dQ4.*m5.*t3.*t4.*t8.*2.0-Lycm6.*Lz4.*dQ1.*dQ2.*m6.*t4.*t5.*t11.*2.0-Lycm6.*Lz4.*dQ1.*dQ3.*m6.*t4.*t5.*t11.*2.0-Lycm6.*Lz5.*dQ1.*dQ2.*m6.*t5.*t6.*t9.*2.0-Lycm6.*Lz5.*dQ1.*dQ3.*m6.*t5.*t6.*t9.*2.0+Lycm6.*Lz5.*dQ4.*dQ5.*m6.*t2.*t3.*t11.*2.0-Lycm6.*Lz5.*dQ1.*dQ6.*m6.*t5.*t6.*t10.*2.0-Lycm6.*Lz5.*dQ4.*dQ5.*m6.*t7.*t8.*t11.*2.0;
et112 = Lycm6.*Lz4.*dQ1.*dQ2.*m6.*t6.*t9.*t32.*4.0+Lycm6.*Lz4.*dQ1.*dQ2.*m6.*t6.*t9.*t33.*4.0+Lycm6.*Lz4.*dQ1.*dQ3.*m6.*t6.*t9.*t32.*4.0-Lycm6.*Lz5.*dQ1.*dQ2.*m6.*t4.*t11.*t32.*4.0+Lycm6.*Lz4.*dQ1.*dQ3.*m6.*t6.*t9.*t33.*4.0-Lycm6.*Lz5.*dQ1.*dQ2.*m6.*t4.*t11.*t33.*4.0-Lycm6.*Lz5.*dQ1.*dQ3.*m6.*t4.*t11.*t32.*4.0-Lycm6.*Lz5.*dQ1.*dQ3.*m6.*t4.*t11.*t33.*4.0+Lycm6.*Lz4.*dQ1.*dQ5.*m6.*t5.*t11.*t32.*2.0-Lycm6.*Lz5.*dQ1.*dQ2.*m6.*t4.*t11.*t35.*4.0-Lycm6.*Lz5.*dQ1.*dQ4.*m6.*t6.*t10.*t32.*2.0+Lycm6.*Lz4.*dQ1.*dQ5.*m6.*t5.*t11.*t33.*2.0+Lycm6.*Lz4.*dQ1.*dQ6.*m6.*t6.*t10.*t32.*2.0-Lycm6.*Lz5.*dQ1.*dQ3.*m6.*t4.*t11.*t35.*4.0-Lycm6.*Lz5.*dQ1.*dQ4.*m6.*t6.*t10.*t33.*2.0+Lycm6.*Lz4.*dQ1.*dQ6.*m6.*t6.*t10.*t33.*2.0-Lycm5.*Lz4.*dQ1.*dQ2.*m5.*t9.*t32.*t33.*8.0-Lycm5.*Lz4.*dQ1.*dQ3.*m5.*t9.*t32.*t33.*8.0;
et113 = Lycm6.*Lz5.*dQ1.*dQ5.*m6.*t11.*t32.*t33.*4.0-Lycm6.*Lz5.*dQ1.*dQ5.*m6.*t11.*t32.*t34.*2.0+Lycm6.*Lz5.*dQ1.*dQ5.*m6.*t11.*t32.*t35.*4.0-Lycm6.*Lz5.*dQ1.*dQ5.*m6.*t11.*t33.*t34.*2.0+Lycm6.*Lz5.*dQ1.*dQ5.*m6.*t11.*t33.*t35.*4.0+Lycm4.*Lzcm4.*dQ1.*dQ4.*m4.*t2.*t4.*t7.*2.0+Lycm4.*Lzcm4.*dQ2.*dQ3.*m4.*t2.*t4.*t8.*2.0+Lycm4.*Lzcm4.*dQ2.*dQ3.*m4.*t3.*t4.*t7.*2.0+Lycm4.*Lzcm4.*dQ1.*dQ4.*m4.*t3.*t4.*t8.*2.0-Lycm5.*Lzcm5.*dQ2.*dQ3.*m5.*t2.*t3.*t10.*2.0-Lycm6.*Lzcm6.*dQ1.*dQ2.*m6.*t5.*t6.*t9.*2.0-Lycm6.*Lzcm6.*dQ1.*dQ3.*m6.*t5.*t6.*t9.*2.0+Lycm6.*Lzcm6.*dQ4.*dQ5.*m6.*t2.*t3.*t11.*2.0+Lycm5.*Lzcm5.*dQ2.*dQ3.*m5.*t7.*t8.*t10.*2.0-Lycm6.*Lzcm6.*dQ1.*dQ6.*m6.*t5.*t6.*t10.*2.0-Lycm6.*Lzcm6.*dQ4.*dQ5.*m6.*t7.*t8.*t11.*2.0+Lycm5.*Lzcm5.*dQ1.*dQ2.*m5.*t5.*t9.*t32.*4.0+Lycm5.*Lzcm5.*dQ1.*dQ2.*m5.*t5.*t9.*t33.*4.0+Lycm5.*Lzcm5.*dQ1.*dQ3.*m5.*t5.*t9.*t32.*4.0;
et114 = Lycm5.*Lzcm5.*dQ1.*dQ3.*m5.*t5.*t9.*t33.*4.0-Lycm6.*Lzcm6.*dQ1.*dQ2.*m6.*t4.*t11.*t32.*4.0-Lycm6.*Lzcm6.*dQ1.*dQ2.*m6.*t4.*t11.*t33.*4.0-Lycm6.*Lzcm6.*dQ1.*dQ3.*m6.*t4.*t11.*t32.*4.0-Lycm6.*Lzcm6.*dQ1.*dQ3.*m6.*t4.*t11.*t33.*4.0-Lycm6.*Lzcm6.*dQ1.*dQ2.*m6.*t4.*t11.*t35.*4.0-Lycm6.*Lzcm6.*dQ1.*dQ4.*m6.*t6.*t10.*t32.*2.0-Lycm6.*Lzcm6.*dQ1.*dQ3.*m6.*t4.*t11.*t35.*4.0-Lycm6.*Lzcm6.*dQ1.*dQ4.*m6.*t6.*t10.*t33.*2.0-Lycm4.*Lzcm4.*dQ1.*dQ2.*m4.*t9.*t32.*t33.*8.0-Lycm4.*Lzcm4.*dQ1.*dQ3.*m4.*t9.*t32.*t33.*8.0+Lycm5.*Lzcm5.*dQ1.*dQ4.*m5.*t10.*t32.*t33.*4.0+Lycm5.*Lzcm5.*dQ1.*dQ4.*m5.*t10.*t32.*t34.*4.0+Lycm5.*Lzcm5.*dQ1.*dQ4.*m5.*t10.*t33.*t34.*4.0+Lycm6.*Lzcm6.*dQ1.*dQ5.*m6.*t11.*t32.*t33.*4.0-Lycm6.*Lzcm6.*dQ1.*dQ5.*m6.*t11.*t32.*t34.*2.0+Lycm6.*Lzcm6.*dQ1.*dQ5.*m6.*t11.*t32.*t35.*4.0-Lycm6.*Lzcm6.*dQ1.*dQ5.*m6.*t11.*t33.*t34.*2.0;
et115 = Lycm6.*Lzcm6.*dQ1.*dQ5.*m6.*t11.*t33.*t35.*4.0-Lz4.*Lz5.*dQ1.*dQ2.*m6.*t2.*t5.*t7.*4.0-Lz4.*Lz5.*dQ1.*dQ3.*m6.*t2.*t5.*t7.*4.0-Lz4.*Lz5.*dQ1.*dQ2.*m6.*t3.*t5.*t8.*4.0-Lz4.*Lz5.*dQ1.*dQ3.*m6.*t3.*t5.*t8.*4.0-Lz4.*Lz5.*dQ1.*dQ2.*m6.*t4.*t10.*t32.*4.0-Lz4.*Lz5.*dQ1.*dQ2.*m6.*t4.*t10.*t33.*4.0-Lz4.*Lz5.*dQ1.*dQ3.*m6.*t4.*t10.*t32.*4.0-Lz4.*Lz5.*dQ1.*dQ3.*m6.*t4.*t10.*t33.*4.0+Lz4.*Lz5.*dQ1.*dQ5.*m6.*t10.*t32.*t33.*4.0-Lz4.*Lzcm5.*dQ1.*dQ2.*m5.*t2.*t5.*t7.*4.0-Lz4.*Lzcm5.*dQ1.*dQ3.*m5.*t2.*t5.*t7.*4.0-Lz4.*Lzcm5.*dQ1.*dQ2.*m5.*t3.*t5.*t8.*4.0-Lz4.*Lzcm6.*dQ1.*dQ2.*m6.*t2.*t5.*t7.*4.0-Lz4.*Lzcm5.*dQ1.*dQ3.*m5.*t3.*t5.*t8.*4.0-Lz4.*Lzcm6.*dQ1.*dQ3.*m6.*t2.*t5.*t7.*4.0-Lz4.*Lzcm6.*dQ1.*dQ2.*m6.*t3.*t5.*t8.*4.0-Lz4.*Lzcm6.*dQ1.*dQ3.*m6.*t3.*t5.*t8.*4.0;
et116 = Lz5.*Lzcm6.*dQ1.*dQ5.*m6.*t2.*t4.*t7.*4.0+Lz5.*Lzcm6.*dQ1.*dQ5.*m6.*t3.*t4.*t8.*4.0+Lz5.*Lzcm6.*dQ2.*dQ5.*m6.*t2.*t3.*t9.*4.0+Lz5.*Lzcm6.*dQ1.*dQ2.*m6.*t4.*t5.*t10.*4.0+Lz5.*Lzcm6.*dQ3.*dQ5.*m6.*t2.*t3.*t9.*4.0+Lz5.*Lzcm6.*dQ1.*dQ3.*m6.*t4.*t5.*t10.*4.0-Lz5.*Lzcm6.*dQ2.*dQ5.*m6.*t7.*t8.*t9.*4.0-Lz5.*Lzcm6.*dQ3.*dQ5.*m6.*t7.*t8.*t9.*4.0-Lz4.*Lzcm5.*dQ1.*dQ2.*m5.*t4.*t10.*t32.*4.0+Lz5.*Lzcm6.*dQ1.*dQ2.*m6.*t2.*t7.*t34.*4.0-Lz4.*Lzcm5.*dQ1.*dQ2.*m5.*t4.*t10.*t33.*4.0-Lz4.*Lzcm5.*dQ1.*dQ3.*m5.*t4.*t10.*t32.*4.0-Lz5.*Lzcm6.*dQ1.*dQ2.*m6.*t2.*t7.*t35.*4.0+Lz5.*Lzcm6.*dQ1.*dQ3.*m6.*t2.*t7.*t34.*4.0-Lz4.*Lzcm5.*dQ1.*dQ3.*m5.*t4.*t10.*t33.*4.0-Lz4.*Lzcm6.*dQ1.*dQ2.*m6.*t4.*t10.*t32.*4.0+Lz5.*Lzcm6.*dQ1.*dQ2.*m6.*t3.*t8.*t34.*4.0-Lz5.*Lzcm6.*dQ1.*dQ3.*m6.*t2.*t7.*t35.*4.0-Lz4.*Lzcm6.*dQ1.*dQ2.*m6.*t4.*t10.*t33.*4.0;
et117 = Lz4.*Lzcm6.*dQ1.*dQ3.*m6.*t4.*t10.*t32.*-4.0-Lz5.*Lzcm6.*dQ1.*dQ2.*m6.*t3.*t8.*t35.*4.0+Lz5.*Lzcm6.*dQ1.*dQ3.*m6.*t3.*t8.*t34.*4.0-Lz4.*Lzcm6.*dQ1.*dQ3.*m6.*t4.*t10.*t33.*4.0-Lz5.*Lzcm6.*dQ1.*dQ3.*m6.*t3.*t8.*t35.*4.0+Lz5.*Lzcm6.*dQ1.*dQ4.*m6.*t4.*t9.*t32.*4.0+Lz5.*Lzcm6.*dQ2.*dQ4.*m6.*t2.*t8.*t34.*4.0+Lz5.*Lzcm6.*dQ2.*dQ4.*m6.*t3.*t7.*t34.*4.0+Lz5.*Lzcm6.*dQ1.*dQ4.*m6.*t4.*t9.*t33.*4.0+Lz5.*Lzcm6.*dQ2.*dQ4.*m6.*t2.*t8.*t35.*4.0+Lz5.*Lzcm6.*dQ2.*dQ4.*m6.*t3.*t7.*t35.*4.0+Lz5.*Lzcm6.*dQ3.*dQ4.*m6.*t2.*t8.*t34.*4.0+Lz5.*Lzcm6.*dQ3.*dQ4.*m6.*t3.*t7.*t34.*4.0+Lz5.*Lzcm6.*dQ3.*dQ4.*m6.*t2.*t8.*t35.*4.0+Lz5.*Lzcm6.*dQ3.*dQ4.*m6.*t3.*t7.*t35.*4.0-Lz5.*Lzcm6.*dQ1.*dQ5.*m6.*t5.*t10.*t32.*4.0-Lz5.*Lzcm6.*dQ1.*dQ5.*m6.*t5.*t10.*t33.*4.0+Lz4.*Lzcm5.*dQ1.*dQ5.*m5.*t10.*t32.*t33.*4.0+Lz4.*Lzcm6.*dQ1.*dQ5.*m6.*t10.*t32.*t33.*4.0;
et118 = Ixx6.*dQ2.*dQ3.*t2.*t3.*t5.*t6.*t11.*2.0+Ixx5.*dQ1.*dQ4.*t2.*t5.*t7.*t9.*t10.*2.0+Ixx5.*dQ2.*dQ3.*t2.*t5.*t8.*t9.*t10.*2.0+Ixx5.*dQ2.*dQ3.*t3.*t5.*t7.*t9.*t10.*2.0+Ixx5.*dQ1.*dQ4.*t3.*t5.*t8.*t9.*t10.*2.0-Ixx6.*dQ2.*dQ3.*t5.*t6.*t7.*t8.*t11.*2.0+Ixx6.*dQ5.*dQ6.*t2.*t6.*t8.*t9.*t11.*2.0+Ixx6.*dQ5.*dQ6.*t3.*t6.*t7.*t9.*t11.*2.0-Ixx5.*dQ2.*dQ3.*t2.*t3.*t4.*t9.*t35.*2.0-Ixx6.*dQ2.*dQ3.*t2.*t3.*t4.*t9.*t36.*2.0-Ixx6.*dQ2.*dQ6.*t2.*t3.*t4.*t10.*t36.*2.0-Ixx6.*dQ3.*dQ6.*t2.*t3.*t4.*t10.*t36.*2.0+Ixx6.*dQ4.*dQ5.*t2.*t3.*t5.*t10.*t36.*2.0-Ixx6.*dQ5.*dQ6.*t2.*t4.*t5.*t8.*t36.*2.0-Ixx6.*dQ5.*dQ6.*t3.*t4.*t5.*t7.*t36.*2.0+Ixx5.*dQ2.*dQ3.*t4.*t7.*t8.*t9.*t35.*2.0+Ixx6.*dQ4.*dQ6.*t2.*t3.*t6.*t11.*t35.*2.0+Ixx6.*dQ1.*dQ6.*t2.*t7.*t9.*t10.*t33.*4.0+Ixx6.*dQ1.*dQ6.*t3.*t8.*t9.*t10.*t32.*4.0;
et119 = Ixx6.*dQ2.*dQ3.*t4.*t7.*t8.*t9.*t36.*2.0+Ixx6.*dQ1.*dQ2.*t6.*t9.*t10.*t11.*t32.*4.0+Ixx6.*dQ1.*dQ6.*t2.*t7.*t9.*t10.*t36.*4.0+Ixx6.*dQ1.*dQ2.*t6.*t9.*t10.*t11.*t33.*4.0+Ixx6.*dQ1.*dQ3.*t6.*t9.*t10.*t11.*t32.*4.0+Ixx6.*dQ1.*dQ3.*t6.*t9.*t10.*t11.*t33.*4.0+Ixx6.*dQ1.*dQ6.*t3.*t8.*t9.*t10.*t36.*4.0+Ixx6.*dQ2.*dQ6.*t4.*t7.*t8.*t10.*t36.*2.0+Ixx6.*dQ3.*dQ6.*t4.*t7.*t8.*t10.*t36.*2.0-Ixx6.*dQ4.*dQ5.*t5.*t7.*t8.*t10.*t36.*2.0-Ixx6.*dQ4.*dQ6.*t2.*t8.*t9.*t10.*t36.*2.0-Ixx6.*dQ4.*dQ6.*t3.*t7.*t9.*t10.*t36.*2.0-Ixx6.*dQ4.*dQ6.*t6.*t7.*t8.*t11.*t35.*2.0+Ixx5.*dQ1.*dQ2.*t4.*t5.*t10.*t32.*t33.*8.0+Ixx5.*dQ1.*dQ5.*t2.*t4.*t7.*t33.*t35.*8.0+Ixx5.*dQ1.*dQ3.*t4.*t5.*t10.*t32.*t33.*8.0+Ixx5.*dQ1.*dQ5.*t3.*t4.*t8.*t32.*t35.*8.0-Ixx6.*dQ1.*dQ5.*t2.*t4.*t7.*t33.*t36.*4.0-Ixx6.*dQ1.*dQ5.*t3.*t4.*t8.*t32.*t36.*4.0;
et120 = Ixx6.*dQ1.*dQ2.*t4.*t5.*t10.*t32.*t36.*-4.0-Ixx6.*dQ1.*dQ5.*t2.*t4.*t7.*t35.*t36.*4.0-Ixx6.*dQ1.*dQ6.*t4.*t5.*t9.*t32.*t33.*4.0-Ixx6.*dQ1.*dQ2.*t4.*t5.*t10.*t33.*t36.*4.0-Ixx6.*dQ1.*dQ3.*t4.*t5.*t10.*t32.*t36.*4.0-Ixx6.*dQ1.*dQ3.*t4.*t5.*t10.*t33.*t36.*4.0-Ixx6.*dQ1.*dQ4.*t5.*t6.*t11.*t32.*t33.*4.0-Ixx6.*dQ1.*dQ5.*t3.*t4.*t8.*t35.*t36.*4.0-Ixx6.*dQ2.*dQ5.*t2.*t3.*t9.*t35.*t36.*2.0-Ixx6.*dQ1.*dQ4.*t5.*t6.*t11.*t32.*t34.*4.0-Ixx6.*dQ1.*dQ6.*t4.*t5.*t9.*t32.*t36.*4.0-Ixx6.*dQ2.*dQ6.*t2.*t5.*t8.*t34.*t36.*4.0-Ixx6.*dQ2.*dQ6.*t3.*t5.*t7.*t34.*t36.*4.0-Ixx6.*dQ3.*dQ5.*t2.*t3.*t9.*t35.*t36.*2.0-Ixx6.*dQ1.*dQ4.*t5.*t6.*t11.*t33.*t34.*4.0-Ixx6.*dQ1.*dQ6.*t4.*t5.*t9.*t33.*t36.*4.0-Ixx6.*dQ3.*dQ6.*t2.*t5.*t8.*t34.*t36.*4.0-Ixx6.*dQ3.*dQ6.*t3.*t5.*t7.*t34.*t36.*4.0;
et121 = Ixx6.*dQ4.*dQ5.*t2.*t4.*t8.*t35.*t36.*2.0+Ixx6.*dQ4.*dQ5.*t3.*t4.*t7.*t35.*t36.*2.0+Ixx6.*dQ2.*dQ5.*t7.*t8.*t9.*t35.*t36.*2.0+Ixx6.*dQ3.*dQ5.*t7.*t8.*t9.*t35.*t36.*2.0+Ixx5.*dQ1.*dQ2.*t2.*t7.*t33.*t34.*t35.*4.0+Ixx5.*dQ1.*dQ2.*t3.*t8.*t32.*t34.*t35.*4.0+Ixx5.*dQ1.*dQ3.*t2.*t7.*t33.*t34.*t35.*4.0+Ixx5.*dQ1.*dQ3.*t3.*t8.*t32.*t34.*t35.*4.0+Ixx6.*dQ1.*dQ2.*t2.*t7.*t33.*t34.*t36.*4.0+Ixx6.*dQ1.*dQ2.*t2.*t7.*t33.*t35.*t36.*4.0+Ixx6.*dQ1.*dQ2.*t3.*t8.*t32.*t34.*t36.*4.0+Ixx6.*dQ1.*dQ3.*t2.*t7.*t33.*t34.*t36.*4.0+Ixx5.*dQ1.*dQ4.*t4.*t9.*t32.*t33.*t35.*4.0-Ixx6.*dQ1.*dQ2.*t2.*t7.*t34.*t35.*t36.*2.0+Ixx6.*dQ1.*dQ2.*t3.*t8.*t32.*t35.*t36.*4.0+Ixx6.*dQ1.*dQ3.*t2.*t7.*t33.*t35.*t36.*4.0+Ixx6.*dQ1.*dQ3.*t3.*t8.*t32.*t34.*t36.*4.0-Ixx6.*dQ1.*dQ3.*t2.*t7.*t34.*t35.*t36.*2.0+Ixx6.*dQ1.*dQ3.*t3.*t8.*t32.*t35.*t36.*4.0;
et122 = Ixx5.*dQ1.*dQ5.*t5.*t10.*t32.*t33.*t34.*4.0-Ixx6.*dQ1.*dQ2.*t3.*t8.*t34.*t35.*t36.*2.0+Ixx6.*dQ1.*dQ4.*t4.*t9.*t32.*t33.*t36.*4.0-Ixx6.*dQ1.*dQ3.*t3.*t8.*t34.*t35.*t36.*2.0-Ixx6.*dQ1.*dQ4.*t4.*t9.*t32.*t35.*t36.*2.0-Ixx6.*dQ2.*dQ4.*t2.*t8.*t34.*t35.*t36.*2.0-Ixx6.*dQ2.*dQ4.*t3.*t7.*t34.*t35.*t36.*2.0-Ixx6.*dQ1.*dQ4.*t4.*t9.*t33.*t35.*t36.*2.0+Ixx6.*dQ1.*dQ5.*t5.*t10.*t32.*t33.*t36.*4.0-Ixx6.*dQ3.*dQ4.*t2.*t8.*t34.*t35.*t36.*2.0-Ixx6.*dQ3.*dQ4.*t3.*t7.*t34.*t35.*t36.*2.0-Ixx6.*dQ1.*dQ5.*t5.*t10.*t32.*t34.*t36.*2.0+Ixx6.*dQ1.*dQ6.*t6.*t11.*t32.*t33.*t34.*4.0-Ixx6.*dQ1.*dQ5.*t5.*t10.*t33.*t34.*t36.*2.0+Ixx6.*dQ1.*dQ6.*t6.*t11.*t32.*t33.*t35.*4.0-Ixx6.*dQ1.*dQ6.*t6.*t11.*t32.*t34.*t35.*2.0-Ixx6.*dQ1.*dQ6.*t6.*t11.*t33.*t34.*t35.*2.0-Ixy5.*dQ1.*dQ2.*t2.*t4.*t5.*t7.*t9.*2.0;
et123 = Ixy5.*dQ1.*dQ4.*t2.*t3.*t5.*t7.*t8.*-2.0-Ixy5.*dQ1.*dQ3.*t2.*t4.*t5.*t7.*t9.*2.0+Ixy6.*dQ1.*dQ2.*t2.*t4.*t5.*t7.*t9.*2.0+Ixy6.*dQ1.*dQ4.*t2.*t3.*t5.*t7.*t8.*2.0-Ixy5.*dQ1.*dQ2.*t3.*t4.*t5.*t8.*t9.*2.0+Ixy6.*dQ1.*dQ3.*t2.*t4.*t5.*t7.*t9.*2.0-Ixy5.*dQ1.*dQ3.*t3.*t4.*t5.*t8.*t9.*2.0+Ixy6.*dQ1.*dQ2.*t3.*t4.*t5.*t8.*t9.*2.0+Ixy6.*dQ1.*dQ3.*t3.*t4.*t5.*t8.*t9.*2.0+Ixy6.*dQ1.*dQ6.*t2.*t4.*t5.*t7.*t10.*2.0+Ixy6.*dQ1.*dQ5.*t2.*t4.*t6.*t7.*t11.*2.0+Ixy6.*dQ1.*dQ6.*t3.*t4.*t5.*t8.*t10.*2.0+Ixy6.*dQ2.*dQ6.*t2.*t3.*t5.*t9.*t10+Ixy6.*dQ1.*dQ5.*t3.*t4.*t6.*t8.*t11.*2.0+Ixy6.*dQ3.*dQ6.*t2.*t3.*t5.*t9.*t10+Ixy6.*dQ1.*dQ2.*t4.*t5.*t6.*t10.*t11.*2.0-Ixy6.*dQ4.*dQ6.*t2.*t4.*t5.*t8.*t10-Ixy6.*dQ4.*dQ6.*t3.*t4.*t5.*t7.*t10+Ixy6.*dQ1.*dQ3.*t4.*t5.*t6.*t10.*t11.*2.0;
et124 = Ixy6.*dQ2.*dQ6.*t2.*t5.*t6.*t8.*t11.*2.0+Ixy6.*dQ2.*dQ6.*t3.*t5.*t6.*t7.*t11.*2.0-Ixy6.*dQ4.*dQ5.*t2.*t4.*t6.*t8.*t11.*2.0-Ixy6.*dQ4.*dQ5.*t3.*t4.*t6.*t7.*t11.*2.0+Ixy6.*dQ3.*dQ6.*t2.*t5.*t6.*t8.*t11.*2.0+Ixy6.*dQ3.*dQ6.*t3.*t5.*t6.*t7.*t11.*2.0-Ixy6.*dQ5.*dQ6.*t2.*t3.*t6.*t10.*t11.*2.0-Ixy6.*dQ2.*dQ6.*t5.*t7.*t8.*t9.*t10-Ixy6.*dQ3.*dQ6.*t5.*t7.*t8.*t9.*t10+Ixy6.*dQ5.*dQ6.*t6.*t7.*t8.*t10.*t11.*2.0+Ixy4.*dQ1.*dQ2.*t2.*t4.*t7.*t9.*t33.*4.0+Ixy4.*dQ1.*dQ2.*t3.*t4.*t8.*t9.*t32.*4.0+Ixy4.*dQ1.*dQ3.*t2.*t4.*t7.*t9.*t33.*4.0+Ixy4.*dQ1.*dQ4.*t2.*t3.*t7.*t8.*t34.*4.0+Ixy6.*dQ2.*dQ5.*t2.*t3.*t4.*t5.*t36.*2.0+Ixy4.*dQ1.*dQ3.*t3.*t4.*t8.*t9.*t32.*4.0+Ixy6.*dQ3.*dQ5.*t2.*t3.*t4.*t5.*t36.*2.0+Ixy5.*dQ1.*dQ4.*t2.*t4.*t7.*t10.*t33.*2.0+Ixy5.*dQ1.*dQ4.*t3.*t4.*t8.*t10.*t32.*2.0;
et125 = Ixy5.*dQ1.*dQ5.*t2.*t5.*t7.*t9.*t33.*2.0-Ixy6.*dQ1.*dQ4.*t2.*t4.*t7.*t10.*t33.*2.0-Ixy6.*dQ1.*dQ6.*t2.*t3.*t7.*t8.*t34.*2.0+Ixy5.*dQ1.*dQ5.*t3.*t5.*t8.*t9.*t32.*2.0-Ixy6.*dQ1.*dQ2.*t2.*t6.*t7.*t11.*t33.*8.0-Ixy6.*dQ1.*dQ4.*t3.*t4.*t8.*t10.*t32.*2.0-Ixy6.*dQ1.*dQ5.*t2.*t5.*t7.*t9.*t33.*2.0-Ixy6.*dQ1.*dQ6.*t2.*t3.*t7.*t8.*t35.*2.0-Ixy6.*dQ1.*dQ2.*t2.*t6.*t7.*t11.*t34.*2.0-Ixy6.*dQ1.*dQ2.*t3.*t6.*t8.*t11.*t32.*8.0-Ixy6.*dQ1.*dQ3.*t2.*t6.*t7.*t11.*t33.*8.0-Ixy6.*dQ1.*dQ5.*t3.*t5.*t8.*t9.*t32.*2.0-Ixy6.*dQ1.*dQ6.*t2.*t3.*t7.*t8.*t36.*8.0-Ixy6.*dQ1.*dQ2.*t2.*t6.*t7.*t11.*t35.*2.0-Ixy6.*dQ1.*dQ3.*t2.*t6.*t7.*t11.*t34.*2.0-Ixy6.*dQ1.*dQ3.*t3.*t6.*t8.*t11.*t32.*8.0-Ixy6.*dQ1.*dQ4.*t2.*t4.*t7.*t10.*t36.*2.0;
et126 = Ixy6.*dQ1.*dQ2.*t3.*t6.*t8.*t11.*t34.*-2.0-Ixy6.*dQ1.*dQ3.*t2.*t6.*t7.*t11.*t35.*2.0-Ixy6.*dQ1.*dQ5.*t2.*t5.*t7.*t9.*t36.*2.0-Ixy6.*dQ2.*dQ3.*t2.*t4.*t8.*t10.*t36.*2.0-Ixy6.*dQ2.*dQ3.*t3.*t4.*t7.*t10.*t36.*2.0-Ixy6.*dQ1.*dQ2.*t3.*t6.*t8.*t11.*t35.*2.0-Ixy6.*dQ1.*dQ3.*t3.*t6.*t8.*t11.*t34.*2.0-Ixy6.*dQ1.*dQ4.*t3.*t4.*t8.*t10.*t36.*2.0-Ixy6.*dQ1.*dQ3.*t3.*t6.*t8.*t11.*t35.*2.0-Ixy6.*dQ1.*dQ4.*t4.*t6.*t9.*t11.*t32.*2.0-Ixy6.*dQ1.*dQ5.*t3.*t5.*t8.*t9.*t36.*2.0-Ixy6.*dQ2.*dQ4.*t2.*t6.*t8.*t11.*t34.*2.0-Ixy6.*dQ2.*dQ4.*t3.*t6.*t7.*t11.*t34.*2.0-Ixy6.*dQ2.*dQ5.*t4.*t5.*t7.*t8.*t36.*2.0-Ixy6.*dQ2.*dQ6.*t2.*t4.*t8.*t9.*t36.*2.0-Ixy6.*dQ2.*dQ6.*t3.*t4.*t7.*t9.*t36.*2.0-Ixy6.*dQ1.*dQ4.*t4.*t6.*t9.*t11.*t33.*2.0+Ixy6.*dQ2.*dQ4.*t2.*t6.*t8.*t11.*t35.*2.0;
et127 = Ixy6.*dQ2.*dQ4.*t3.*t6.*t7.*t11.*t35.*2.0-Ixy6.*dQ3.*dQ4.*t2.*t6.*t8.*t11.*t34.*2.0-Ixy6.*dQ3.*dQ4.*t3.*t6.*t7.*t11.*t34.*2.0-Ixy6.*dQ3.*dQ5.*t4.*t5.*t7.*t8.*t36.*2.0-Ixy6.*dQ3.*dQ6.*t2.*t4.*t8.*t9.*t36.*2.0-Ixy6.*dQ3.*dQ6.*t3.*t4.*t7.*t9.*t36.*2.0+Ixy6.*dQ3.*dQ4.*t2.*t6.*t8.*t11.*t35.*2.0+Ixy6.*dQ3.*dQ4.*t3.*t6.*t7.*t11.*t35.*2.0-Ixy6.*dQ1.*dQ5.*t5.*t6.*t10.*t11.*t32.*2.0-Ixy6.*dQ1.*dQ5.*t5.*t6.*t10.*t11.*t33.*2.0+Ixy6.*dQ2.*dQ3.*t2.*t3.*t5.*t34.*t36.*4.0+Ixy5.*dQ1.*dQ5.*t4.*t9.*t10.*t32.*t33.*2.0-Ixy6.*dQ1.*dQ5.*t4.*t9.*t10.*t32.*t33.*2.0-Ixy6.*dQ2.*dQ3.*t5.*t7.*t8.*t34.*t36.*4.0-Ixy6.*dQ1.*dQ5.*t4.*t9.*t10.*t32.*t36.*2.0-Ixy6.*dQ2.*dQ5.*t2.*t8.*t10.*t34.*t36.*2.0-Ixy6.*dQ2.*dQ5.*t3.*t7.*t10.*t34.*t36.*2.0-Ixy6.*dQ1.*dQ5.*t4.*t9.*t10.*t33.*t36.*2.0;
et128 = Ixy6.*dQ3.*dQ5.*t2.*t8.*t10.*t34.*t36.*-2.0-Ixy6.*dQ3.*dQ5.*t3.*t7.*t10.*t34.*t36.*2.0+Ixy6.*dQ1.*dQ2.*t9.*t10.*t32.*t33.*t36.*8.0+Ixy6.*dQ1.*dQ3.*t9.*t10.*t32.*t33.*t36.*8.0-Ixy6.*dQ1.*dQ4.*t5.*t32.*t33.*t34.*t36.*8.0-Ixy6.*dQ1.*dQ6.*t32.*t33.*t34.*t35.*t36.*4.0-Ixz4.*dQ1.*dQ2.*t2.*t3.*t4.*t7.*t8.*4.0-Ixz4.*dQ1.*dQ3.*t2.*t3.*t4.*t7.*t8.*4.0+Ixz5.*dQ1.*dQ2.*t2.*t3.*t4.*t7.*t8.*4.0+Ixz5.*dQ1.*dQ3.*t2.*t3.*t4.*t7.*t8.*4.0+Ixz6.*dQ1.*dQ5.*t2.*t3.*t6.*t7.*t8.*2.0+Ixz5.*dQ1.*dQ5.*t2.*t4.*t5.*t7.*t10.*4.0+Ixz6.*dQ1.*dQ2.*t2.*t5.*t6.*t7.*t10.*2.0+Ixz6.*dQ1.*dQ3.*t2.*t5.*t6.*t7.*t10.*2.0+Ixz6.*dQ1.*dQ4.*t2.*t4.*t5.*t7.*t11+Ixz5.*dQ1.*dQ5.*t3.*t4.*t5.*t8.*t10.*4.0+Ixz6.*dQ1.*dQ2.*t3.*t5.*t6.*t8.*t10.*2.0+Ixz6.*dQ2.*dQ3.*t2.*t4.*t5.*t8.*t11+Ixz6.*dQ2.*dQ3.*t3.*t4.*t5.*t7.*t11;
et129 = Ixz6.*dQ1.*dQ3.*t3.*t5.*t6.*t8.*t10.*2.0+Ixz6.*dQ1.*dQ4.*t3.*t4.*t5.*t8.*t11+Ixz6.*dQ1.*dQ6.*t2.*t5.*t6.*t7.*t9-Ixz5.*dQ4.*dQ5.*t2.*t4.*t5.*t8.*t10.*2.0-Ixz5.*dQ4.*dQ5.*t3.*t4.*t5.*t7.*t10.*2.0-Ixz6.*dQ2.*dQ4.*t2.*t5.*t6.*t8.*t10.*2.0-Ixz6.*dQ2.*dQ4.*t3.*t5.*t6.*t7.*t10.*2.0+Ixz6.*dQ2.*dQ5.*t2.*t3.*t4.*t10.*t11+Ixz6.*dQ1.*dQ6.*t3.*t5.*t6.*t8.*t9-Ixz6.*dQ3.*dQ4.*t2.*t5.*t6.*t8.*t10.*2.0-Ixz6.*dQ3.*dQ4.*t3.*t5.*t6.*t7.*t10.*2.0+Ixz6.*dQ3.*dQ5.*t2.*t3.*t4.*t10.*t11-Ixz6.*dQ4.*dQ6.*t2.*t5.*t6.*t8.*t9-Ixz6.*dQ4.*dQ6.*t3.*t5.*t6.*t7.*t9-Ixz6.*dQ4.*dQ6.*t2.*t3.*t5.*t10.*t11-Ixz6.*dQ1.*dQ5.*t2.*t7.*t9.*t10.*t11-Ixz6.*dQ1.*dQ5.*t3.*t8.*t9.*t10.*t11-Ixz6.*dQ2.*dQ5.*t4.*t7.*t8.*t10.*t11-Ixz6.*dQ3.*dQ5.*t4.*t7.*t8.*t10.*t11;
et130 = Ixz6.*dQ4.*dQ6.*t5.*t7.*t8.*t10.*t11-Ixz5.*dQ1.*dQ2.*t2.*t5.*t7.*t10.*t33.*4.0+Ixz5.*dQ1.*dQ5.*t2.*t3.*t7.*t8.*t34.*2.0+Ixz5.*dQ1.*dQ2.*t2.*t5.*t7.*t10.*t34.*2.0-Ixz5.*dQ1.*dQ2.*t3.*t5.*t8.*t10.*t32.*4.0-Ixz5.*dQ1.*dQ3.*t2.*t5.*t7.*t10.*t33.*4.0-Ixz5.*dQ1.*dQ5.*t2.*t3.*t7.*t8.*t35.*4.0+Ixz5.*dQ1.*dQ3.*t2.*t5.*t7.*t10.*t34.*2.0-Ixz5.*dQ1.*dQ3.*t3.*t5.*t8.*t10.*t32.*4.0+Ixz5.*dQ1.*dQ2.*t3.*t5.*t8.*t10.*t34.*2.0+Ixz6.*dQ1.*dQ4.*t2.*t6.*t7.*t9.*t33.*2.0+Ixz5.*dQ1.*dQ3.*t3.*t5.*t8.*t10.*t34.*2.0+Ixz6.*dQ1.*dQ4.*t3.*t6.*t8.*t9.*t32.*2.0+Ixz5.*dQ1.*dQ4.*t4.*t5.*t9.*t10.*t32.*2.0+Ixz5.*dQ2.*dQ4.*t2.*t5.*t8.*t10.*t34.*2.0+Ixz5.*dQ2.*dQ4.*t3.*t5.*t7.*t10.*t34.*2.0+Ixz6.*dQ1.*dQ4.*t2.*t6.*t7.*t9.*t35.*2.0+Ixz6.*dQ1.*dQ6.*t2.*t4.*t7.*t11.*t33.*2.0+Ixz5.*dQ1.*dQ4.*t4.*t5.*t9.*t10.*t33.*2.0;
et131 = Ixz5.*dQ3.*dQ4.*t2.*t5.*t8.*t10.*t34.*2.0+Ixz5.*dQ3.*dQ4.*t3.*t5.*t7.*t10.*t34.*2.0+Ixz6.*dQ1.*dQ6.*t3.*t4.*t8.*t11.*t32.*2.0+Ixz6.*dQ2.*dQ3.*t2.*t3.*t10.*t11.*t34.*2.0+Ixz6.*dQ2.*dQ3.*t2.*t6.*t8.*t9.*t35.*2.0+Ixz6.*dQ2.*dQ3.*t3.*t6.*t7.*t9.*t35.*2.0+Ixz6.*dQ1.*dQ4.*t3.*t6.*t8.*t9.*t35.*2.0+Ixz6.*dQ1.*dQ6.*t2.*t4.*t7.*t11.*t35.*2.0+Ixz6.*dQ1.*dQ5.*t4.*t5.*t9.*t11.*t32+Ixz6.*dQ2.*dQ5.*t2.*t5.*t8.*t11.*t34+Ixz6.*dQ2.*dQ5.*t3.*t5.*t7.*t11.*t34+Ixz6.*dQ1.*dQ5.*t4.*t5.*t9.*t11.*t33+Ixz6.*dQ1.*dQ6.*t3.*t4.*t8.*t11.*t35.*2.0+Ixz6.*dQ1.*dQ6.*t4.*t6.*t9.*t10.*t32+Ixz6.*dQ2.*dQ6.*t2.*t3.*t9.*t11.*t35+Ixz6.*dQ2.*dQ6.*t2.*t6.*t8.*t10.*t34+Ixz6.*dQ2.*dQ6.*t3.*t6.*t7.*t10.*t34+Ixz6.*dQ3.*dQ5.*t2.*t5.*t8.*t11.*t34+Ixz6.*dQ3.*dQ5.*t3.*t5.*t7.*t11.*t34+Ixz6.*dQ1.*dQ6.*t4.*t6.*t9.*t10.*t33+Ixz6.*dQ3.*dQ6.*t2.*t3.*t9.*t11.*t35;
et132 = Ixz6.*dQ3.*dQ6.*t2.*t6.*t8.*t10.*t34+Ixz6.*dQ3.*dQ6.*t3.*t6.*t7.*t10.*t34-Ixz6.*dQ4.*dQ6.*t2.*t4.*t8.*t11.*t35-Ixz6.*dQ4.*dQ6.*t3.*t4.*t7.*t11.*t35-Ixz6.*dQ2.*dQ3.*t7.*t8.*t10.*t11.*t34.*2.0-Ixz6.*dQ2.*dQ6.*t7.*t8.*t9.*t11.*t35-Ixz6.*dQ3.*dQ6.*t7.*t8.*t9.*t11.*t35-Ixz5.*dQ1.*dQ4.*t2.*t7.*t9.*t33.*t35.*4.0-Ixz5.*dQ1.*dQ4.*t3.*t8.*t9.*t32.*t35.*4.0-Ixz6.*dQ1.*dQ2.*t5.*t9.*t11.*t32.*t33.*4.0-Ixz6.*dQ1.*dQ3.*t5.*t9.*t11.*t32.*t33.*4.0-Ixz6.*dQ1.*dQ6.*t5.*t10.*t11.*t32.*t33.*2.0+Ixz6.*dQ1.*dQ6.*t5.*t10.*t11.*t32.*t34+Ixz6.*dQ1.*dQ6.*t5.*t10.*t11.*t33.*t34+Ixz6.*dQ1.*dQ2.*t4.*t6.*t32.*t33.*t35.*8.0+Ixz6.*dQ1.*dQ3.*t4.*t6.*t32.*t33.*t35.*8.0-Ixz6.*dQ1.*dQ4.*t10.*t11.*t32.*t33.*t34.*4.0+Ixz6.*dQ1.*dQ5.*t6.*t32.*t33.*t34.*t35.*4.0-Iyx5.*dQ1.*dQ2.*t2.*t4.*t5.*t7.*t9.*2.0;
et133 = Iyx5.*dQ1.*dQ4.*t2.*t3.*t5.*t7.*t8.*-2.0-Iyx5.*dQ1.*dQ3.*t2.*t4.*t5.*t7.*t9.*2.0+Iyx6.*dQ1.*dQ2.*t2.*t4.*t5.*t7.*t9.*2.0+Iyx6.*dQ1.*dQ4.*t2.*t3.*t5.*t7.*t8.*2.0-Iyx5.*dQ1.*dQ2.*t3.*t4.*t5.*t8.*t9.*2.0+Iyx6.*dQ1.*dQ3.*t2.*t4.*t5.*t7.*t9.*2.0-Iyx5.*dQ1.*dQ3.*t3.*t4.*t5.*t8.*t9.*2.0+Iyx6.*dQ1.*dQ2.*t3.*t4.*t5.*t8.*t9.*2.0+Iyx6.*dQ1.*dQ3.*t3.*t4.*t5.*t8.*t9.*2.0+Iyx6.*dQ1.*dQ6.*t2.*t4.*t5.*t7.*t10.*2.0+Iyx6.*dQ1.*dQ5.*t2.*t4.*t6.*t7.*t11.*2.0+Iyx6.*dQ1.*dQ6.*t3.*t4.*t5.*t8.*t10.*2.0+Iyx6.*dQ2.*dQ6.*t2.*t3.*t5.*t9.*t10+Iyx6.*dQ1.*dQ5.*t3.*t4.*t6.*t8.*t11.*2.0+Iyx6.*dQ3.*dQ6.*t2.*t3.*t5.*t9.*t10+Iyx6.*dQ1.*dQ2.*t4.*t5.*t6.*t10.*t11.*2.0-Iyx6.*dQ4.*dQ6.*t2.*t4.*t5.*t8.*t10-Iyx6.*dQ4.*dQ6.*t3.*t4.*t5.*t7.*t10+Iyx6.*dQ1.*dQ3.*t4.*t5.*t6.*t10.*t11.*2.0;
et134 = Iyx6.*dQ2.*dQ6.*t2.*t5.*t6.*t8.*t11.*2.0+Iyx6.*dQ2.*dQ6.*t3.*t5.*t6.*t7.*t11.*2.0-Iyx6.*dQ4.*dQ5.*t2.*t4.*t6.*t8.*t11.*2.0-Iyx6.*dQ4.*dQ5.*t3.*t4.*t6.*t7.*t11.*2.0+Iyx6.*dQ3.*dQ6.*t2.*t5.*t6.*t8.*t11.*2.0+Iyx6.*dQ3.*dQ6.*t3.*t5.*t6.*t7.*t11.*2.0-Iyx6.*dQ5.*dQ6.*t2.*t3.*t6.*t10.*t11.*2.0-Iyx6.*dQ2.*dQ6.*t5.*t7.*t8.*t9.*t10-Iyx6.*dQ3.*dQ6.*t5.*t7.*t8.*t9.*t10+Iyx6.*dQ5.*dQ6.*t6.*t7.*t8.*t10.*t11.*2.0+Iyx4.*dQ1.*dQ2.*t2.*t4.*t7.*t9.*t33.*4.0+Iyx4.*dQ1.*dQ2.*t3.*t4.*t8.*t9.*t32.*4.0+Iyx4.*dQ1.*dQ3.*t2.*t4.*t7.*t9.*t33.*4.0+Iyx4.*dQ1.*dQ4.*t2.*t3.*t7.*t8.*t34.*4.0+Iyx6.*dQ2.*dQ5.*t2.*t3.*t4.*t5.*t36.*2.0+Iyx4.*dQ1.*dQ3.*t3.*t4.*t8.*t9.*t32.*4.0+Iyx6.*dQ3.*dQ5.*t2.*t3.*t4.*t5.*t36.*2.0+Iyx5.*dQ1.*dQ4.*t2.*t4.*t7.*t10.*t33.*2.0+Iyx5.*dQ1.*dQ4.*t3.*t4.*t8.*t10.*t32.*2.0;
et135 = Iyx5.*dQ1.*dQ5.*t2.*t5.*t7.*t9.*t33.*2.0-Iyx6.*dQ1.*dQ4.*t2.*t4.*t7.*t10.*t33.*2.0-Iyx6.*dQ1.*dQ6.*t2.*t3.*t7.*t8.*t34.*2.0+Iyx5.*dQ1.*dQ5.*t3.*t5.*t8.*t9.*t32.*2.0-Iyx6.*dQ1.*dQ2.*t2.*t6.*t7.*t11.*t33.*8.0-Iyx6.*dQ1.*dQ4.*t3.*t4.*t8.*t10.*t32.*2.0-Iyx6.*dQ1.*dQ5.*t2.*t5.*t7.*t9.*t33.*2.0-Iyx6.*dQ1.*dQ6.*t2.*t3.*t7.*t8.*t35.*2.0-Iyx6.*dQ1.*dQ2.*t2.*t6.*t7.*t11.*t34.*2.0-Iyx6.*dQ1.*dQ2.*t3.*t6.*t8.*t11.*t32.*8.0-Iyx6.*dQ1.*dQ3.*t2.*t6.*t7.*t11.*t33.*8.0-Iyx6.*dQ1.*dQ5.*t3.*t5.*t8.*t9.*t32.*2.0-Iyx6.*dQ1.*dQ6.*t2.*t3.*t7.*t8.*t36.*8.0-Iyx6.*dQ1.*dQ2.*t2.*t6.*t7.*t11.*t35.*2.0-Iyx6.*dQ1.*dQ3.*t2.*t6.*t7.*t11.*t34.*2.0-Iyx6.*dQ1.*dQ3.*t3.*t6.*t8.*t11.*t32.*8.0-Iyx6.*dQ1.*dQ4.*t2.*t4.*t7.*t10.*t36.*2.0;
et136 = Iyx6.*dQ1.*dQ2.*t3.*t6.*t8.*t11.*t34.*-2.0-Iyx6.*dQ1.*dQ3.*t2.*t6.*t7.*t11.*t35.*2.0-Iyx6.*dQ1.*dQ5.*t2.*t5.*t7.*t9.*t36.*2.0-Iyx6.*dQ2.*dQ3.*t2.*t4.*t8.*t10.*t36.*2.0-Iyx6.*dQ2.*dQ3.*t3.*t4.*t7.*t10.*t36.*2.0-Iyx6.*dQ1.*dQ2.*t3.*t6.*t8.*t11.*t35.*2.0-Iyx6.*dQ1.*dQ3.*t3.*t6.*t8.*t11.*t34.*2.0-Iyx6.*dQ1.*dQ4.*t3.*t4.*t8.*t10.*t36.*2.0-Iyx6.*dQ1.*dQ3.*t3.*t6.*t8.*t11.*t35.*2.0-Iyx6.*dQ1.*dQ4.*t4.*t6.*t9.*t11.*t32.*2.0-Iyx6.*dQ1.*dQ5.*t3.*t5.*t8.*t9.*t36.*2.0-Iyx6.*dQ2.*dQ4.*t2.*t6.*t8.*t11.*t34.*2.0-Iyx6.*dQ2.*dQ4.*t3.*t6.*t7.*t11.*t34.*2.0-Iyx6.*dQ2.*dQ5.*t4.*t5.*t7.*t8.*t36.*2.0-Iyx6.*dQ2.*dQ6.*t2.*t4.*t8.*t9.*t36.*2.0-Iyx6.*dQ2.*dQ6.*t3.*t4.*t7.*t9.*t36.*2.0-Iyx6.*dQ1.*dQ4.*t4.*t6.*t9.*t11.*t33.*2.0+Iyx6.*dQ2.*dQ4.*t2.*t6.*t8.*t11.*t35.*2.0;
et137 = Iyx6.*dQ2.*dQ4.*t3.*t6.*t7.*t11.*t35.*2.0-Iyx6.*dQ3.*dQ4.*t2.*t6.*t8.*t11.*t34.*2.0-Iyx6.*dQ3.*dQ4.*t3.*t6.*t7.*t11.*t34.*2.0-Iyx6.*dQ3.*dQ5.*t4.*t5.*t7.*t8.*t36.*2.0-Iyx6.*dQ3.*dQ6.*t2.*t4.*t8.*t9.*t36.*2.0-Iyx6.*dQ3.*dQ6.*t3.*t4.*t7.*t9.*t36.*2.0+Iyx6.*dQ3.*dQ4.*t2.*t6.*t8.*t11.*t35.*2.0+Iyx6.*dQ3.*dQ4.*t3.*t6.*t7.*t11.*t35.*2.0-Iyx6.*dQ1.*dQ5.*t5.*t6.*t10.*t11.*t32.*2.0-Iyx6.*dQ1.*dQ5.*t5.*t6.*t10.*t11.*t33.*2.0+Iyx6.*dQ2.*dQ3.*t2.*t3.*t5.*t34.*t36.*4.0+Iyx5.*dQ1.*dQ5.*t4.*t9.*t10.*t32.*t33.*2.0-Iyx6.*dQ1.*dQ5.*t4.*t9.*t10.*t32.*t33.*2.0-Iyx6.*dQ2.*dQ3.*t5.*t7.*t8.*t34.*t36.*4.0-Iyx6.*dQ1.*dQ5.*t4.*t9.*t10.*t32.*t36.*2.0-Iyx6.*dQ2.*dQ5.*t2.*t8.*t10.*t34.*t36.*2.0-Iyx6.*dQ2.*dQ5.*t3.*t7.*t10.*t34.*t36.*2.0-Iyx6.*dQ1.*dQ5.*t4.*t9.*t10.*t33.*t36.*2.0;
et138 = Iyx6.*dQ3.*dQ5.*t2.*t8.*t10.*t34.*t36.*-2.0-Iyx6.*dQ3.*dQ5.*t3.*t7.*t10.*t34.*t36.*2.0+Iyx6.*dQ1.*dQ2.*t9.*t10.*t32.*t33.*t36.*8.0+Iyx6.*dQ1.*dQ3.*t9.*t10.*t32.*t33.*t36.*8.0-Iyx6.*dQ1.*dQ4.*t5.*t32.*t33.*t34.*t36.*8.0-Iyx6.*dQ1.*dQ6.*t32.*t33.*t34.*t35.*t36.*4.0-Iyy6.*dQ2.*dQ3.*t2.*t3.*t5.*t6.*t11.*2.0+Iyy6.*dQ1.*dQ4.*t2.*t5.*t7.*t9.*t10.*2.0+Iyy6.*dQ2.*dQ3.*t2.*t5.*t8.*t9.*t10.*2.0+Iyy6.*dQ2.*dQ3.*t3.*t5.*t7.*t9.*t10.*2.0+Iyy6.*dQ1.*dQ4.*t3.*t5.*t8.*t9.*t10.*2.0+Iyy6.*dQ2.*dQ3.*t5.*t6.*t7.*t8.*t11.*2.0-Iyy6.*dQ5.*dQ6.*t2.*t6.*t8.*t9.*t11.*2.0-Iyy6.*dQ5.*dQ6.*t3.*t6.*t7.*t9.*t11.*2.0-Iyy6.*dQ2.*dQ3.*t2.*t3.*t4.*t9.*t35.*2.0+Iyy6.*dQ2.*dQ3.*t2.*t3.*t4.*t9.*t36.*2.0+Iyy6.*dQ2.*dQ6.*t2.*t3.*t4.*t10.*t36.*2.0+Iyy6.*dQ3.*dQ6.*t2.*t3.*t4.*t10.*t36.*2.0;
et139 = Iyy6.*dQ4.*dQ5.*t2.*t3.*t5.*t10.*t36.*-2.0+Iyy6.*dQ5.*dQ6.*t2.*t4.*t5.*t8.*t36.*2.0+Iyy6.*dQ5.*dQ6.*t3.*t4.*t5.*t7.*t36.*2.0-Iyy6.*dQ4.*dQ6.*t2.*t3.*t6.*t11.*t35.*2.0-Iyy6.*dQ1.*dQ6.*t2.*t7.*t9.*t10.*t33.*4.0+Iyy6.*dQ2.*dQ3.*t4.*t7.*t8.*t9.*t35.*2.0-Iyy6.*dQ1.*dQ6.*t3.*t8.*t9.*t10.*t32.*4.0-Iyy6.*dQ2.*dQ3.*t4.*t7.*t8.*t9.*t36.*2.0-Iyy6.*dQ1.*dQ2.*t6.*t9.*t10.*t11.*t32.*4.0-Iyy6.*dQ1.*dQ6.*t2.*t7.*t9.*t10.*t36.*4.0-Iyy6.*dQ1.*dQ2.*t6.*t9.*t10.*t11.*t33.*4.0-Iyy6.*dQ1.*dQ3.*t6.*t9.*t10.*t11.*t32.*4.0-Iyy6.*dQ1.*dQ3.*t6.*t9.*t10.*t11.*t33.*4.0-Iyy6.*dQ1.*dQ6.*t3.*t8.*t9.*t10.*t36.*4.0-Iyy6.*dQ2.*dQ6.*t4.*t7.*t8.*t10.*t36.*2.0-Iyy6.*dQ3.*dQ6.*t4.*t7.*t8.*t10.*t36.*2.0+Iyy6.*dQ4.*dQ5.*t5.*t7.*t8.*t10.*t36.*2.0+Iyy6.*dQ4.*dQ6.*t2.*t8.*t9.*t10.*t36.*2.0;
et140 = Iyy6.*dQ4.*dQ6.*t3.*t7.*t9.*t10.*t36.*2.0+Iyy6.*dQ4.*dQ6.*t6.*t7.*t8.*t11.*t35.*2.0+Iyy6.*dQ1.*dQ2.*t4.*t5.*t10.*t32.*t33.*8.0+Iyy6.*dQ1.*dQ5.*t2.*t4.*t7.*t33.*t35.*8.0+Iyy6.*dQ1.*dQ3.*t4.*t5.*t10.*t32.*t33.*8.0+Iyy6.*dQ1.*dQ5.*t2.*t4.*t7.*t33.*t36.*4.0+Iyy6.*dQ1.*dQ5.*t3.*t4.*t8.*t32.*t35.*8.0+Iyy6.*dQ1.*dQ5.*t3.*t4.*t8.*t32.*t36.*4.0+Iyy6.*dQ1.*dQ2.*t4.*t5.*t10.*t32.*t36.*4.0+Iyy6.*dQ1.*dQ5.*t2.*t4.*t7.*t35.*t36.*4.0+Iyy6.*dQ1.*dQ6.*t4.*t5.*t9.*t32.*t33.*4.0+Iyy6.*dQ1.*dQ2.*t4.*t5.*t10.*t33.*t36.*4.0+Iyy6.*dQ1.*dQ3.*t4.*t5.*t10.*t32.*t36.*4.0+Iyy6.*dQ1.*dQ3.*t4.*t5.*t10.*t33.*t36.*4.0+Iyy6.*dQ1.*dQ4.*t5.*t6.*t11.*t32.*t33.*4.0+Iyy6.*dQ1.*dQ5.*t3.*t4.*t8.*t35.*t36.*4.0+Iyy6.*dQ2.*dQ5.*t2.*t3.*t9.*t35.*t36.*2.0+Iyy6.*dQ1.*dQ4.*t5.*t6.*t11.*t32.*t34.*4.0+Iyy6.*dQ1.*dQ6.*t4.*t5.*t9.*t32.*t36.*4.0;
et141 = Iyy6.*dQ2.*dQ6.*t2.*t5.*t8.*t34.*t36.*4.0+Iyy6.*dQ2.*dQ6.*t3.*t5.*t7.*t34.*t36.*4.0+Iyy6.*dQ3.*dQ5.*t2.*t3.*t9.*t35.*t36.*2.0+Iyy6.*dQ1.*dQ4.*t5.*t6.*t11.*t33.*t34.*4.0+Iyy6.*dQ1.*dQ6.*t4.*t5.*t9.*t33.*t36.*4.0+Iyy6.*dQ3.*dQ6.*t2.*t5.*t8.*t34.*t36.*4.0+Iyy6.*dQ3.*dQ6.*t3.*t5.*t7.*t34.*t36.*4.0-Iyy6.*dQ4.*dQ5.*t2.*t4.*t8.*t35.*t36.*2.0-Iyy6.*dQ4.*dQ5.*t3.*t4.*t7.*t35.*t36.*2.0-Iyy6.*dQ2.*dQ5.*t7.*t8.*t9.*t35.*t36.*2.0-Iyy6.*dQ3.*dQ5.*t7.*t8.*t9.*t35.*t36.*2.0+Iyy6.*dQ1.*dQ2.*t2.*t7.*t33.*t34.*t35.*4.0-Iyy6.*dQ1.*dQ2.*t2.*t7.*t33.*t34.*t36.*4.0+Iyy6.*dQ1.*dQ2.*t3.*t8.*t32.*t34.*t35.*4.0+Iyy6.*dQ1.*dQ3.*t2.*t7.*t33.*t34.*t35.*4.0-Iyy6.*dQ1.*dQ2.*t2.*t7.*t33.*t35.*t36.*4.0-Iyy6.*dQ1.*dQ2.*t3.*t8.*t32.*t34.*t36.*4.0-Iyy6.*dQ1.*dQ3.*t2.*t7.*t33.*t34.*t36.*4.0+Iyy6.*dQ1.*dQ3.*t3.*t8.*t32.*t34.*t35.*4.0;
et142 = Iyy6.*dQ1.*dQ2.*t2.*t7.*t34.*t35.*t36.*2.0-Iyy6.*dQ1.*dQ2.*t3.*t8.*t32.*t35.*t36.*4.0-Iyy6.*dQ1.*dQ3.*t2.*t7.*t33.*t35.*t36.*4.0-Iyy6.*dQ1.*dQ3.*t3.*t8.*t32.*t34.*t36.*4.0+Iyy6.*dQ1.*dQ3.*t2.*t7.*t34.*t35.*t36.*2.0-Iyy6.*dQ1.*dQ3.*t3.*t8.*t32.*t35.*t36.*4.0+Iyy6.*dQ1.*dQ4.*t4.*t9.*t32.*t33.*t35.*4.0+Iyy6.*dQ1.*dQ2.*t3.*t8.*t34.*t35.*t36.*2.0-Iyy6.*dQ1.*dQ4.*t4.*t9.*t32.*t33.*t36.*4.0+Iyy6.*dQ1.*dQ3.*t3.*t8.*t34.*t35.*t36.*2.0+Iyy6.*dQ1.*dQ5.*t5.*t10.*t32.*t33.*t34.*4.0+Iyy6.*dQ1.*dQ4.*t4.*t9.*t32.*t35.*t36.*2.0+Iyy6.*dQ2.*dQ4.*t2.*t8.*t34.*t35.*t36.*2.0+Iyy6.*dQ2.*dQ4.*t3.*t7.*t34.*t35.*t36.*2.0+Iyy6.*dQ1.*dQ4.*t4.*t9.*t33.*t35.*t36.*2.0-Iyy6.*dQ1.*dQ5.*t5.*t10.*t32.*t33.*t36.*4.0+Iyy6.*dQ3.*dQ4.*t2.*t8.*t34.*t35.*t36.*2.0+Iyy6.*dQ3.*dQ4.*t3.*t7.*t34.*t35.*t36.*2.0+Iyy6.*dQ1.*dQ5.*t5.*t10.*t32.*t34.*t36.*2.0;
et143 = Iyy6.*dQ1.*dQ6.*t6.*t11.*t32.*t33.*t34.*-4.0+Iyy6.*dQ1.*dQ5.*t5.*t10.*t33.*t34.*t36.*2.0-Iyy6.*dQ1.*dQ6.*t6.*t11.*t32.*t33.*t35.*4.0+Iyy6.*dQ1.*dQ6.*t6.*t11.*t32.*t34.*t35.*2.0+Iyy6.*dQ1.*dQ6.*t6.*t11.*t33.*t34.*t35.*2.0+Iyz6.*dQ1.*dQ4.*t2.*t4.*t5.*t6.*t7+Iyz4.*dQ1.*dQ2.*t2.*t3.*t7.*t8.*t9.*4.0+Iyz6.*dQ2.*dQ3.*t2.*t4.*t5.*t6.*t8+Iyz6.*dQ2.*dQ3.*t3.*t4.*t5.*t6.*t7+Iyz4.*dQ1.*dQ3.*t2.*t3.*t7.*t8.*t9.*4.0+Iyz6.*dQ1.*dQ4.*t3.*t4.*t5.*t6.*t8+Iyz6.*dQ2.*dQ5.*t2.*t3.*t4.*t6.*t10+Iyz6.*dQ3.*dQ5.*t2.*t3.*t4.*t6.*t10-Iyz5.*dQ1.*dQ2.*t2.*t4.*t7.*t9.*t10.*2.0-Iyz5.*dQ1.*dQ4.*t2.*t3.*t7.*t8.*t10.*2.0-Iyz5.*dQ1.*dQ3.*t2.*t4.*t7.*t9.*t10.*2.0-Iyz5.*dQ1.*dQ2.*t3.*t4.*t8.*t9.*t10.*2.0-Iyz6.*dQ4.*dQ6.*t2.*t3.*t5.*t6.*t10-Iyz5.*dQ1.*dQ3.*t3.*t4.*t8.*t9.*t10.*2.0;
et144 = Iyz6.*dQ1.*dQ5.*t2.*t3.*t7.*t8.*t11.*-2.0-Iyz6.*dQ1.*dQ2.*t2.*t5.*t7.*t10.*t11.*2.0-Iyz6.*dQ1.*dQ3.*t2.*t5.*t7.*t10.*t11.*2.0-Iyz6.*dQ1.*dQ2.*t3.*t5.*t8.*t10.*t11.*2.0-Iyz6.*dQ1.*dQ5.*t2.*t6.*t7.*t9.*t10-Iyz6.*dQ1.*dQ3.*t3.*t5.*t8.*t10.*t11.*2.0-Iyz6.*dQ1.*dQ6.*t2.*t5.*t7.*t9.*t11-Iyz6.*dQ1.*dQ5.*t3.*t6.*t8.*t9.*t10+Iyz6.*dQ2.*dQ4.*t2.*t5.*t8.*t10.*t11.*2.0+Iyz6.*dQ2.*dQ4.*t3.*t5.*t7.*t10.*t11.*2.0-Iyz6.*dQ2.*dQ5.*t4.*t6.*t7.*t8.*t10-Iyz6.*dQ1.*dQ6.*t3.*t5.*t8.*t9.*t11+Iyz6.*dQ3.*dQ4.*t2.*t5.*t8.*t10.*t11.*2.0+Iyz6.*dQ3.*dQ4.*t3.*t5.*t7.*t10.*t11.*2.0-Iyz6.*dQ3.*dQ5.*t4.*t6.*t7.*t8.*t10+Iyz6.*dQ4.*dQ6.*t2.*t5.*t8.*t9.*t11+Iyz6.*dQ4.*dQ6.*t3.*t5.*t7.*t9.*t11+Iyz6.*dQ4.*dQ6.*t5.*t6.*t7.*t8.*t10-Iyz5.*dQ1.*dQ4.*t2.*t4.*t5.*t7.*t33.*2.0;
et145 = Iyz5.*dQ1.*dQ4.*t3.*t4.*t5.*t8.*t32.*-2.0+Iyz6.*dQ1.*dQ6.*t2.*t4.*t6.*t7.*t33.*2.0+Iyz6.*dQ1.*dQ6.*t3.*t4.*t6.*t8.*t32.*2.0+Iyz6.*dQ2.*dQ3.*t2.*t3.*t6.*t10.*t34.*2.0+Iyz6.*dQ1.*dQ6.*t2.*t4.*t6.*t7.*t35.*2.0+Iyz6.*dQ1.*dQ5.*t4.*t5.*t6.*t9.*t32+Iyz6.*dQ2.*dQ5.*t2.*t5.*t6.*t8.*t34+Iyz6.*dQ2.*dQ5.*t3.*t5.*t6.*t7.*t34+Iyz6.*dQ1.*dQ5.*t4.*t5.*t6.*t9.*t33+Iyz6.*dQ1.*dQ6.*t3.*t4.*t6.*t8.*t35.*2.0+Iyz6.*dQ2.*dQ6.*t2.*t3.*t6.*t9.*t35+Iyz6.*dQ3.*dQ5.*t2.*t5.*t6.*t8.*t34+Iyz6.*dQ3.*dQ5.*t3.*t5.*t6.*t7.*t34+Iyz6.*dQ3.*dQ6.*t2.*t3.*t6.*t9.*t35-Iyz6.*dQ4.*dQ6.*t2.*t4.*t6.*t8.*t35-Iyz6.*dQ4.*dQ6.*t3.*t4.*t6.*t7.*t35+Iyz5.*dQ1.*dQ5.*t2.*t7.*t9.*t10.*t33.*2.0+Iyz5.*dQ1.*dQ5.*t3.*t8.*t9.*t10.*t32.*2.0-Iyz6.*dQ1.*dQ4.*t2.*t7.*t9.*t11.*t33.*2.0-Iyz6.*dQ1.*dQ4.*t3.*t8.*t9.*t11.*t32.*2.0;
et146 = Iyz6.*dQ1.*dQ4.*t2.*t7.*t9.*t11.*t35.*-2.0-Iyz6.*dQ2.*dQ3.*t2.*t8.*t9.*t11.*t35.*2.0-Iyz6.*dQ2.*dQ3.*t3.*t7.*t9.*t11.*t35.*2.0-Iyz6.*dQ2.*dQ3.*t6.*t7.*t8.*t10.*t34.*2.0-Iyz6.*dQ1.*dQ4.*t3.*t8.*t9.*t11.*t35.*2.0-Iyz6.*dQ1.*dQ6.*t4.*t9.*t10.*t11.*t32-Iyz6.*dQ2.*dQ6.*t2.*t8.*t10.*t11.*t34-Iyz6.*dQ2.*dQ6.*t3.*t7.*t10.*t11.*t34-Iyz6.*dQ2.*dQ6.*t6.*t7.*t8.*t9.*t35-Iyz6.*dQ1.*dQ6.*t4.*t9.*t10.*t11.*t33-Iyz6.*dQ3.*dQ6.*t2.*t8.*t10.*t11.*t34-Iyz6.*dQ3.*dQ6.*t3.*t7.*t10.*t11.*t34-Iyz6.*dQ3.*dQ6.*t6.*t7.*t8.*t9.*t35-Iyz5.*dQ1.*dQ5.*t4.*t5.*t9.*t32.*t33.*2.0-Iyz6.*dQ1.*dQ2.*t5.*t6.*t9.*t32.*t33.*4.0-Iyz6.*dQ1.*dQ3.*t5.*t6.*t9.*t32.*t33.*4.0-Iyz6.*dQ1.*dQ6.*t5.*t6.*t10.*t32.*t33.*2.0+Iyz6.*dQ1.*dQ6.*t5.*t6.*t10.*t32.*t34;
et147 = Iyz6.*dQ1.*dQ6.*t5.*t6.*t10.*t33.*t34-Iyz6.*dQ1.*dQ2.*t4.*t11.*t32.*t33.*t35.*8.0-Iyz6.*dQ1.*dQ3.*t4.*t11.*t32.*t33.*t35.*8.0-Iyz6.*dQ1.*dQ4.*t6.*t10.*t32.*t33.*t34.*4.0-Iyz6.*dQ1.*dQ5.*t11.*t32.*t33.*t34.*t35.*4.0-Izx4.*dQ1.*dQ2.*t2.*t3.*t4.*t7.*t8.*4.0-Izx4.*dQ1.*dQ3.*t2.*t3.*t4.*t7.*t8.*4.0+Izx5.*dQ1.*dQ2.*t2.*t3.*t4.*t7.*t8.*4.0+Izx5.*dQ1.*dQ3.*t2.*t3.*t4.*t7.*t8.*4.0+Izx6.*dQ1.*dQ5.*t2.*t3.*t6.*t7.*t8.*2.0+Izx5.*dQ1.*dQ5.*t2.*t4.*t5.*t7.*t10.*4.0+Izx6.*dQ1.*dQ2.*t2.*t5.*t6.*t7.*t10.*2.0+Izx6.*dQ1.*dQ3.*t2.*t5.*t6.*t7.*t10.*2.0+Izx6.*dQ1.*dQ4.*t2.*t4.*t5.*t7.*t11+Izx5.*dQ1.*dQ5.*t3.*t4.*t5.*t8.*t10.*4.0+Izx6.*dQ1.*dQ2.*t3.*t5.*t6.*t8.*t10.*2.0+Izx6.*dQ2.*dQ3.*t2.*t4.*t5.*t8.*t11+Izx6.*dQ2.*dQ3.*t3.*t4.*t5.*t7.*t11+Izx6.*dQ1.*dQ3.*t3.*t5.*t6.*t8.*t10.*2.0;
et148 = Izx6.*dQ1.*dQ4.*t3.*t4.*t5.*t8.*t11+Izx6.*dQ1.*dQ6.*t2.*t5.*t6.*t7.*t9-Izx5.*dQ4.*dQ5.*t2.*t4.*t5.*t8.*t10.*2.0-Izx5.*dQ4.*dQ5.*t3.*t4.*t5.*t7.*t10.*2.0-Izx6.*dQ2.*dQ4.*t2.*t5.*t6.*t8.*t10.*2.0-Izx6.*dQ2.*dQ4.*t3.*t5.*t6.*t7.*t10.*2.0+Izx6.*dQ2.*dQ5.*t2.*t3.*t4.*t10.*t11+Izx6.*dQ1.*dQ6.*t3.*t5.*t6.*t8.*t9-Izx6.*dQ3.*dQ4.*t2.*t5.*t6.*t8.*t10.*2.0-Izx6.*dQ3.*dQ4.*t3.*t5.*t6.*t7.*t10.*2.0+Izx6.*dQ3.*dQ5.*t2.*t3.*t4.*t10.*t11-Izx6.*dQ4.*dQ6.*t2.*t5.*t6.*t8.*t9-Izx6.*dQ4.*dQ6.*t3.*t5.*t6.*t7.*t9-Izx6.*dQ4.*dQ6.*t2.*t3.*t5.*t10.*t11-Izx6.*dQ1.*dQ5.*t2.*t7.*t9.*t10.*t11-Izx6.*dQ1.*dQ5.*t3.*t8.*t9.*t10.*t11-Izx6.*dQ2.*dQ5.*t4.*t7.*t8.*t10.*t11-Izx6.*dQ3.*dQ5.*t4.*t7.*t8.*t10.*t11+Izx6.*dQ4.*dQ6.*t5.*t7.*t8.*t10.*t11;
et149 = Izx5.*dQ1.*dQ2.*t2.*t5.*t7.*t10.*t33.*-4.0+Izx5.*dQ1.*dQ5.*t2.*t3.*t7.*t8.*t34.*2.0+Izx5.*dQ1.*dQ2.*t2.*t5.*t7.*t10.*t34.*2.0-Izx5.*dQ1.*dQ2.*t3.*t5.*t8.*t10.*t32.*4.0-Izx5.*dQ1.*dQ3.*t2.*t5.*t7.*t10.*t33.*4.0-Izx5.*dQ1.*dQ5.*t2.*t3.*t7.*t8.*t35.*4.0+Izx5.*dQ1.*dQ3.*t2.*t5.*t7.*t10.*t34.*2.0-Izx5.*dQ1.*dQ3.*t3.*t5.*t8.*t10.*t32.*4.0+Izx5.*dQ1.*dQ2.*t3.*t5.*t8.*t10.*t34.*2.0+Izx6.*dQ1.*dQ4.*t2.*t6.*t7.*t9.*t33.*2.0+Izx5.*dQ1.*dQ3.*t3.*t5.*t8.*t10.*t34.*2.0+Izx6.*dQ1.*dQ4.*t3.*t6.*t8.*t9.*t32.*2.0+Izx5.*dQ1.*dQ4.*t4.*t5.*t9.*t10.*t32.*2.0+Izx5.*dQ2.*dQ4.*t2.*t5.*t8.*t10.*t34.*2.0+Izx5.*dQ2.*dQ4.*t3.*t5.*t7.*t10.*t34.*2.0+Izx6.*dQ1.*dQ4.*t2.*t6.*t7.*t9.*t35.*2.0+Izx6.*dQ1.*dQ6.*t2.*t4.*t7.*t11.*t33.*2.0+Izx5.*dQ1.*dQ4.*t4.*t5.*t9.*t10.*t33.*2.0+Izx5.*dQ3.*dQ4.*t2.*t5.*t8.*t10.*t34.*2.0;
et150 = Izx5.*dQ3.*dQ4.*t3.*t5.*t7.*t10.*t34.*2.0+Izx6.*dQ1.*dQ6.*t3.*t4.*t8.*t11.*t32.*2.0+Izx6.*dQ2.*dQ3.*t2.*t3.*t10.*t11.*t34.*2.0+Izx6.*dQ2.*dQ3.*t2.*t6.*t8.*t9.*t35.*2.0+Izx6.*dQ2.*dQ3.*t3.*t6.*t7.*t9.*t35.*2.0+Izx6.*dQ1.*dQ4.*t3.*t6.*t8.*t9.*t35.*2.0+Izx6.*dQ1.*dQ6.*t2.*t4.*t7.*t11.*t35.*2.0+Izx6.*dQ1.*dQ5.*t4.*t5.*t9.*t11.*t32+Izx6.*dQ2.*dQ5.*t2.*t5.*t8.*t11.*t34+Izx6.*dQ2.*dQ5.*t3.*t5.*t7.*t11.*t34+Izx6.*dQ1.*dQ5.*t4.*t5.*t9.*t11.*t33+Izx6.*dQ1.*dQ6.*t3.*t4.*t8.*t11.*t35.*2.0+Izx6.*dQ1.*dQ6.*t4.*t6.*t9.*t10.*t32+Izx6.*dQ2.*dQ6.*t2.*t3.*t9.*t11.*t35+Izx6.*dQ2.*dQ6.*t2.*t6.*t8.*t10.*t34+Izx6.*dQ2.*dQ6.*t3.*t6.*t7.*t10.*t34+Izx6.*dQ3.*dQ5.*t2.*t5.*t8.*t11.*t34+Izx6.*dQ3.*dQ5.*t3.*t5.*t7.*t11.*t34+Izx6.*dQ1.*dQ6.*t4.*t6.*t9.*t10.*t33+Izx6.*dQ3.*dQ6.*t2.*t3.*t9.*t11.*t35+Izx6.*dQ3.*dQ6.*t2.*t6.*t8.*t10.*t34;
et151 = Izx6.*dQ3.*dQ6.*t3.*t6.*t7.*t10.*t34-Izx6.*dQ4.*dQ6.*t2.*t4.*t8.*t11.*t35-Izx6.*dQ4.*dQ6.*t3.*t4.*t7.*t11.*t35-Izx6.*dQ2.*dQ3.*t7.*t8.*t10.*t11.*t34.*2.0-Izx6.*dQ2.*dQ6.*t7.*t8.*t9.*t11.*t35-Izx6.*dQ3.*dQ6.*t7.*t8.*t9.*t11.*t35-Izx5.*dQ1.*dQ4.*t2.*t7.*t9.*t33.*t35.*4.0-Izx5.*dQ1.*dQ4.*t3.*t8.*t9.*t32.*t35.*4.0-Izx6.*dQ1.*dQ2.*t5.*t9.*t11.*t32.*t33.*4.0-Izx6.*dQ1.*dQ3.*t5.*t9.*t11.*t32.*t33.*4.0-Izx6.*dQ1.*dQ6.*t5.*t10.*t11.*t32.*t33.*2.0+Izx6.*dQ1.*dQ6.*t5.*t10.*t11.*t32.*t34+Izx6.*dQ1.*dQ6.*t5.*t10.*t11.*t33.*t34+Izx6.*dQ1.*dQ2.*t4.*t6.*t32.*t33.*t35.*8.0+Izx6.*dQ1.*dQ3.*t4.*t6.*t32.*t33.*t35.*8.0-Izx6.*dQ1.*dQ4.*t10.*t11.*t32.*t33.*t34.*4.0+Izx6.*dQ1.*dQ5.*t6.*t32.*t33.*t34.*t35.*4.0+Izy6.*dQ1.*dQ4.*t2.*t4.*t5.*t6.*t7+Izy4.*dQ1.*dQ2.*t2.*t3.*t7.*t8.*t9.*4.0;
et152 = Izy6.*dQ2.*dQ3.*t2.*t4.*t5.*t6.*t8+Izy6.*dQ2.*dQ3.*t3.*t4.*t5.*t6.*t7+Izy4.*dQ1.*dQ3.*t2.*t3.*t7.*t8.*t9.*4.0+Izy6.*dQ1.*dQ4.*t3.*t4.*t5.*t6.*t8+Izy6.*dQ2.*dQ5.*t2.*t3.*t4.*t6.*t10+Izy6.*dQ3.*dQ5.*t2.*t3.*t4.*t6.*t10-Izy5.*dQ1.*dQ2.*t2.*t4.*t7.*t9.*t10.*2.0-Izy5.*dQ1.*dQ4.*t2.*t3.*t7.*t8.*t10.*2.0-Izy5.*dQ1.*dQ3.*t2.*t4.*t7.*t9.*t10.*2.0-Izy5.*dQ1.*dQ2.*t3.*t4.*t8.*t9.*t10.*2.0-Izy6.*dQ4.*dQ6.*t2.*t3.*t5.*t6.*t10-Izy5.*dQ1.*dQ3.*t3.*t4.*t8.*t9.*t10.*2.0-Izy6.*dQ1.*dQ5.*t2.*t3.*t7.*t8.*t11.*2.0-Izy6.*dQ1.*dQ2.*t2.*t5.*t7.*t10.*t11.*2.0-Izy6.*dQ1.*dQ3.*t2.*t5.*t7.*t10.*t11.*2.0-Izy6.*dQ1.*dQ2.*t3.*t5.*t8.*t10.*t11.*2.0-Izy6.*dQ1.*dQ5.*t2.*t6.*t7.*t9.*t10-Izy6.*dQ1.*dQ3.*t3.*t5.*t8.*t10.*t11.*2.0-Izy6.*dQ1.*dQ6.*t2.*t5.*t7.*t9.*t11;
et153 = -Izy6.*dQ1.*dQ5.*t3.*t6.*t8.*t9.*t10+Izy6.*dQ2.*dQ4.*t2.*t5.*t8.*t10.*t11.*2.0+Izy6.*dQ2.*dQ4.*t3.*t5.*t7.*t10.*t11.*2.0-Izy6.*dQ2.*dQ5.*t4.*t6.*t7.*t8.*t10-Izy6.*dQ1.*dQ6.*t3.*t5.*t8.*t9.*t11+Izy6.*dQ3.*dQ4.*t2.*t5.*t8.*t10.*t11.*2.0+Izy6.*dQ3.*dQ4.*t3.*t5.*t7.*t10.*t11.*2.0-Izy6.*dQ3.*dQ5.*t4.*t6.*t7.*t8.*t10+Izy6.*dQ4.*dQ6.*t2.*t5.*t8.*t9.*t11+Izy6.*dQ4.*dQ6.*t3.*t5.*t7.*t9.*t11+Izy6.*dQ4.*dQ6.*t5.*t6.*t7.*t8.*t10-Izy5.*dQ1.*dQ4.*t2.*t4.*t5.*t7.*t33.*2.0-Izy5.*dQ1.*dQ4.*t3.*t4.*t5.*t8.*t32.*2.0+Izy6.*dQ1.*dQ6.*t2.*t4.*t6.*t7.*t33.*2.0+Izy6.*dQ1.*dQ6.*t3.*t4.*t6.*t8.*t32.*2.0+Izy6.*dQ2.*dQ3.*t2.*t3.*t6.*t10.*t34.*2.0+Izy6.*dQ1.*dQ6.*t2.*t4.*t6.*t7.*t35.*2.0+Izy6.*dQ1.*dQ5.*t4.*t5.*t6.*t9.*t32+Izy6.*dQ2.*dQ5.*t2.*t5.*t6.*t8.*t34+Izy6.*dQ2.*dQ5.*t3.*t5.*t6.*t7.*t34;
et154 = Izy6.*dQ1.*dQ5.*t4.*t5.*t6.*t9.*t33+Izy6.*dQ1.*dQ6.*t3.*t4.*t6.*t8.*t35.*2.0+Izy6.*dQ2.*dQ6.*t2.*t3.*t6.*t9.*t35+Izy6.*dQ3.*dQ5.*t2.*t5.*t6.*t8.*t34+Izy6.*dQ3.*dQ5.*t3.*t5.*t6.*t7.*t34+Izy6.*dQ3.*dQ6.*t2.*t3.*t6.*t9.*t35-Izy6.*dQ4.*dQ6.*t2.*t4.*t6.*t8.*t35-Izy6.*dQ4.*dQ6.*t3.*t4.*t6.*t7.*t35+Izy5.*dQ1.*dQ5.*t2.*t7.*t9.*t10.*t33.*2.0+Izy5.*dQ1.*dQ5.*t3.*t8.*t9.*t10.*t32.*2.0-Izy6.*dQ1.*dQ4.*t2.*t7.*t9.*t11.*t33.*2.0-Izy6.*dQ1.*dQ4.*t3.*t8.*t9.*t11.*t32.*2.0-Izy6.*dQ1.*dQ4.*t2.*t7.*t9.*t11.*t35.*2.0-Izy6.*dQ2.*dQ3.*t2.*t8.*t9.*t11.*t35.*2.0-Izy6.*dQ2.*dQ3.*t3.*t7.*t9.*t11.*t35.*2.0-Izy6.*dQ2.*dQ3.*t6.*t7.*t8.*t10.*t34.*2.0-Izy6.*dQ1.*dQ4.*t3.*t8.*t9.*t11.*t35.*2.0-Izy6.*dQ1.*dQ6.*t4.*t9.*t10.*t11.*t32-Izy6.*dQ2.*dQ6.*t2.*t8.*t10.*t11.*t34;
et155 = -Izy6.*dQ2.*dQ6.*t3.*t7.*t10.*t11.*t34-Izy6.*dQ2.*dQ6.*t6.*t7.*t8.*t9.*t35-Izy6.*dQ1.*dQ6.*t4.*t9.*t10.*t11.*t33-Izy6.*dQ3.*dQ6.*t2.*t8.*t10.*t11.*t34-Izy6.*dQ3.*dQ6.*t3.*t7.*t10.*t11.*t34-Izy6.*dQ3.*dQ6.*t6.*t7.*t8.*t9.*t35-Izy5.*dQ1.*dQ5.*t4.*t5.*t9.*t32.*t33.*2.0-Izy6.*dQ1.*dQ2.*t5.*t6.*t9.*t32.*t33.*4.0-Izy6.*dQ1.*dQ3.*t5.*t6.*t9.*t32.*t33.*4.0-Izy6.*dQ1.*dQ6.*t5.*t6.*t10.*t32.*t33.*2.0+Izy6.*dQ1.*dQ6.*t5.*t6.*t10.*t32.*t34+Izy6.*dQ1.*dQ6.*t5.*t6.*t10.*t33.*t34-Izy6.*dQ1.*dQ2.*t4.*t11.*t32.*t33.*t35.*8.0-Izy6.*dQ1.*dQ3.*t4.*t11.*t32.*t33.*t35.*8.0-Izy6.*dQ1.*dQ4.*t6.*t10.*t32.*t33.*t34.*4.0-Izy6.*dQ1.*dQ5.*t11.*t32.*t33.*t34.*t35.*4.0-Izz5.*dQ1.*dQ4.*t2.*t5.*t7.*t9.*t10.*2.0-Izz5.*dQ2.*dQ3.*t2.*t5.*t8.*t9.*t10.*2.0;
et156 = Izz5.*dQ2.*dQ3.*t3.*t5.*t7.*t9.*t10.*-2.0-Izz6.*dQ1.*dQ4.*t2.*t5.*t7.*t9.*t10.*2.0-Izz5.*dQ1.*dQ4.*t3.*t5.*t8.*t9.*t10.*2.0-Izz6.*dQ2.*dQ3.*t2.*t5.*t8.*t9.*t10.*2.0-Izz6.*dQ2.*dQ3.*t3.*t5.*t7.*t9.*t10.*2.0-Izz6.*dQ1.*dQ4.*t3.*t5.*t8.*t9.*t10.*2.0+Izz5.*dQ2.*dQ3.*t2.*t3.*t4.*t9.*t35.*2.0+Izz6.*dQ2.*dQ3.*t2.*t3.*t4.*t9.*t35.*2.0-Izz5.*dQ2.*dQ3.*t4.*t7.*t8.*t9.*t35.*2.0-Izz6.*dQ2.*dQ3.*t4.*t7.*t8.*t9.*t35.*2.0-Izz5.*dQ1.*dQ2.*t4.*t5.*t10.*t32.*t33.*8.0-Izz5.*dQ1.*dQ5.*t2.*t4.*t7.*t33.*t35.*8.0-Izz5.*dQ1.*dQ3.*t4.*t5.*t10.*t32.*t33.*8.0-Izz5.*dQ1.*dQ5.*t3.*t4.*t8.*t32.*t35.*8.0-Izz6.*dQ1.*dQ2.*t4.*t5.*t10.*t32.*t33.*8.0-Izz6.*dQ1.*dQ5.*t2.*t4.*t7.*t33.*t35.*8.0-Izz6.*dQ1.*dQ3.*t4.*t5.*t10.*t32.*t33.*8.0;
et157 = Izz6.*dQ1.*dQ5.*t3.*t4.*t8.*t32.*t35.*-8.0-Izz5.*dQ1.*dQ2.*t2.*t7.*t33.*t34.*t35.*4.0-Izz5.*dQ1.*dQ2.*t3.*t8.*t32.*t34.*t35.*4.0-Izz5.*dQ1.*dQ3.*t2.*t7.*t33.*t34.*t35.*4.0-Izz6.*dQ1.*dQ2.*t2.*t7.*t33.*t34.*t35.*4.0-Izz5.*dQ1.*dQ3.*t3.*t8.*t32.*t34.*t35.*4.0-Izz6.*dQ1.*dQ2.*t3.*t8.*t32.*t34.*t35.*4.0-Izz6.*dQ1.*dQ3.*t2.*t7.*t33.*t34.*t35.*4.0-Izz6.*dQ1.*dQ3.*t3.*t8.*t32.*t34.*t35.*4.0-Izz5.*dQ1.*dQ4.*t4.*t9.*t32.*t33.*t35.*4.0-Izz6.*dQ1.*dQ4.*t4.*t9.*t32.*t33.*t35.*4.0-Izz5.*dQ1.*dQ5.*t5.*t10.*t32.*t33.*t34.*4.0-Izz6.*dQ1.*dQ5.*t5.*t10.*t32.*t33.*t34.*4.0+dQ2.*dQ3.*m4.*t2.*t3.*t4.*t9.*t15.*2.0-dQ2.*dQ3.*m4.*t2.*t3.*t4.*t9.*t18.*2.0-dQ2.*dQ3.*m6.*t2.*t3.*t4.*t9.*t17.*2.0-dQ2.*dQ3.*m5.*t2.*t3.*t4.*t9.*t19.*2.0-dQ2.*dQ6.*m6.*t2.*t3.*t4.*t10.*t17.*2.0;
et158 = dQ4.*dQ5.*m5.*t2.*t3.*t5.*t10.*t16.*-2.0+dQ2.*dQ3.*m6.*t2.*t3.*t4.*t9.*t22.*2.0-dQ3.*dQ6.*m6.*t2.*t3.*t4.*t10.*t17.*2.0-dQ2.*dQ3.*m4.*t4.*t7.*t8.*t9.*t15.*2.0+dQ2.*dQ3.*m5.*t2.*t3.*t4.*t9.*t25.*2.0-dQ5.*dQ6.*m6.*t2.*t4.*t5.*t8.*t17.*2.0-dQ5.*dQ6.*m6.*t3.*t4.*t5.*t7.*t17.*2.0+dQ2.*dQ3.*m4.*t4.*t7.*t8.*t9.*t18.*2.0+dQ2.*dQ3.*m6.*t2.*t3.*t4.*t9.*t26.*2.0-dQ4.*dQ5.*m6.*t2.*t3.*t5.*t10.*t20.*2.0+dQ4.*dQ6.*m6.*t2.*t3.*t6.*t11.*t17.*2.0+dQ2.*dQ3.*m6.*t4.*t7.*t8.*t9.*t17.*2.0+dQ2.*dQ3.*m5.*t4.*t7.*t8.*t9.*t19.*2.0+dQ4.*dQ5.*m6.*t2.*t3.*t5.*t10.*t22.*2.0+dQ1.*dQ6.*m6.*t2.*t7.*t9.*t10.*t17.*2.0-dQ4.*dQ6.*m6.*t2.*t3.*t6.*t11.*t20.*2.0+dQ4.*dQ5.*m5.*t2.*t3.*t5.*t10.*t25.*2.0+dQ1.*dQ6.*m6.*t3.*t8.*t9.*t10.*t17.*2.0+dQ2.*dQ6.*m6.*t4.*t7.*t8.*t10.*t17.*2.0;
et159 = dQ4.*dQ5.*m5.*t5.*t7.*t8.*t10.*t16.*2.0-dQ1.*dQ6.*m6.*t2.*t7.*t9.*t10.*t20.*2.0-dQ2.*dQ3.*m6.*t4.*t7.*t8.*t9.*t22.*2.0+dQ3.*dQ6.*m6.*t4.*t7.*t8.*t10.*t17.*2.0+dQ4.*dQ5.*m6.*t2.*t3.*t5.*t10.*t26.*2.0+dQ1.*dQ2.*m6.*t6.*t9.*t10.*t11.*t17.*2.0+dQ1.*dQ3.*m6.*t6.*t9.*t10.*t11.*t17.*2.0-dQ1.*dQ6.*m6.*t3.*t8.*t9.*t10.*t20.*2.0-dQ2.*dQ3.*m5.*t4.*t7.*t8.*t9.*t25.*2.0-dQ1.*dQ2.*m6.*t6.*t9.*t10.*t11.*t20.*2.0-dQ2.*dQ3.*m6.*t4.*t7.*t8.*t9.*t26.*2.0+dQ4.*dQ5.*m6.*t5.*t7.*t8.*t10.*t20.*2.0+dQ4.*dQ6.*m6.*t2.*t8.*t9.*t10.*t20.*2.0+dQ4.*dQ6.*m6.*t3.*t7.*t9.*t10.*t20.*2.0-dQ4.*dQ6.*m6.*t6.*t7.*t8.*t11.*t17.*2.0-dQ1.*dQ3.*m6.*t6.*t9.*t10.*t11.*t20.*2.0-dQ4.*dQ5.*m6.*t5.*t7.*t8.*t10.*t22.*2.0+dQ4.*dQ6.*m6.*t6.*t7.*t8.*t11.*t20.*2.0-dQ4.*dQ5.*m5.*t5.*t7.*t8.*t10.*t25.*2.0;
et160 = dQ4.*dQ5.*m6.*t5.*t7.*t8.*t10.*t26.*-2.0+dQ1.*dQ5.*m5.*t2.*t4.*t7.*t16.*t33.*4.0+dQ1.*dQ5.*m5.*t3.*t4.*t8.*t16.*t32.*4.0+dQ1.*dQ2.*m5.*t4.*t5.*t10.*t16.*t32.*4.0+dQ1.*dQ5.*m5.*t2.*t4.*t7.*t16.*t35.*4.0+dQ1.*dQ2.*m5.*t4.*t5.*t10.*t16.*t33.*4.0+dQ1.*dQ3.*m5.*t4.*t5.*t10.*t16.*t32.*4.0+dQ1.*dQ3.*m5.*t4.*t5.*t10.*t16.*t33.*4.0+dQ1.*dQ5.*m5.*t3.*t4.*t8.*t16.*t35.*4.0+dQ2.*dQ5.*m5.*t2.*t3.*t9.*t16.*t35.*2.0-dQ1.*dQ5.*m6.*t2.*t4.*t7.*t17.*t36.*2.0+dQ1.*dQ5.*m6.*t2.*t4.*t7.*t20.*t33.*4.0+dQ3.*dQ5.*m5.*t2.*t3.*t9.*t16.*t35.*2.0+dQ1.*dQ5.*m6.*t3.*t4.*t8.*t20.*t32.*4.0-dQ4.*dQ5.*m5.*t2.*t4.*t8.*t16.*t35.*2.0-dQ4.*dQ5.*m5.*t3.*t4.*t7.*t16.*t35.*2.0+dQ1.*dQ2.*m6.*t4.*t5.*t10.*t20.*t32.*4.0+dQ1.*dQ5.*m6.*t2.*t4.*t7.*t20.*t35.*4.0-dQ1.*dQ5.*m6.*t2.*t4.*t7.*t22.*t33.*4.0;
et161 = dQ1.*dQ5.*m6.*t3.*t4.*t8.*t17.*t36.*-2.0-dQ1.*dQ6.*m6.*t4.*t5.*t9.*t17.*t32.*2.0-dQ2.*dQ6.*m6.*t2.*t5.*t8.*t17.*t34.*2.0-dQ2.*dQ6.*m6.*t3.*t5.*t7.*t17.*t34.*2.0-dQ1.*dQ2.*m6.*t4.*t5.*t10.*t17.*t36.*2.0+dQ1.*dQ2.*m6.*t4.*t5.*t10.*t20.*t33.*4.0+dQ1.*dQ3.*m6.*t4.*t5.*t10.*t20.*t32.*4.0+dQ1.*dQ5.*m6.*t2.*t4.*t7.*t20.*t36.*2.0-dQ1.*dQ5.*m6.*t3.*t4.*t8.*t22.*t32.*4.0-dQ1.*dQ6.*m6.*t4.*t5.*t9.*t17.*t33.*2.0-dQ3.*dQ6.*m6.*t2.*t5.*t8.*t17.*t34.*2.0-dQ3.*dQ6.*m6.*t3.*t5.*t7.*t17.*t34.*2.0-dQ1.*dQ2.*m6.*t4.*t5.*t10.*t22.*t32.*4.0-dQ1.*dQ3.*m6.*t4.*t5.*t10.*t17.*t36.*2.0+dQ1.*dQ3.*m6.*t4.*t5.*t10.*t20.*t33.*4.0-dQ1.*dQ4.*m6.*t5.*t6.*t11.*t17.*t32.*2.0-dQ1.*dQ5.*m5.*t2.*t4.*t7.*t25.*t33.*4.0-dQ1.*dQ5.*m6.*t2.*t4.*t7.*t22.*t35.*4.0;
et162 = dQ1.*dQ5.*m6.*t3.*t4.*t8.*t20.*t35.*4.0+dQ2.*dQ5.*m6.*t2.*t3.*t9.*t20.*t35.*2.0-dQ2.*dQ6.*m6.*t2.*t5.*t8.*t17.*t36.*2.0-dQ2.*dQ6.*m6.*t3.*t5.*t7.*t17.*t36.*2.0+dQ4.*dQ5.*m6.*t2.*t4.*t8.*t17.*t36.*2.0+dQ4.*dQ5.*m6.*t3.*t4.*t7.*t17.*t36.*2.0-dQ1.*dQ2.*m6.*t4.*t5.*t10.*t22.*t33.*4.0-dQ1.*dQ3.*m6.*t4.*t5.*t10.*t22.*t32.*4.0-dQ1.*dQ4.*m6.*t5.*t6.*t11.*t17.*t33.*2.0-dQ1.*dQ5.*m5.*t3.*t4.*t8.*t25.*t32.*4.0+dQ1.*dQ5.*m6.*t3.*t4.*t8.*t20.*t36.*2.0+dQ1.*dQ6.*m6.*t4.*t5.*t9.*t20.*t32.*2.0+dQ2.*dQ6.*m6.*t2.*t5.*t8.*t20.*t34.*2.0+dQ2.*dQ6.*m6.*t3.*t5.*t7.*t20.*t34.*2.0+dQ3.*dQ5.*m6.*t2.*t3.*t9.*t20.*t35.*2.0-dQ3.*dQ6.*m6.*t2.*t5.*t8.*t17.*t36.*2.0-dQ3.*dQ6.*m6.*t3.*t5.*t7.*t17.*t36.*2.0-dQ1.*dQ2.*m5.*t4.*t5.*t10.*t25.*t32.*4.0+dQ1.*dQ2.*m6.*t4.*t5.*t10.*t20.*t36.*2.0;
et163 = dQ1.*dQ3.*m6.*t4.*t5.*t10.*t22.*t33.*-4.0-dQ1.*dQ5.*m5.*t2.*t4.*t7.*t25.*t35.*4.0-dQ1.*dQ5.*m6.*t2.*t4.*t7.*t26.*t33.*4.0-dQ1.*dQ5.*m6.*t3.*t4.*t8.*t22.*t35.*4.0+dQ1.*dQ6.*m6.*t4.*t5.*t9.*t20.*t33.*2.0-dQ2.*dQ5.*m6.*t2.*t3.*t9.*t22.*t35.*2.0+dQ3.*dQ6.*m6.*t2.*t5.*t8.*t20.*t34.*2.0+dQ3.*dQ6.*m6.*t3.*t5.*t7.*t20.*t34.*2.0-dQ4.*dQ5.*m6.*t2.*t4.*t8.*t20.*t35.*2.0-dQ4.*dQ5.*m6.*t3.*t4.*t7.*t20.*t35.*2.0-dQ1.*dQ2.*m5.*t4.*t5.*t10.*t25.*t33.*4.0-dQ1.*dQ3.*m5.*t4.*t5.*t10.*t25.*t32.*4.0+dQ1.*dQ3.*m6.*t4.*t5.*t10.*t20.*t36.*2.0+dQ1.*dQ4.*m6.*t5.*t6.*t11.*t20.*t32.*2.0-dQ1.*dQ5.*m6.*t3.*t4.*t8.*t26.*t32.*4.0+dQ2.*dQ6.*m6.*t2.*t5.*t8.*t20.*t36.*2.0+dQ2.*dQ6.*m6.*t3.*t5.*t7.*t20.*t36.*2.0-dQ3.*dQ5.*m6.*t2.*t3.*t9.*t22.*t35.*2.0;
et164 = dQ4.*dQ5.*m6.*t2.*t4.*t8.*t20.*t36.*-2.0-dQ4.*dQ5.*m6.*t3.*t4.*t7.*t20.*t36.*2.0+dQ5.*dQ6.*m6.*t2.*t3.*t10.*t17.*t36.*2.0-dQ1.*dQ2.*m6.*t4.*t5.*t10.*t26.*t32.*4.0-dQ1.*dQ3.*m5.*t4.*t5.*t10.*t25.*t33.*4.0+dQ1.*dQ4.*m6.*t5.*t6.*t11.*t20.*t33.*2.0-dQ1.*dQ5.*m5.*t3.*t4.*t8.*t25.*t35.*4.0-dQ1.*dQ5.*m6.*t2.*t4.*t7.*t26.*t35.*4.0-dQ2.*dQ5.*m5.*t2.*t3.*t9.*t25.*t35.*2.0+dQ3.*dQ6.*m6.*t2.*t5.*t8.*t20.*t36.*2.0+dQ3.*dQ6.*m6.*t3.*t5.*t7.*t20.*t36.*2.0+dQ4.*dQ5.*m6.*t2.*t4.*t8.*t22.*t35.*2.0+dQ4.*dQ5.*m6.*t3.*t4.*t7.*t22.*t35.*2.0-dQ1.*dQ2.*m6.*t4.*t5.*t10.*t26.*t33.*4.0-dQ1.*dQ3.*m6.*t4.*t5.*t10.*t26.*t32.*4.0-dQ2.*dQ5.*m5.*t7.*t8.*t9.*t16.*t35.*2.0-dQ3.*dQ5.*m5.*t2.*t3.*t9.*t25.*t35.*2.0-dQ1.*dQ3.*m6.*t4.*t5.*t10.*t26.*t33.*4.0;
et165 = dQ1.*dQ5.*m6.*t3.*t4.*t8.*t26.*t35.*-4.0-dQ2.*dQ5.*m6.*t2.*t3.*t9.*t26.*t35.*2.0-dQ3.*dQ5.*m5.*t7.*t8.*t9.*t16.*t35.*2.0+dQ4.*dQ5.*m5.*t2.*t4.*t8.*t25.*t35.*2.0+dQ4.*dQ5.*m5.*t3.*t4.*t7.*t25.*t35.*2.0-dQ5.*dQ6.*m6.*t2.*t3.*t10.*t20.*t36.*2.0-dQ3.*dQ5.*m6.*t2.*t3.*t9.*t26.*t35.*2.0+dQ4.*dQ5.*m6.*t2.*t4.*t8.*t26.*t35.*2.0+dQ4.*dQ5.*m6.*t3.*t4.*t7.*t26.*t35.*2.0-dQ2.*dQ5.*m6.*t7.*t8.*t9.*t20.*t35.*2.0-dQ3.*dQ5.*m6.*t7.*t8.*t9.*t20.*t35.*2.0+dQ2.*dQ5.*m6.*t7.*t8.*t9.*t22.*t35.*2.0+dQ3.*dQ5.*m6.*t7.*t8.*t9.*t22.*t35.*2.0-dQ5.*dQ6.*m6.*t7.*t8.*t10.*t17.*t36.*2.0+dQ2.*dQ5.*m5.*t7.*t8.*t9.*t25.*t35.*2.0+dQ3.*dQ5.*m5.*t7.*t8.*t9.*t25.*t35.*2.0-dQ1.*dQ2.*m4.*t2.*t7.*t15.*t33.*t34.*4.0+dQ2.*dQ5.*m6.*t7.*t8.*t9.*t26.*t35.*2.0+dQ5.*dQ6.*m6.*t7.*t8.*t10.*t20.*t36.*2.0;
et166 = dQ1.*dQ2.*m4.*t3.*t8.*t15.*t32.*t34.*-4.0-dQ1.*dQ3.*m4.*t2.*t7.*t15.*t33.*t34.*4.0+dQ3.*dQ5.*m6.*t7.*t8.*t9.*t26.*t35.*2.0-dQ1.*dQ3.*m4.*t3.*t8.*t15.*t32.*t34.*4.0+dQ1.*dQ2.*m4.*t2.*t7.*t18.*t33.*t34.*4.0-dQ1.*dQ2.*m5.*t2.*t7.*t16.*t33.*t35.*4.0+dQ1.*dQ2.*m4.*t3.*t8.*t18.*t32.*t34.*4.0+dQ1.*dQ2.*m5.*t2.*t7.*t16.*t34.*t35.*2.0-dQ1.*dQ2.*m5.*t3.*t8.*t16.*t32.*t35.*4.0+dQ1.*dQ2.*m6.*t2.*t7.*t17.*t33.*t34.*4.0+dQ1.*dQ3.*m4.*t2.*t7.*t18.*t33.*t34.*4.0-dQ1.*dQ3.*m5.*t2.*t7.*t16.*t33.*t35.*4.0-dQ1.*dQ4.*m4.*t4.*t9.*t15.*t32.*t33.*4.0+dQ1.*dQ2.*m5.*t2.*t7.*t19.*t33.*t34.*4.0+dQ1.*dQ2.*m6.*t3.*t8.*t17.*t32.*t34.*4.0+dQ1.*dQ3.*m4.*t3.*t8.*t18.*t32.*t34.*4.0+dQ1.*dQ3.*m5.*t2.*t7.*t16.*t34.*t35.*2.0-dQ1.*dQ3.*m5.*t3.*t8.*t16.*t32.*t35.*4.0+dQ1.*dQ3.*m6.*t2.*t7.*t17.*t33.*t34.*4.0;
et167 = dQ1.*dQ2.*m5.*t3.*t8.*t16.*t34.*t35.*2.0+dQ1.*dQ2.*m5.*t3.*t8.*t19.*t32.*t34.*4.0+dQ1.*dQ2.*m6.*t2.*t7.*t17.*t33.*t36.*8.0+dQ1.*dQ3.*m5.*t2.*t7.*t19.*t33.*t34.*4.0+dQ1.*dQ3.*m6.*t3.*t8.*t17.*t32.*t34.*4.0+dQ1.*dQ2.*m6.*t2.*t7.*t17.*t34.*t36.*2.0+dQ1.*dQ2.*m6.*t3.*t8.*t17.*t32.*t36.*8.0+dQ1.*dQ3.*m5.*t3.*t8.*t16.*t34.*t35.*2.0+dQ1.*dQ3.*m5.*t3.*t8.*t19.*t32.*t34.*4.0+dQ1.*dQ3.*m6.*t2.*t7.*t17.*t33.*t36.*8.0+dQ1.*dQ4.*m4.*t4.*t9.*t18.*t32.*t33.*4.0+dQ1.*dQ2.*m6.*t2.*t7.*t17.*t35.*t36.*2.0-dQ1.*dQ2.*m6.*t2.*t7.*t20.*t33.*t35.*4.0+dQ1.*dQ3.*m6.*t2.*t7.*t17.*t34.*t36.*2.0+dQ1.*dQ3.*m6.*t3.*t8.*t17.*t32.*t36.*8.0+dQ1.*dQ4.*m5.*t4.*t9.*t16.*t32.*t35.*2.0+dQ1.*dQ4.*m6.*t4.*t9.*t17.*t32.*t33.*4.0+dQ2.*dQ4.*m5.*t2.*t8.*t16.*t34.*t35.*2.0+dQ2.*dQ4.*m5.*t3.*t7.*t16.*t34.*t35.*2.0;
et168 = dQ1.*dQ2.*m6.*t2.*t7.*t20.*t33.*t36.*-8.0+dQ1.*dQ2.*m6.*t2.*t7.*t20.*t34.*t35.*2.0-dQ1.*dQ2.*m6.*t2.*t7.*t22.*t33.*t34.*4.0+dQ1.*dQ2.*m6.*t3.*t8.*t17.*t34.*t36.*2.0-dQ1.*dQ2.*m6.*t3.*t8.*t20.*t32.*t35.*4.0+dQ1.*dQ3.*m6.*t2.*t7.*t17.*t35.*t36.*2.0-dQ1.*dQ3.*m6.*t2.*t7.*t20.*t33.*t35.*4.0+dQ1.*dQ4.*m5.*t4.*t9.*t16.*t33.*t35.*2.0+dQ1.*dQ4.*m5.*t4.*t9.*t19.*t32.*t33.*4.0-dQ1.*dQ5.*m5.*t5.*t10.*t16.*t32.*t33.*4.0+dQ3.*dQ4.*m5.*t2.*t8.*t16.*t34.*t35.*2.0+dQ3.*dQ4.*m5.*t3.*t7.*t16.*t34.*t35.*2.0-dQ1.*dQ2.*m6.*t2.*t7.*t20.*t34.*t36.*2.0+dQ1.*dQ2.*m6.*t2.*t7.*t22.*t33.*t35.*4.0+dQ1.*dQ2.*m6.*t3.*t8.*t17.*t35.*t36.*2.0-dQ1.*dQ2.*m6.*t3.*t8.*t20.*t32.*t36.*8.0-dQ1.*dQ2.*m6.*t3.*t8.*t22.*t32.*t34.*4.0-dQ1.*dQ3.*m6.*t2.*t7.*t20.*t33.*t36.*8.0;
et169 = dQ1.*dQ3.*m6.*t2.*t7.*t20.*t34.*t35.*2.0-dQ1.*dQ3.*m6.*t2.*t7.*t22.*t33.*t34.*4.0+dQ1.*dQ3.*m6.*t3.*t8.*t17.*t34.*t36.*2.0-dQ1.*dQ3.*m6.*t3.*t8.*t20.*t32.*t35.*4.0+dQ1.*dQ5.*m5.*t5.*t10.*t16.*t32.*t34.*2.0-dQ1.*dQ2.*m5.*t2.*t7.*t25.*t33.*t34.*4.0-dQ1.*dQ2.*m6.*t2.*t7.*t20.*t35.*t36.*2.0-dQ1.*dQ2.*m6.*t2.*t7.*t22.*t34.*t35.*2.0+dQ1.*dQ2.*m6.*t3.*t8.*t20.*t34.*t35.*2.0+dQ1.*dQ2.*m6.*t3.*t8.*t22.*t32.*t35.*4.0-dQ1.*dQ3.*m6.*t2.*t7.*t20.*t34.*t36.*2.0+dQ1.*dQ3.*m6.*t2.*t7.*t22.*t33.*t35.*4.0+dQ1.*dQ3.*m6.*t3.*t8.*t17.*t35.*t36.*2.0-dQ1.*dQ3.*m6.*t3.*t8.*t20.*t32.*t36.*8.0-dQ1.*dQ3.*m6.*t3.*t8.*t22.*t32.*t34.*4.0+dQ1.*dQ4.*m6.*t4.*t9.*t17.*t32.*t36.*2.0+dQ1.*dQ5.*m5.*t5.*t10.*t16.*t33.*t34.*2.0+dQ2.*dQ4.*m6.*t2.*t8.*t17.*t34.*t36.*2.0+dQ2.*dQ4.*m6.*t3.*t7.*t17.*t34.*t36.*2.0;
et170 = dQ1.*dQ2.*m5.*t2.*t7.*t25.*t33.*t35.*4.0-dQ1.*dQ2.*m5.*t3.*t8.*t25.*t32.*t34.*4.0-dQ1.*dQ2.*m6.*t3.*t8.*t20.*t34.*t36.*2.0-dQ1.*dQ3.*m5.*t2.*t7.*t25.*t33.*t34.*4.0-dQ1.*dQ3.*m6.*t2.*t7.*t20.*t35.*t36.*2.0-dQ1.*dQ3.*m6.*t2.*t7.*t22.*t34.*t35.*2.0+dQ1.*dQ3.*m6.*t3.*t8.*t20.*t34.*t35.*2.0+dQ1.*dQ3.*m6.*t3.*t8.*t22.*t32.*t35.*4.0+dQ1.*dQ4.*m6.*t4.*t9.*t17.*t33.*t36.*2.0-dQ2.*dQ4.*m6.*t2.*t8.*t17.*t35.*t36.*2.0-dQ2.*dQ4.*m6.*t3.*t7.*t17.*t35.*t36.*2.0+dQ3.*dQ4.*m6.*t2.*t8.*t17.*t34.*t36.*2.0+dQ3.*dQ4.*m6.*t3.*t7.*t17.*t34.*t36.*2.0-dQ1.*dQ2.*m5.*t2.*t7.*t25.*t34.*t35.*2.0+dQ1.*dQ2.*m5.*t3.*t8.*t25.*t32.*t35.*4.0-dQ1.*dQ2.*m6.*t2.*t7.*t26.*t33.*t34.*4.0-dQ1.*dQ2.*m6.*t3.*t8.*t20.*t35.*t36.*2.0-dQ1.*dQ2.*m6.*t3.*t8.*t22.*t34.*t35.*2.0;
et171 = dQ1.*dQ3.*m5.*t2.*t7.*t25.*t33.*t35.*4.0-dQ1.*dQ3.*m5.*t3.*t8.*t25.*t32.*t34.*4.0-dQ1.*dQ3.*m6.*t3.*t8.*t20.*t34.*t36.*2.0+dQ1.*dQ4.*m6.*t4.*t9.*t20.*t32.*t35.*2.0-dQ1.*dQ4.*m6.*t4.*t9.*t22.*t32.*t33.*4.0+dQ2.*dQ4.*m6.*t2.*t8.*t20.*t34.*t35.*2.0+dQ2.*dQ4.*m6.*t3.*t7.*t20.*t34.*t35.*2.0-dQ3.*dQ4.*m6.*t2.*t8.*t17.*t35.*t36.*2.0-dQ3.*dQ4.*m6.*t3.*t7.*t17.*t35.*t36.*2.0+dQ1.*dQ2.*m6.*t2.*t7.*t26.*t33.*t35.*4.0-dQ1.*dQ2.*m6.*t3.*t8.*t26.*t32.*t34.*4.0-dQ1.*dQ3.*m5.*t2.*t7.*t25.*t34.*t35.*2.0+dQ1.*dQ3.*m5.*t3.*t8.*t25.*t32.*t35.*4.0-dQ1.*dQ3.*m6.*t2.*t7.*t26.*t33.*t34.*4.0-dQ1.*dQ3.*m6.*t3.*t8.*t20.*t35.*t36.*2.0-dQ1.*dQ3.*m6.*t3.*t8.*t22.*t34.*t35.*2.0-dQ1.*dQ4.*m6.*t4.*t9.*t20.*t32.*t36.*2.0+dQ1.*dQ4.*m6.*t4.*t9.*t20.*t33.*t35.*2.0;
et172 = dQ1.*dQ5.*m6.*t5.*t10.*t17.*t32.*t36.*2.0-dQ1.*dQ5.*m6.*t5.*t10.*t20.*t32.*t33.*4.0+dQ1.*dQ6.*m6.*t6.*t11.*t17.*t32.*t33.*8.0-dQ2.*dQ4.*m6.*t2.*t8.*t20.*t34.*t36.*2.0-dQ2.*dQ4.*m6.*t3.*t7.*t20.*t34.*t36.*2.0+dQ3.*dQ4.*m6.*t2.*t8.*t20.*t34.*t35.*2.0+dQ3.*dQ4.*m6.*t3.*t7.*t20.*t34.*t35.*2.0-dQ1.*dQ2.*m5.*t3.*t8.*t25.*t34.*t35.*2.0-dQ1.*dQ2.*m6.*t2.*t7.*t26.*t34.*t35.*2.0+dQ1.*dQ2.*m6.*t3.*t8.*t26.*t32.*t35.*4.0+dQ1.*dQ3.*m6.*t2.*t7.*t26.*t33.*t35.*4.0-dQ1.*dQ3.*m6.*t3.*t8.*t26.*t32.*t34.*4.0-dQ1.*dQ4.*m5.*t4.*t9.*t25.*t32.*t33.*4.0-dQ1.*dQ4.*m6.*t4.*t9.*t20.*t33.*t36.*2.0-dQ1.*dQ4.*m6.*t4.*t9.*t22.*t32.*t35.*2.0+dQ1.*dQ5.*m6.*t5.*t10.*t17.*t33.*t36.*2.0+dQ1.*dQ5.*m6.*t5.*t10.*t20.*t32.*t34.*2.0+dQ1.*dQ6.*m6.*t6.*t11.*t17.*t32.*t34.*2.0+dQ2.*dQ4.*m6.*t2.*t8.*t20.*t35.*t36.*2.0;
et173 = dQ2.*dQ4.*m6.*t2.*t8.*t22.*t34.*t35.*-2.0+dQ2.*dQ4.*m6.*t3.*t7.*t20.*t35.*t36.*2.0-dQ2.*dQ4.*m6.*t3.*t7.*t22.*t34.*t35.*2.0-dQ3.*dQ4.*m6.*t2.*t8.*t20.*t34.*t36.*2.0-dQ3.*dQ4.*m6.*t3.*t7.*t20.*t34.*t36.*2.0-dQ1.*dQ3.*m5.*t3.*t8.*t25.*t34.*t35.*2.0-dQ1.*dQ3.*m6.*t2.*t7.*t26.*t34.*t35.*2.0+dQ1.*dQ3.*m6.*t3.*t8.*t26.*t32.*t35.*4.0-dQ1.*dQ4.*m6.*t4.*t9.*t22.*t33.*t35.*2.0+dQ1.*dQ5.*m6.*t5.*t10.*t20.*t33.*t34.*2.0+dQ1.*dQ5.*m6.*t5.*t10.*t22.*t32.*t33.*4.0+dQ1.*dQ6.*m6.*t6.*t11.*t17.*t32.*t35.*2.0+dQ1.*dQ6.*m6.*t6.*t11.*t17.*t33.*t34.*2.0+dQ3.*dQ4.*m6.*t2.*t8.*t20.*t35.*t36.*2.0-dQ3.*dQ4.*m6.*t2.*t8.*t22.*t34.*t35.*2.0+dQ3.*dQ4.*m6.*t3.*t7.*t20.*t35.*t36.*2.0-dQ3.*dQ4.*m6.*t3.*t7.*t22.*t34.*t35.*2.0-dQ1.*dQ2.*m6.*t3.*t8.*t26.*t34.*t35.*2.0;
et174 = dQ1.*dQ4.*m5.*t4.*t9.*t25.*t32.*t35.*-2.0-dQ1.*dQ4.*m6.*t4.*t9.*t26.*t32.*t33.*4.0-dQ1.*dQ5.*m6.*t5.*t10.*t20.*t32.*t36.*2.0-dQ1.*dQ5.*m6.*t5.*t10.*t22.*t32.*t34.*2.0+dQ1.*dQ6.*m6.*t6.*t11.*t17.*t33.*t35.*2.0-dQ1.*dQ6.*m6.*t6.*t11.*t20.*t32.*t33.*8.0-dQ2.*dQ4.*m5.*t2.*t8.*t25.*t34.*t35.*2.0-dQ2.*dQ4.*m5.*t3.*t7.*t25.*t34.*t35.*2.0-dQ1.*dQ3.*m6.*t3.*t8.*t26.*t34.*t35.*2.0-dQ1.*dQ4.*m5.*t4.*t9.*t25.*t33.*t35.*2.0+dQ1.*dQ5.*m5.*t5.*t10.*t25.*t32.*t33.*4.0-dQ1.*dQ5.*m6.*t5.*t10.*t20.*t33.*t36.*2.0-dQ1.*dQ5.*m6.*t5.*t10.*t22.*t33.*t34.*2.0-dQ1.*dQ6.*m6.*t6.*t11.*t20.*t32.*t34.*2.0-dQ3.*dQ4.*m5.*t2.*t8.*t25.*t34.*t35.*2.0-dQ3.*dQ4.*m5.*t3.*t7.*t25.*t34.*t35.*2.0-dQ1.*dQ4.*m6.*t4.*t9.*t26.*t32.*t35.*2.0-dQ1.*dQ5.*m5.*t5.*t10.*t25.*t32.*t34.*2.0;
et175 = dQ1.*dQ6.*m6.*t6.*t11.*t20.*t32.*t35.*-2.0-dQ1.*dQ6.*m6.*t6.*t11.*t20.*t33.*t34.*2.0-dQ2.*dQ4.*m6.*t2.*t8.*t26.*t34.*t35.*2.0-dQ2.*dQ4.*m6.*t3.*t7.*t26.*t34.*t35.*2.0-dQ1.*dQ4.*m6.*t4.*t9.*t26.*t33.*t35.*2.0-dQ1.*dQ5.*m5.*t5.*t10.*t25.*t33.*t34.*2.0+dQ1.*dQ5.*m6.*t5.*t10.*t26.*t32.*t33.*4.0-dQ1.*dQ6.*m6.*t6.*t11.*t20.*t33.*t35.*2.0-dQ3.*dQ4.*m6.*t2.*t8.*t26.*t34.*t35.*2.0-dQ3.*dQ4.*m6.*t3.*t7.*t26.*t34.*t35.*2.0-dQ1.*dQ5.*m6.*t5.*t10.*t26.*t32.*t34.*2.0-dQ1.*dQ5.*m6.*t5.*t10.*t26.*t33.*t34.*2.0-Ixx6.*dQ2.*dQ5.*t2.*t3.*t4.*t5.*t6.*t11.*2.0-Ixx6.*dQ3.*dQ5.*t2.*t3.*t4.*t5.*t6.*t11.*2.0-Ixx5.*dQ1.*dQ5.*t2.*t3.*t5.*t7.*t8.*t10.*4.0+Ixx5.*dQ2.*dQ5.*t2.*t4.*t5.*t8.*t9.*t10.*2.0+Ixx5.*dQ2.*dQ5.*t3.*t4.*t5.*t7.*t9.*t10.*2.0;
et176 = Ixx6.*dQ1.*dQ6.*t2.*t3.*t6.*t7.*t8.*t11.*8.0+Ixx5.*dQ3.*dQ5.*t2.*t4.*t5.*t8.*t9.*t10.*2.0+Ixx5.*dQ3.*dQ5.*t3.*t4.*t5.*t7.*t9.*t10.*2.0+Ixx6.*dQ1.*dQ4.*t2.*t4.*t6.*t7.*t10.*t11.*2.0+Ixx6.*dQ1.*dQ5.*t2.*t5.*t6.*t7.*t9.*t11.*2.0+Ixx6.*dQ2.*dQ3.*t2.*t4.*t6.*t8.*t10.*t11.*2.0+Ixx6.*dQ2.*dQ3.*t3.*t4.*t6.*t7.*t10.*t11.*2.0+Ixx6.*dQ1.*dQ4.*t3.*t4.*t6.*t8.*t10.*t11.*2.0+Ixx6.*dQ1.*dQ5.*t3.*t5.*t6.*t8.*t9.*t11.*2.0+Ixx6.*dQ2.*dQ5.*t4.*t5.*t6.*t7.*t8.*t11.*2.0+Ixx6.*dQ2.*dQ6.*t2.*t4.*t6.*t8.*t9.*t11.*2.0+Ixx6.*dQ2.*dQ6.*t3.*t4.*t6.*t7.*t9.*t11.*2.0+Ixx6.*dQ3.*dQ5.*t4.*t5.*t6.*t7.*t8.*t11.*2.0+Ixx6.*dQ3.*dQ6.*t2.*t4.*t6.*t8.*t9.*t11.*2.0+Ixx6.*dQ3.*dQ6.*t3.*t4.*t6.*t7.*t9.*t11.*2.0-Ixx6.*dQ2.*dQ3.*t2.*t3.*t5.*t6.*t11.*t34.*4.0-Ixx5.*dQ1.*dQ4.*t2.*t5.*t7.*t9.*t10.*t33.*4.0;
et177 = Ixx5.*dQ1.*dQ4.*t3.*t5.*t8.*t9.*t10.*t32.*-4.0+Ixx6.*dQ1.*dQ4.*t2.*t5.*t7.*t9.*t10.*t36.*2.0+Ixx6.*dQ2.*dQ3.*t2.*t5.*t8.*t9.*t10.*t36.*2.0+Ixx6.*dQ2.*dQ3.*t3.*t5.*t7.*t9.*t10.*t36.*2.0+Ixx6.*dQ1.*dQ4.*t3.*t5.*t8.*t9.*t10.*t36.*2.0+Ixx6.*dQ2.*dQ3.*t5.*t6.*t7.*t8.*t11.*t34.*4.0+Ixx6.*dQ1.*dQ5.*t4.*t6.*t9.*t10.*t11.*t32.*2.0+Ixx6.*dQ2.*dQ5.*t2.*t6.*t8.*t10.*t11.*t34.*2.0+Ixx6.*dQ2.*dQ5.*t3.*t6.*t7.*t10.*t11.*t34.*2.0+Ixx6.*dQ1.*dQ5.*t4.*t6.*t9.*t10.*t11.*t33.*2.0+Ixx6.*dQ3.*dQ5.*t2.*t6.*t8.*t10.*t11.*t34.*2.0+Ixx6.*dQ3.*dQ5.*t3.*t6.*t7.*t10.*t11.*t34.*2.0-Ixx6.*dQ2.*dQ3.*t2.*t3.*t4.*t9.*t35.*t36.*2.0-Ixx6.*dQ1.*dQ2.*t6.*t9.*t10.*t11.*t32.*t33.*8.0-Ixx6.*dQ1.*dQ6.*t2.*t7.*t9.*t10.*t33.*t36.*8.0+Ixx6.*dQ2.*dQ3.*t4.*t7.*t8.*t9.*t35.*t36.*2.0-Ixx6.*dQ1.*dQ3.*t6.*t9.*t10.*t11.*t32.*t33.*8.0;
et178 = Ixx6.*dQ1.*dQ6.*t3.*t8.*t9.*t10.*t32.*t36.*-8.0+Ixx6.*dQ1.*dQ2.*t4.*t5.*t10.*t32.*t33.*t36.*8.0+Ixx6.*dQ1.*dQ5.*t2.*t4.*t7.*t33.*t35.*t36.*8.0+Ixx6.*dQ1.*dQ3.*t4.*t5.*t10.*t32.*t33.*t36.*8.0+Ixx6.*dQ1.*dQ5.*t3.*t4.*t8.*t32.*t35.*t36.*8.0+Ixx6.*dQ1.*dQ4.*t5.*t6.*t11.*t32.*t33.*t34.*8.0+Ixx6.*dQ1.*dQ6.*t4.*t5.*t9.*t32.*t33.*t36.*8.0+Ixx6.*dQ1.*dQ2.*t2.*t7.*t33.*t34.*t35.*t36.*4.0+Ixx6.*dQ1.*dQ2.*t3.*t8.*t32.*t34.*t35.*t36.*4.0+Ixx6.*dQ1.*dQ3.*t2.*t7.*t33.*t34.*t35.*t36.*4.0+Ixx6.*dQ1.*dQ3.*t3.*t8.*t32.*t34.*t35.*t36.*4.0+Ixx6.*dQ1.*dQ4.*t4.*t9.*t32.*t33.*t35.*t36.*4.0+Ixx6.*dQ1.*dQ5.*t5.*t10.*t32.*t33.*t34.*t36.*4.0+Ixx6.*dQ1.*dQ6.*t6.*t11.*t32.*t33.*t34.*t35.*4.0-Ixy6.*dQ2.*dQ3.*t2.*t3.*t4.*t6.*t9.*t11.*2.0-Ixy5.*dQ1.*dQ2.*t2.*t3.*t7.*t8.*t9.*t10.*4.0-Ixy5.*dQ1.*dQ3.*t2.*t3.*t7.*t8.*t9.*t10.*4.0;
et179 = Ixy6.*dQ1.*dQ2.*t2.*t3.*t7.*t8.*t9.*t10.*4.0+Ixy6.*dQ1.*dQ3.*t2.*t3.*t7.*t8.*t9.*t10.*4.0-Ixy6.*dQ2.*dQ6.*t2.*t3.*t4.*t6.*t10.*t11.*2.0-Ixy6.*dQ3.*dQ6.*t2.*t3.*t4.*t6.*t10.*t11.*2.0+Ixy6.*dQ4.*dQ5.*t2.*t3.*t5.*t6.*t10.*t11.*2.0+Ixy6.*dQ2.*dQ3.*t4.*t6.*t7.*t8.*t9.*t11.*2.0+Ixy6.*dQ1.*dQ6.*t2.*t6.*t7.*t9.*t10.*t11.*4.0+Ixy6.*dQ1.*dQ6.*t3.*t6.*t8.*t9.*t10.*t11.*4.0+Ixy6.*dQ2.*dQ6.*t4.*t6.*t7.*t8.*t10.*t11.*2.0+Ixy6.*dQ3.*dQ6.*t4.*t6.*t7.*t8.*t10.*t11.*2.0-Ixy6.*dQ4.*dQ5.*t5.*t6.*t7.*t8.*t10.*t11.*2.0-Ixy6.*dQ4.*dQ6.*t2.*t6.*t8.*t9.*t10.*t11.*2.0-Ixy6.*dQ4.*dQ6.*t3.*t6.*t7.*t9.*t10.*t11.*2.0+Ixy5.*dQ1.*dQ2.*t2.*t4.*t5.*t7.*t9.*t33.*4.0+Ixy5.*dQ1.*dQ2.*t3.*t4.*t5.*t8.*t9.*t32.*4.0+Ixy5.*dQ1.*dQ3.*t2.*t4.*t5.*t7.*t9.*t33.*4.0+Ixy5.*dQ1.*dQ4.*t2.*t3.*t5.*t7.*t8.*t34.*4.0;
et180 = Ixy6.*dQ1.*dQ2.*t2.*t4.*t5.*t7.*t9.*t33.*-4.0+Ixy5.*dQ1.*dQ3.*t3.*t4.*t5.*t8.*t9.*t32.*4.0-Ixy6.*dQ1.*dQ2.*t3.*t4.*t5.*t8.*t9.*t32.*4.0-Ixy6.*dQ1.*dQ3.*t2.*t4.*t5.*t7.*t9.*t33.*4.0-Ixy6.*dQ1.*dQ4.*t2.*t3.*t5.*t7.*t8.*t34.*4.0-Ixy6.*dQ1.*dQ3.*t3.*t4.*t5.*t8.*t9.*t32.*4.0-Ixy6.*dQ1.*dQ2.*t2.*t4.*t5.*t7.*t9.*t36.*4.0-Ixy6.*dQ1.*dQ4.*t2.*t3.*t5.*t7.*t8.*t36.*4.0-Ixy6.*dQ1.*dQ3.*t2.*t4.*t5.*t7.*t9.*t36.*4.0-Ixy6.*dQ1.*dQ2.*t3.*t4.*t5.*t8.*t9.*t36.*4.0-Ixy6.*dQ1.*dQ6.*t2.*t4.*t5.*t7.*t10.*t33.*4.0-Ixy6.*dQ1.*dQ3.*t3.*t4.*t5.*t8.*t9.*t36.*4.0-Ixy6.*dQ1.*dQ5.*t2.*t4.*t6.*t7.*t11.*t33.*4.0-Ixy6.*dQ1.*dQ6.*t3.*t4.*t5.*t8.*t10.*t32.*4.0-Ixy6.*dQ1.*dQ5.*t3.*t4.*t6.*t8.*t11.*t32.*4.0-Ixy6.*dQ1.*dQ2.*t4.*t5.*t6.*t10.*t11.*t32.*4.0;
et181 = Ixy6.*dQ1.*dQ5.*t2.*t4.*t6.*t7.*t11.*t35.*-4.0-Ixy6.*dQ1.*dQ6.*t2.*t4.*t5.*t7.*t10.*t36.*4.0-Ixy6.*dQ1.*dQ2.*t4.*t5.*t6.*t10.*t11.*t33.*4.0-Ixy6.*dQ1.*dQ3.*t4.*t5.*t6.*t10.*t11.*t32.*4.0-Ixy6.*dQ1.*dQ3.*t4.*t5.*t6.*t10.*t11.*t33.*4.0-Ixy6.*dQ1.*dQ5.*t3.*t4.*t6.*t8.*t11.*t35.*4.0-Ixy6.*dQ1.*dQ6.*t3.*t4.*t5.*t8.*t10.*t36.*4.0-Ixy6.*dQ2.*dQ5.*t2.*t3.*t6.*t9.*t11.*t35.*2.0-Ixy6.*dQ2.*dQ6.*t2.*t3.*t5.*t9.*t10.*t36.*2.0-Ixy6.*dQ1.*dQ6.*t4.*t5.*t6.*t9.*t11.*t32.*4.0-Ixy6.*dQ3.*dQ5.*t2.*t3.*t6.*t9.*t11.*t35.*2.0-Ixy6.*dQ3.*dQ6.*t2.*t3.*t5.*t9.*t10.*t36.*2.0-Ixy6.*dQ1.*dQ6.*t4.*t5.*t6.*t9.*t11.*t33.*4.0+Ixy6.*dQ4.*dQ5.*t2.*t4.*t6.*t8.*t11.*t35.*2.0+Ixy6.*dQ4.*dQ5.*t3.*t4.*t6.*t7.*t11.*t35.*2.0+Ixy6.*dQ4.*dQ6.*t2.*t4.*t5.*t8.*t10.*t36.*2.0+Ixy6.*dQ4.*dQ6.*t3.*t4.*t5.*t7.*t10.*t36.*2.0;
et182 = Ixy6.*dQ2.*dQ5.*t6.*t7.*t8.*t9.*t11.*t35.*2.0+Ixy6.*dQ2.*dQ6.*t5.*t7.*t8.*t9.*t10.*t36.*2.0+Ixy6.*dQ3.*dQ5.*t6.*t7.*t8.*t9.*t11.*t35.*2.0+Ixy6.*dQ3.*dQ6.*t5.*t7.*t8.*t9.*t10.*t36.*2.0+Ixy6.*dQ1.*dQ2.*t2.*t6.*t7.*t11.*t33.*t34.*4.0-Ixy6.*dQ1.*dQ6.*t2.*t3.*t7.*t8.*t34.*t35.*2.0+Ixy6.*dQ1.*dQ2.*t2.*t6.*t7.*t11.*t33.*t35.*4.0+Ixy6.*dQ1.*dQ2.*t3.*t6.*t8.*t11.*t32.*t34.*4.0+Ixy6.*dQ1.*dQ3.*t2.*t6.*t7.*t11.*t33.*t34.*4.0+Ixy6.*dQ1.*dQ4.*t2.*t4.*t7.*t10.*t33.*t36.*4.0+Ixy6.*dQ1.*dQ6.*t2.*t3.*t7.*t8.*t34.*t36.*4.0-Ixy6.*dQ1.*dQ2.*t2.*t6.*t7.*t11.*t34.*t35.*2.0+Ixy6.*dQ1.*dQ2.*t3.*t6.*t8.*t11.*t32.*t35.*4.0+Ixy6.*dQ1.*dQ3.*t2.*t6.*t7.*t11.*t33.*t35.*4.0+Ixy6.*dQ1.*dQ3.*t3.*t6.*t8.*t11.*t32.*t34.*4.0+Ixy6.*dQ1.*dQ4.*t3.*t4.*t8.*t10.*t32.*t36.*4.0+Ixy6.*dQ1.*dQ5.*t2.*t5.*t7.*t9.*t33.*t36.*4.0+Ixy6.*dQ1.*dQ6.*t2.*t3.*t7.*t8.*t35.*t36.*4.0;
et183 = Ixy6.*dQ1.*dQ3.*t2.*t6.*t7.*t11.*t34.*t35.*-2.0+Ixy6.*dQ1.*dQ3.*t3.*t6.*t8.*t11.*t32.*t35.*4.0+Ixy6.*dQ1.*dQ5.*t3.*t5.*t8.*t9.*t32.*t36.*4.0-Ixy6.*dQ1.*dQ2.*t3.*t6.*t8.*t11.*t34.*t35.*2.0+Ixy6.*dQ1.*dQ4.*t4.*t6.*t9.*t11.*t32.*t33.*4.0-Ixy6.*dQ1.*dQ3.*t3.*t6.*t8.*t11.*t34.*t35.*2.0-Ixy6.*dQ1.*dQ4.*t4.*t6.*t9.*t11.*t32.*t35.*2.0-Ixy6.*dQ2.*dQ4.*t2.*t6.*t8.*t11.*t34.*t35.*2.0-Ixy6.*dQ2.*dQ4.*t3.*t6.*t7.*t11.*t34.*t35.*2.0-Ixy6.*dQ1.*dQ4.*t4.*t6.*t9.*t11.*t33.*t35.*2.0+Ixy6.*dQ1.*dQ5.*t5.*t6.*t10.*t11.*t32.*t33.*4.0-Ixy6.*dQ3.*dQ4.*t2.*t6.*t8.*t11.*t34.*t35.*2.0-Ixy6.*dQ3.*dQ4.*t3.*t6.*t7.*t11.*t34.*t35.*2.0-Ixy6.*dQ1.*dQ5.*t5.*t6.*t10.*t11.*t32.*t34.*2.0-Ixy6.*dQ1.*dQ5.*t5.*t6.*t10.*t11.*t33.*t34.*2.0+Ixy6.*dQ1.*dQ5.*t4.*t9.*t10.*t32.*t33.*t36.*4.0+Ixz6.*dQ1.*dQ2.*t2.*t3.*t4.*t6.*t7.*t8.*4.0;
et184 = Ixz6.*dQ1.*dQ3.*t2.*t3.*t4.*t6.*t7.*t8.*4.0+Ixz5.*dQ2.*dQ3.*t2.*t3.*t4.*t5.*t9.*t10.*2.0+Ixz6.*dQ1.*dQ5.*t2.*t4.*t5.*t6.*t7.*t10.*4.0+Ixz6.*dQ1.*dQ5.*t3.*t4.*t5.*t6.*t8.*t10.*4.0-Ixz6.*dQ4.*dQ5.*t2.*t4.*t5.*t6.*t8.*t10.*2.0-Ixz6.*dQ4.*dQ5.*t3.*t4.*t5.*t6.*t7.*t10.*2.0-Ixz6.*dQ1.*dQ2.*t2.*t4.*t7.*t9.*t10.*t11.*2.0-Ixz6.*dQ1.*dQ4.*t2.*t3.*t7.*t8.*t10.*t11.*2.0-Ixz5.*dQ2.*dQ3.*t4.*t5.*t7.*t8.*t9.*t10.*2.0-Ixz6.*dQ1.*dQ3.*t2.*t4.*t7.*t9.*t10.*t11.*2.0-Ixz6.*dQ1.*dQ2.*t3.*t4.*t8.*t9.*t10.*t11.*2.0-Ixz6.*dQ1.*dQ3.*t3.*t4.*t8.*t9.*t10.*t11.*2.0-Ixz5.*dQ1.*dQ2.*t2.*t3.*t4.*t7.*t8.*t35.*8.0-Ixz5.*dQ1.*dQ3.*t2.*t3.*t4.*t7.*t8.*t35.*8.0-Ixz5.*dQ1.*dQ5.*t2.*t4.*t5.*t7.*t10.*t33.*8.0-Ixz6.*dQ1.*dQ2.*t2.*t5.*t6.*t7.*t10.*t33.*4.0;
et185 = Ixz6.*dQ1.*dQ5.*t2.*t3.*t6.*t7.*t8.*t34.*2.0-Ixz5.*dQ1.*dQ5.*t3.*t4.*t5.*t8.*t10.*t32.*8.0+Ixz6.*dQ1.*dQ2.*t2.*t5.*t6.*t7.*t10.*t34.*2.0-Ixz6.*dQ1.*dQ2.*t3.*t5.*t6.*t8.*t10.*t32.*4.0-Ixz6.*dQ1.*dQ3.*t2.*t5.*t6.*t7.*t10.*t33.*4.0-Ixz6.*dQ1.*dQ4.*t2.*t4.*t5.*t7.*t11.*t33.*2.0-Ixz6.*dQ1.*dQ5.*t2.*t3.*t6.*t7.*t8.*t35.*4.0+Ixz6.*dQ1.*dQ3.*t2.*t5.*t6.*t7.*t10.*t34.*2.0-Ixz6.*dQ1.*dQ3.*t3.*t5.*t6.*t8.*t10.*t32.*4.0-Ixz6.*dQ1.*dQ4.*t3.*t4.*t5.*t8.*t11.*t32.*2.0+Ixz6.*dQ1.*dQ2.*t3.*t5.*t6.*t8.*t10.*t34.*2.0-Ixz6.*dQ1.*dQ6.*t2.*t5.*t6.*t7.*t9.*t33.*2.0+Ixz6.*dQ1.*dQ3.*t3.*t5.*t6.*t8.*t10.*t34.*2.0-Ixz6.*dQ1.*dQ6.*t3.*t5.*t6.*t8.*t9.*t32.*2.0+Ixz6.*dQ1.*dQ4.*t4.*t5.*t6.*t9.*t10.*t32.*2.0+Ixz6.*dQ2.*dQ4.*t2.*t5.*t6.*t8.*t10.*t34.*2.0+Ixz6.*dQ2.*dQ4.*t3.*t5.*t6.*t7.*t10.*t34.*2.0;
